simulink model "simulator_prototype"  (R2021b)
(part 7 of 12)

t5255 = t4765.*(-t1901+t3122+t3277);
t5262 = -t3893.*(t4165+t27.*(t1959-t3313+t38.*t1022.*(t855-t878).*2.196325630278387e-1));
t5280 = t3937.*t4834.*7.26735e-3;
t5281 = t4834.*(t1959-t3313+t38.*t1022.*(t855-t878).*2.196325630278387e-1).*(-7.26735e-3);
t5292 = -t5287;
t5300 = -t5297;
t5310 = t4118.*t4814;
t5320 = t4137+t4842;
t5321 = t4142+t4841;
t5356 = t4151.*t4853.*7.26735e-3;
t5357 = t4853.*(t1005+t20.*(t1941-t3315+t39.*t1022.*(t855-t878).*2.196325630278387e-1)).*(-7.26735e-3);
t5415 = (t4360.*t4879)./2.0;
et50 = -t2306-t2317+t3145+t3148+t35.*t941.*t948.*(t850-t874).*3.775747223193135e-1;
et51 = t36.*t941.*t948.*(t850-t874).*2.244797987218524e-1;
t5416 = ((et50+et51).*(-t3538+t3540+t50.*t188.*t202.*(t46-t47).*2.711709361697228e-39))./2.0;
t5487 = t3755.*t3910.*t3934.*t4172.*5.43845e-3;
t5488 = t3755.*t4172.*(t2674-t2676+t3022-t3027).*(t2694-t2701+t3036-t3043).*5.43845e-3;
t5494 = t3712.*t3910.*t3934.*t4215.*5.43845e-3;
t5495 = t3712.*t4215.*(t2674-t2676+t3022-t3027).*(t2694-t2701+t3036-t3043).*5.43845e-3;
t5535 = t3810.*t3910.*t3934.*t4172.*5.43845e-3;
t5536 = t3810.*t4172.*(t2674-t2676+t3022-t3027).*(t2694-t2701+t3036-t3043).*5.43845e-3;
t5538 = t3808.*t3910.*t3934.*t4215.*5.43845e-3;
t5539 = t3808.*t4215.*(t2674-t2676+t3022-t3027).*(t2694-t2701+t3036-t3043).*5.43845e-3;
t5543 = t3756+t4505+t4526;
t5728 = t3910.*t3934.*t3951.*(t1488+t1874+t2519+t2740+t2747+t3096+t3097).*(-3.633675e-3);
t5729 = t3951.*(t2674-t2676+t3022-t3027).*(t2694-t2701+t3036-t3043).*(t1488+t1874+t2519+t2740+t2747+t3096+t3097).*(-3.633675e-3);
t5730 = t3910.*t3934.*t3951.*(t1488+t1874+t2519+t2740+t2747+t3096+t3097).*3.633675e-3;
t5731 = t3951.*(t2674-t2676+t3022-t3027).*(t2694-t2701+t3036-t3043).*(t1488+t1874+t2519+t2740+t2747+t3096+t3097).*3.633675e-3;
t5732 = t3910.*t3925.*t3934.*(t1513+t1879+t2598+t2820+t2834+t3117+t3118).*(-3.633675e-3);
t5733 = t3925.*(t2674-t2676+t3022-t3027).*(t2694-t2701+t3036-t3043).*(t1513+t1879+t2598+t2820+t2834+t3117+t3118).*(-3.633675e-3);
t5734 = t3910.*t3925.*t3934.*(t1513+t1879+t2598+t2820+t2834+t3117+t3118).*3.633675e-3;
t5735 = t3925.*(t2674-t2676+t3022-t3027).*(t2694-t2701+t3036-t3043).*(t1513+t1879+t2598+t2820+t2834+t3117+t3118).*3.633675e-3;
t5738 = t3910.*t3934.*t4018.*(t1488+t1874+t2519+t2740+t2747+t3096+t3097).*(-3.633675e-3);
t5739 = t4018.*(t2674-t2676+t3022-t3027).*(t2694-t2701+t3036-t3043).*(t1488+t1874+t2519+t2740+t2747+t3096+t3097).*(-3.633675e-3);
t5741 = t3910.*t3934.*t3975.*(t1513+t1879+t2598+t2820+t2834+t3117+t3118).*(-3.633675e-3);
t5742 = t3975.*(t2674-t2676+t3022-t3027).*(t2694-t2701+t3036-t3043).*(t1513+t1879+t2598+t2820+t2834+t3117+t3118).*(-3.633675e-3);
t5758 = t3910.*t3934.*t4187.*(t1488+t1874+t2519+t2740+t2747+t3096+t3097).*(-3.633675e-3);
t5759 = t4187.*(t2674-t2676+t3022-t3027).*(t2694-t2701+t3036-t3043).*(t1488+t1874+t2519+t2740+t2747+t3096+t3097).*(-3.633675e-3);
t5780 = -t5779;
t5849 = t3934.*t4215.*t5278.*5.43845e-3;
t5850 = t4215.*t5279.*(t2694-t2701+t3036-t3043).*(-5.43845e-3);
t5916 = t4383+t4384+t4390+t4399;
t5917 = t4392+t4397+t4398+t4400;
t5952 = (t3910.*t4172.*t5540)./2.0;
t5953 = t4172.*t5541.*(t2674-t2676+t3022-t3027).*(-1.0./2.0);
t5955 = (t4172.*t5541.*(t2674-t2676+t3022-t3027))./2.0;
et52 = -t2748-t2749+t2773+t2781-t2788+t3211+t3471+t4032-t4047+t262.*(t46-t47).*2.075672598245148e-23;
et53 = t264.*(t46-t47).*1.875105520197095e-20;
t5989 = t3638.*t3910.*(et52+et53).*(-1.0./2.0);
et54 = t50.*t189.*(-t4504+t4515+t3395.*(t2813-t2835+t12.*(t1456-t2355).*1.02e-6+t17.*(t1456-t2355).*9.0e-8)+t3396.*(-t2804+t2838+t3109+t17.*(t1456-t2355).*9.3e-7));
et55 = -4.771516396025243e-17;
tau_c = ft_9({dq1,dq2,dq3,dq4,dq5,dq6,et54,et55,t10,t1005,t1022,t1089,t11,t1104,t1105,t1108,t1115,t1121,t1158,t1159,t1190,t1193,t1194,t1196,t12,t1205,t1207,t1208,t1210,t1212,t1214,t1217,t1218,t1219,t1220,t1221,t1222,t123,t1230,t1235,t1236,t1237,t1238,t1288,t1289,t13,t1302,t1303,t1319,t1320,t1336,t1348,t1350,t1351,t1360,t1369,t1378,t1396,t14,t140,t1425,t1435,t1456,t1477,t1488,t15,t1513,t1539,t1544,t1545,t1547,t1548,t1549,t1553,t1554,t1559,t1564,t1565,t1576,t1577,t1578,t1579,t1581,t1584,t1585,t1586,t1587,t1591,t1595,t1596,t1598,t1599,t16,t1600,t1601,t1602,t1604,t1605,t1606,t1607,t1608,t1609,t1612,t1613,t1614,t1615,t1616,t1626,t1627,t1628,t1629,t1631,t1637,t1640,t1641,t1648,t1649,t1659,t1660,t1661,t1666,t1667,t1683,t1686,t1690,t1692,t17,t1700,t1701,t1703,t1704,t1705,t1712,t1717,t1738,t1741,t1742,t1750,t1752,t1753,t1754,t1758,t1759,t1775,t1776,t18,t1861,t1874,t1879,t188,t1881,t189,t1896,t19,t1901,t1941,t1953,t1959,t1973,t1993,t1994,t20,t201,t202,t2023,t2053,t2060,t2089,t2090,t2098,t2099,t21,t2117,t2120,t2122,t2123,t2125,t2130,t2137,t2138,t2139,t2140,t2141,t2142,t2145,t2146,t2147,t2149,t2150,t2151,t2152,t2153,t2154,t2155,t2156,t2157,t2159,t2160,t2162,t2164,t2165,t2166,t2167,t2168,t2169,t2174,t2183,t2187,t2193,t2194,t2195,t2199,t22,t2203,t2215,t2219,t2222,t2223,t2239,t2240,t2256,t2257,t2291,t2292,t2293,t2294,t2295,t2296,t2297,t2298,t2299,t2300,t2301,t2302,t2303,t2304,t2306,t2307,t2308,t2309,t2310,t2311,t2313,t2317,t2320,t2322,t2323,t2324,t2325,t2326,t2327,t2328,t2329,t2337,t2338,t2339,t2341,t2342,t2343,t2344,t2352,t2353,t2354,t2355,t2357,t2358,t2359,t236,t2360,t2361,t2362,t2363,t2364,t2365,t2366,t2367,t2368,t2369,t237,t2370,t2371,t2374,t2375,t2378,t2379,t238,t2380,t2384,t2388,t2389,t2391,t2394,t2395,t2397,t2398,t2399,t24,t2400,t2401,t2402,t2403,t2404,t2405,t241,t2413,t2414,t2419,t2421,t2422,t2423,t2433,t2434,t2438,t2447,t2448,t2449,t2450,t2459,t2460,t2461,t2471,t2472,t2492,t2493,t2494,t25,t2502,t2508,t2509,t2510,t2515,t2519,t2520,t2525,t2527,t2529,t2530,t2532,t2534,t2539,t2555,t2556,t2572,t2575,t2583,t2598,t26,t2605,t2606,t2612,t2613,t2615,t2618,t2619,t262,t2638,t264,t2651,t2652,t2664,t2670,t2671,t2673,t2674,t2675,t2676,t2678,t2680,t2681,t2682,t2683,t2684,t2685,t2686,t2687,t2689,t2690,t2692,t2693,t2694,t2695,t2696,t2697,t2698,t27,t2700,t2701,t2704,t2705,t2707,t2708,t2709,t2711,t2712,t2713,t2715,t2716,t2717,t2719,t2720,t2721,t2733,t2735,t2736,t2740,t2742,t2744,t2745,t2747,t2748,t2749,t2750,t2753,t2754,t2759,t2765,t2769,t2773,t2774,t2775,t2777,t2778,t2779,t2781,t2785,t2786,t2787,t2788,t2790,t2792,t2795,t2797,t2798,t2799,t28,t2801,t2802,t2803,t2804,t2805,t2807,t2808,t2813,t2814,t2820,t2823,t2828,t2831,t2834,t2835,t2838,t2850,t2851,t29,t2927,t2937,t2941,t2942,t2945,t2946,t2947,t2948,t2950,t2951,t2953,t2954,t2955,t2956,t2957,t2962,t2963,t2964,t2965,t2966,t2969,t2970,t2971,t2972,t2973,t2975,t2976,t2977,t2978,t2979,t2982,t2984,t2985,t2986,t2987,t2990,t2991,t2993,t2994,t2998,t30,t3003,t3004,t3006,t3008,t3009,t3010,t3015,t3016,t3017,t3018,t3019,t3022,t3027,t3029,t3030,t3031,t3036,t3043,t3044,t3045,t3047,t3049,t3050,t3051,t3054,t3055,t3057,t3058,t3063,t3064,t3065,t3066,t3067,t3068,t3069,t3072,t3073,t3074,t3075,t3076,t3077,t3078,t3079,t3080,t3081,t3082,t3083,t3085,t3086,t3087,t3088,t3096,t3097,t31,t3109,t3117,t3118,t3119,t3121,t3122,t3126,t3129,t313,t3130,t3131,t3132,t3133,t3134,t3135,t3136,t314,t3140,t3141,t3142,t3143,t3145,t3148,t3150,t3151,t3153,t3154,t3155,t3156,t3157,t3158,t3159,t3160,t3161,t3162,t3163,t3164,t3165,t3166,t3167,t3171,t3172,t3173,t3179,t3180,t3181,t3185,t3187,t3188,t3189,t3190,t3192,t3193,t3194,t3195,t3196,t3198,t3199,t32,t3200,t3201,t3202,t3203,t3205,t3206,t3208,t3209,t321,t3211,t3212,t3213,t3216,t3217,t3219,t322,t3221,t3222,t3224,t3225,t3227,t3229,t3230,t3231,t3232,t3233,t3234,t3235,t3236,t3237,t3238,t3239,t3240,t3242,t3245,t3247,t3248,t3249,t3251,t3252,t3253,t3254,t3255,t3256,t3257,t3259,t326,t3260,t3261,t3263,t3265,t3266,t3267,t3268,t3269,t3270,t3271,t3272,t3273,t3276,t3277,t3278,t3279,t328,t3282,t3283,t3284,t3285,t3287,t3288,t3289,t329,t3290,t3291,t3292,t3294,t3295,t3296,t3297,t3298,t33,t330,t3300,t3301,t3303,t3304,t3307,t3308,t3309,t331,t3310,t3311,t3312,t3313,t3315,t3318,t332,t3322,t3324,t3326,t3328,t3329,t333,t3331,t3332,t3333,t3334,t3335,t3336,t3337,t3338,t3339,t3340,t3341,t3342,t3343,t3344,t3345,t3346,t3348,t3349,t335,t3351,t3352,t3353,t3354,t3356,t3357,t3358,t3359,t3360,t3361,t3362,t3363,t3364,t3365,t3366,t3369,t3370,t3377,t3379,t338,t3380,t3383,t3386,t3387,t3389,t339,t3392,t3393,t3394,t3395,t3396,t3397,t3398,t3399,t34,t3402,t3404,t3405,t3406,t3407,t3408,t3409,t341,t3410,t3411,t3416,t3418,t3419,t3420,t3421,t3422,t3423,t3426,t3428,t343,t3430,t3431,t3432,t3433,t3434,t3435,t3438,t3439,t3440,t3441,t3443,t3444,t3445,t3446,t3447,t3448,t3449,t3451,t3452,t3453,t3454,t3455,t3456,t3457,t3458,t346,t3460,t3461,t3462,t3463,t3464,t3465,t3467,t3468,t3469,t3470,t3471,t3472,t3474,t3475,t3478,t3480,t3481,t3483,t3488,t3489,t3490,t3492,t3495,t3496,t3498,t3499,t35,t350,t3500,t3502,t3503,t3504,t3505,t3506,t3507,t3508,t3509,t351,t3514,t3517,t352,t3524,t3530,t3538,t354,t3541,t3542,t3543,t3545,t3546,t3547,t3548,t3550,t3552,t3553,t3554,t3555,t3556,t3557,t356,t3560,t3566,t3571,t3577,t3578,t358,t3580,t3582,t3585,t3588,t359,t3590,t3597,t3598,t3599,t36,t360,t3600,t3602,t3605,t3609,t3611,t3616,t3619,t362,t3628,t363,t3638,t364,t3643,t3644,t3645,t3646,t3648,t3649,t365,t3651,t3655,t366,t3666,t3668,t3676,t3680,t3683,t3686,t369,t3690,t3692,t3693,t3695,t3696,t3697,t3699,t370,t3700,t3701,t3702,t3703,t3704,t3705,t3706,t3707,t3708,t3709,t371,t3710,t3711,t3712,t3713,t372,t3722,t3723,t3726,t3728,t3734,t3748,t3755,t3759,t3760,t3761,t3762,t3763,t3764,t3765,t3766,t3768,t3771,t3772,t3774,t3775,t3777,t3779,t378,t3781,t3782,t3783,t3784,t3785,t3786,t3788,t3789,t3790,t3791,t3792,t3793,t3794,t3795,t3796,t3797,t3798,t38,t380,t3800,t3801,t3802,t3804,t3805,t3808,t3809,t3810,t3811,t3812,t3813,t3814,t3815,t3816,t3817,t3818,t3819,t382,t3820,t3822,t3824,t3825,t3827,t3828,t3829,t3831,t3833,t3834,t3836,t3840,t3841,t3842,t3843,t3844,t3845,t3846,t3847,t3848,t3850,t3851,t3852,t3855,t3856,t3857,t3861,t3862,t3863,t3865,t387,t3871,t3872,t3873,t3874,t3876,t3877,t3878,t3879,t3880,t3881,t3882,t3883,t3884,t3885,t3887,t3888,t3893,t3894,t3895,t3896,t3897,t3898,t3899,t39,t3901,t3902,t3903,t3905,t3909,t3910,t3913,t3915,t3919,t3924,t3925,t3926,t3927,t3928,t3931,t3933,t3934,t3937,t3941,t3943,t3946,t3949,t3950,t3951,t3952,t3953,t3954,t3957,t3958,t3959,t3961,t3962,t3965,t3966,t3968,t3969,t3970,t3971,t3972,t3973,t3974,t3975,t3977,t3979,t3983,t3987,t3988,t3989,t3990,t3992,t3994,t3996,t3998,t3999,t4000,t4004,t4005,t4008,t4009,t4010,t4012,t4018,t4021,t4027,t4028,t4029,t4032,t4034,t4035,t4036,t4037,t4038,t4039,t4040,t4041,t4042,t4043,t4047,t4050,t4057,t4058,t4061,t4066,t4067,t4068,t4071,t4083,t4084,t4086,t4087,t4092,t4096,t4098,t410,t4101,t4118,t4125,t4126,t4144,t4145,t4146,t4147,t4149,t4151,t4153,t4154,t4160,t4163,t4165,t4167,t4169,t4171,t4172,t4176,t4177,t4181,t4182,t4187,t4192,t4195,t4196,t4198,t42,t4200,t4201,t4202,t4203,t4204,t4210,t4211,t4212,t4213,t4214,t4215,t4216,t4217,t4222,t4223,t4225,t4226,t4227,t4228,t4231,t4235,t4236,t4237,t4238,t4245,t4246,t4247,t4248,t4253,t4255,t4256,t4260,t4261,t4263,t4266,t4268,t4273,t4274,t4275,t4276,t4277,t4278,t4279,t4284,t4287,t4288,t429,t4293,t4294,t4295,t4297,t4298,t43,t4301,t4303,t4306,t4307,t4313,t4314,t4316,t4317,t4318,t4322,t4324,t4325,t4326,t4328,t4330,t4331,t4333,t4334,t4335,t4336,t4343,t4346,t4347,t4348,t4350,t4352,t4356,t4358,t4365,t4366,t4371,t4372,t4373,t4374,t4375,t4377,t4378,t4379,t4380,t4386,t4387,t4388,t4389,t4394,t4396,t4401,t4402,t4405,t4406,t4410,t4413,t4414,t4415,t4416,t4417,t4418,t4419,t4420,t4421,t4424,t4452,t4454,t4457,t4459,t4462,t4463,t4467,t4468,t4470,t4471,t4472,t4473,t4474,t4475,t4476,t4480,t4481,t4482,t4485,t4487,t4488,t4489,t4491,t4492,t4493,t4494,t4496,t4498,t4501,t4502,t4503,t4504,t4506,t4507,t4508,t4510,t4511,t4512,t4513,t4515,t4517,t4519,t4520,t4521,t4522,t4527,t4530,t4532,t4533,t4535,t4537,t4539,t4540,t4541,t4544,t4546,t4551,t4559,t4563,t46,t4636,t4637,t4644,t4650,t4652,t4654,t4657,t4663,t4665,t4667,t4670,t4673,t4674,t4677,t4678,t4680,t4683,t47,t4703,t4704,t4705,t4708,t4709,t4710,t4711,t4713,t4714,t4715,t4716,t4722,t4723,t4724,t4725,t4728,t4730,t4739,t4741,t4744,t4745,t4746,t4747,t4748,t4749,t4750,t4751,t4752,t4753,t4754,t4755,t4756,t4757,t4758,t4759,t4760,t4761,t4762,t4763,t4774,t4814,t4820,t4828,t4833,t4835,t4837,t4838,t4843,t4845,t4847,t4848,t4849,t4850,t4853,t4869,t4871,t4872,t4874,t4877,t4878,t4879,t4884,t4885,t4886,t4890,t4891,t4892,t4893,t4894,t4895,t4902,t4915,t4920,t4923,t4924,t4925,t4926,t50,t5014,t5015,t5016,t5017,t5025,t5027,t5028,t5036,t5037,t5045,t5046,t5052,t5053,t5059,t5062,t5063,t5066,t5070,t5072,t5075,t5079,t5084,t5085,t5086,t5087,t5088,t5089,t5090,t5091,t5092,t5093,t5094,t5095,t5096,t5097,t5098,t5099,t5108,t5111,t5194,t5195,t5203,t5209,t5217,t5218,t5219,t5240,t5250,t5252,t5255,t5262,t5274,t5276,t5278,t5279,t5280,t5281,t5283,t5285,t5286,t5287,t5289,t5291,t5292,t5295,t5296,t5297,t5300,t5301,t5302,t5303,t5304,t5308,t5309,t5310,t5312,t5320,t5321,t5356,t5357,t5361,t5363,t5370,t5372,t5381,t5391,t5392,t5393,t5395,t5399,t5400,t5401,t5402,t5403,t5404,t5415,t5416,t5433,t5434,t5436,t5437,t5438,t5439,t5452,t5456,t5457,t5458,t5459,t5460,t5464,t5481,t5487,t5488,t5494,t5495,t5499,t5535,t5536,t5537,t5538,t5539,t5540,t5541,t5542,t5543,t5544,t5545,t5548,t5550,t5561,t5569,t5570,t5586,t56,t5604,t5607,t5678,t5684,t5730,t5731,t5734,t5735,t5738,t5739,t5741,t5742,t5758,t5759,t5760,t5761,t5779,t5782,t5783,t58,t5849,t5896,t59,t5901,t5902,t5916,t5917,t5952,t5955,t5990,t60,t6011,t6013,t6014,t6255,t6256,t6257,t628,t635,t636,t638,t640,t641,t642,t643,t645,t646,t649,t654,t655,t656,t6564,t6565,t657,t659,t660,t6622,t6623,t663,t664,t665,t666,t667,t668,t669,t67,t670,t672,t673,t674,t6745,t675,t6751,t676,t677,t678,t679,t68,t681,t682,t683,t684,t685,t686,t687,t689,t691,t6919,t692,t6920,t693,t694,t6987,t70,t702,t707,t708,t71,t710,t715,t7150,t716,t717,t718,t721,t722,t724,t725,t73,t736,t738,t740,t741,t749,t756,t76,t762,t768,t777,t792,t793,t8,t801,t802,t808,t813,t819,t821,t850,t855,t874,t878,t89,t9,t90,t91,t92,t941,t944,t948,t951,t97});
end
function tau_c = ft_9(ct)
dq1 = ct{1};
dq2 = ct{2};
dq3 = ct{3};
dq4 = ct{4};
dq5 = ct{5};
dq6 = ct{6};
et54 = ct{7};
et55 = ct{8};
t10 = ct{9};
t1005 = ct{10};
t1022 = ct{11};
t1089 = ct{12};
t11 = ct{13};
t1104 = ct{14};
t1105 = ct{15};
t1108 = ct{16};
t1115 = ct{17};
t1121 = ct{18};
t1158 = ct{19};
t1159 = ct{20};
t1190 = ct{21};
t1193 = ct{22};
t1194 = ct{23};
t1196 = ct{24};
t12 = ct{25};
t1205 = ct{26};
t1207 = ct{27};
t1208 = ct{28};
t1210 = ct{29};
t1212 = ct{30};
t1214 = ct{31};
t1217 = ct{32};
t1218 = ct{33};
t1219 = ct{34};
t1220 = ct{35};
t1221 = ct{36};
t1222 = ct{37};
t123 = ct{38};
t1230 = ct{39};
t1235 = ct{40};
t1236 = ct{41};
t1237 = ct{42};
t1238 = ct{43};
t1288 = ct{44};
t1289 = ct{45};
t13 = ct{46};
t1302 = ct{47};
t1303 = ct{48};
t1319 = ct{49};
t1320 = ct{50};
t1336 = ct{51};
t1348 = ct{52};
t1350 = ct{53};
t1351 = ct{54};
t1360 = ct{55};
t1369 = ct{56};
t1378 = ct{57};
t1396 = ct{58};
t14 = ct{59};
t140 = ct{60};
t1425 = ct{61};
t1435 = ct{62};
t1456 = ct{63};
t1477 = ct{64};
t1488 = ct{65};
t15 = ct{66};
t1513 = ct{67};
t1539 = ct{68};
t1544 = ct{69};
t1545 = ct{70};
t1547 = ct{71};
t1548 = ct{72};
t1549 = ct{73};
t1553 = ct{74};
t1554 = ct{75};
t1559 = ct{76};
t1564 = ct{77};
t1565 = ct{78};
t1576 = ct{79};
t1577 = ct{80};
t1578 = ct{81};
t1579 = ct{82};
t1581 = ct{83};
t1584 = ct{84};
t1585 = ct{85};
t1586 = ct{86};
t1587 = ct{87};
t1591 = ct{88};
t1595 = ct{89};
t1596 = ct{90};
t1598 = ct{91};
t1599 = ct{92};
t16 = ct{93};
t1600 = ct{94};
t1601 = ct{95};
t1602 = ct{96};
t1604 = ct{97};
t1605 = ct{98};
t1606 = ct{99};
t1607 = ct{100};
t1608 = ct{101};
t1609 = ct{102};
t1612 = ct{103};
t1613 = ct{104};
t1614 = ct{105};
t1615 = ct{106};
t1616 = ct{107};
t1626 = ct{108};
t1627 = ct{109};
t1628 = ct{110};
t1629 = ct{111};
t1631 = ct{112};
t1637 = ct{113};
t1640 = ct{114};
t1641 = ct{115};
t1648 = ct{116};
t1649 = ct{117};
t1659 = ct{118};
t1660 = ct{119};
t1661 = ct{120};
t1666 = ct{121};
t1667 = ct{122};
t1683 = ct{123};
t1686 = ct{124};
t1690 = ct{125};
t1692 = ct{126};
t17 = ct{127};
t1700 = ct{128};
t1701 = ct{129};
t1703 = ct{130};
t1704 = ct{131};
t1705 = ct{132};
t1712 = ct{133};
t1717 = ct{134};
t1738 = ct{135};
t1741 = ct{136};
t1742 = ct{137};
t1750 = ct{138};
t1752 = ct{139};
t1753 = ct{140};
t1754 = ct{141};
t1758 = ct{142};
t1759 = ct{143};
t1775 = ct{144};
t1776 = ct{145};
t18 = ct{146};
t1861 = ct{147};
t1874 = ct{148};
t1879 = ct{149};
t188 = ct{150};
t1881 = ct{151};
t189 = ct{152};
t1896 = ct{153};
t19 = ct{154};
t1901 = ct{155};
t1941 = ct{156};
t1953 = ct{157};
t1959 = ct{158};
t1973 = ct{159};
t1993 = ct{160};
t1994 = ct{161};
t20 = ct{162};
t201 = ct{163};
t202 = ct{164};
t2023 = ct{165};
t2053 = ct{166};
t2060 = ct{167};
t2089 = ct{168};
t2090 = ct{169};
t2098 = ct{170};
t2099 = ct{171};
t21 = ct{172};
t2117 = ct{173};
t2120 = ct{174};
t2122 = ct{175};
t2123 = ct{176};
t2125 = ct{177};
t2130 = ct{178};
t2137 = ct{179};
t2138 = ct{180};
t2139 = ct{181};
t2140 = ct{182};
t2141 = ct{183};
t2142 = ct{184};
t2145 = ct{185};
t2146 = ct{186};
t2147 = ct{187};
t2149 = ct{188};
t2150 = ct{189};
t2151 = ct{190};
t2152 = ct{191};
t2153 = ct{192};
t2154 = ct{193};
t2155 = ct{194};
t2156 = ct{195};
t2157 = ct{196};
t2159 = ct{197};
t2160 = ct{198};
t2162 = ct{199};
t2164 = ct{200};
t2165 = ct{201};
t2166 = ct{202};
t2167 = ct{203};
t2168 = ct{204};
t2169 = ct{205};
t2174 = ct{206};
t2183 = ct{207};
t2187 = ct{208};
t2193 = ct{209};
t2194 = ct{210};
t2195 = ct{211};
t2199 = ct{212};
t22 = ct{213};
t2203 = ct{214};
t2215 = ct{215};
t2219 = ct{216};
t2222 = ct{217};
t2223 = ct{218};
t2239 = ct{219};
t2240 = ct{220};
t2256 = ct{221};
t2257 = ct{222};
t2291 = ct{223};
t2292 = ct{224};
t2293 = ct{225};
t2294 = ct{226};
t2295 = ct{227};
t2296 = ct{228};
t2297 = ct{229};
t2298 = ct{230};
t2299 = ct{231};
t2300 = ct{232};
t2301 = ct{233};
t2302 = ct{234};
t2303 = ct{235};
t2304 = ct{236};
t2306 = ct{237};
t2307 = ct{238};
t2308 = ct{239};
t2309 = ct{240};
t2310 = ct{241};
t2311 = ct{242};
t2313 = ct{243};
t2317 = ct{244};
t2320 = ct{245};
t2322 = ct{246};
t2323 = ct{247};
t2324 = ct{248};
t2325 = ct{249};
t2326 = ct{250};
t2327 = ct{251};
t2328 = ct{252};
t2329 = ct{253};
t2337 = ct{254};
t2338 = ct{255};
t2339 = ct{256};
t2341 = ct{257};
t2342 = ct{258};
t2343 = ct{259};
t2344 = ct{260};
t2352 = ct{261};
t2353 = ct{262};
t2354 = ct{263};
t2355 = ct{264};
t2357 = ct{265};
t2358 = ct{266};
t2359 = ct{267};
t236 = ct{268};
t2360 = ct{269};
t2361 = ct{270};
t2362 = ct{271};
t2363 = ct{272};
t2364 = ct{273};
t2365 = ct{274};
t2366 = ct{275};
t2367 = ct{276};
t2368 = ct{277};
t2369 = ct{278};
t237 = ct{279};
t2370 = ct{280};
t2371 = ct{281};
t2374 = ct{282};
t2375 = ct{283};
t2378 = ct{284};
t2379 = ct{285};
t238 = ct{286};
t2380 = ct{287};
t2384 = ct{288};
t2388 = ct{289};
t2389 = ct{290};
t2391 = ct{291};
t2394 = ct{292};
t2395 = ct{293};
t2397 = ct{294};
t2398 = ct{295};
t2399 = ct{296};
t24 = ct{297};
t2400 = ct{298};
t2401 = ct{299};
t2402 = ct{300};
t2403 = ct{301};
t2404 = ct{302};
t2405 = ct{303};
t241 = ct{304};
t2413 = ct{305};
t2414 = ct{306};
t2419 = ct{307};
t2421 = ct{308};
t2422 = ct{309};
t2423 = ct{310};
t2433 = ct{311};
t2434 = ct{312};
t2438 = ct{313};
t2447 = ct{314};
t2448 = ct{315};
t2449 = ct{316};
t2450 = ct{317};
t2459 = ct{318};
t2460 = ct{319};
t2461 = ct{320};
t2471 = ct{321};
t2472 = ct{322};
t2492 = ct{323};
t2493 = ct{324};
t2494 = ct{325};
t25 = ct{326};
t2502 = ct{327};
t2508 = ct{328};
t2509 = ct{329};
t2510 = ct{330};
t2515 = ct{331};
t2519 = ct{332};
t2520 = ct{333};
t2525 = ct{334};
t2527 = ct{335};
t2529 = ct{336};
t2530 = ct{337};
t2532 = ct{338};
t2534 = ct{339};
t2539 = ct{340};
t2555 = ct{341};
t2556 = ct{342};
t2572 = ct{343};
t2575 = ct{344};
t2583 = ct{345};
t2598 = ct{346};
t26 = ct{347};
t2605 = ct{348};
t2606 = ct{349};
t2612 = ct{350};
t2613 = ct{351};
t2615 = ct{352};
t2618 = ct{353};
t2619 = ct{354};
t262 = ct{355};
t2638 = ct{356};
t264 = ct{357};
t2651 = ct{358};
t2652 = ct{359};
t2664 = ct{360};
t2670 = ct{361};
t2671 = ct{362};
t2673 = ct{363};
t2674 = ct{364};
t2675 = ct{365};
t2676 = ct{366};
t2678 = ct{367};
t2680 = ct{368};
t2681 = ct{369};
t2682 = ct{370};
t2683 = ct{371};
t2684 = ct{372};
t2685 = ct{373};
t2686 = ct{374};
t2687 = ct{375};
t2689 = ct{376};
t2690 = ct{377};
t2692 = ct{378};
t2693 = ct{379};
t2694 = ct{380};
t2695 = ct{381};
t2696 = ct{382};
t2697 = ct{383};
t2698 = ct{384};
t27 = ct{385};
t2700 = ct{386};
t2701 = ct{387};
t2704 = ct{388};
t2705 = ct{389};
t2707 = ct{390};
t2708 = ct{391};
t2709 = ct{392};
t2711 = ct{393};
t2712 = ct{394};
t2713 = ct{395};
t2715 = ct{396};
t2716 = ct{397};
t2717 = ct{398};
t2719 = ct{399};
t2720 = ct{400};
t2721 = ct{401};
t2733 = ct{402};
t2735 = ct{403};
t2736 = ct{404};
t2740 = ct{405};
t2742 = ct{406};
t2744 = ct{407};
t2745 = ct{408};
t2747 = ct{409};
t2748 = ct{410};
t2749 = ct{411};
t2750 = ct{412};
t2753 = ct{413};
t2754 = ct{414};
t2759 = ct{415};
t2765 = ct{416};
t2769 = ct{417};
t2773 = ct{418};
t2774 = ct{419};
t2775 = ct{420};
t2777 = ct{421};
t2778 = ct{422};
t2779 = ct{423};
t2781 = ct{424};
t2785 = ct{425};
t2786 = ct{426};
t2787 = ct{427};
t2788 = ct{428};
t2790 = ct{429};
t2792 = ct{430};
t2795 = ct{431};
t2797 = ct{432};
t2798 = ct{433};
t2799 = ct{434};
t28 = ct{435};
t2801 = ct{436};
t2802 = ct{437};
t2803 = ct{438};
t2804 = ct{439};
t2805 = ct{440};
t2807 = ct{441};
t2808 = ct{442};
t2813 = ct{443};
t2814 = ct{444};
t2820 = ct{445};
t2823 = ct{446};
t2828 = ct{447};
t2831 = ct{448};
t2834 = ct{449};
t2835 = ct{450};
t2838 = ct{451};
t2850 = ct{452};
t2851 = ct{453};
t29 = ct{454};
t2927 = ct{455};
t2937 = ct{456};
t2941 = ct{457};
t2942 = ct{458};
t2945 = ct{459};
t2946 = ct{460};
t2947 = ct{461};
t2948 = ct{462};
t2950 = ct{463};
t2951 = ct{464};
t2953 = ct{465};
t2954 = ct{466};
t2955 = ct{467};
t2956 = ct{468};
t2957 = ct{469};
t2962 = ct{470};
t2963 = ct{471};
t2964 = ct{472};
t2965 = ct{473};
t2966 = ct{474};
t2969 = ct{475};
t2970 = ct{476};
t2971 = ct{477};
t2972 = ct{478};
t2973 = ct{479};
t2975 = ct{480};
t2976 = ct{481};
t2977 = ct{482};
t2978 = ct{483};
t2979 = ct{484};
t2982 = ct{485};
t2984 = ct{486};
t2985 = ct{487};
t2986 = ct{488};
t2987 = ct{489};
t2990 = ct{490};
t2991 = ct{491};
t2993 = ct{492};
t2994 = ct{493};
t2998 = ct{494};
t30 = ct{495};
t3003 = ct{496};
t3004 = ct{497};
t3006 = ct{498};
t3008 = ct{499};
t3009 = ct{500};
t3010 = ct{501};
t3015 = ct{502};
t3016 = ct{503};
t3017 = ct{504};
t3018 = ct{505};
t3019 = ct{506};
t3022 = ct{507};
t3027 = ct{508};
t3029 = ct{509};
t3030 = ct{510};
t3031 = ct{511};
t3036 = ct{512};
t3043 = ct{513};
t3044 = ct{514};
t3045 = ct{515};
t3047 = ct{516};
t3049 = ct{517};
t3050 = ct{518};
t3051 = ct{519};
t3054 = ct{520};
t3055 = ct{521};
t3057 = ct{522};
t3058 = ct{523};
t3063 = ct{524};
t3064 = ct{525};
t3065 = ct{526};
t3066 = ct{527};
t3067 = ct{528};
t3068 = ct{529};
t3069 = ct{530};
t3072 = ct{531};
t3073 = ct{532};
t3074 = ct{533};
t3075 = ct{534};
t3076 = ct{535};
t3077 = ct{536};
t3078 = ct{537};
t3079 = ct{538};
t3080 = ct{539};
t3081 = ct{540};
t3082 = ct{541};
t3083 = ct{542};
t3085 = ct{543};
t3086 = ct{544};
t3087 = ct{545};
t3088 = ct{546};
t3096 = ct{547};
t3097 = ct{548};
t31 = ct{549};
t3109 = ct{550};
t3117 = ct{551};
t3118 = ct{552};
t3119 = ct{553};
t3121 = ct{554};
t3122 = ct{555};
t3126 = ct{556};
t3129 = ct{557};
t313 = ct{558};
t3130 = ct{559};
t3131 = ct{560};
t3132 = ct{561};
t3133 = ct{562};
t3134 = ct{563};
t3135 = ct{564};
t3136 = ct{565};
t314 = ct{566};
t3140 = ct{567};
t3141 = ct{568};
t3142 = ct{569};
t3143 = ct{570};
t3145 = ct{571};
t3148 = ct{572};
t3150 = ct{573};
t3151 = ct{574};
t3153 = ct{575};
t3154 = ct{576};
t3155 = ct{577};
t3156 = ct{578};
t3157 = ct{579};
t3158 = ct{580};
t3159 = ct{581};
t3160 = ct{582};
t3161 = ct{583};
t3162 = ct{584};
t3163 = ct{585};
t3164 = ct{586};
t3165 = ct{587};
t3166 = ct{588};
t3167 = ct{589};
t3171 = ct{590};
t3172 = ct{591};
t3173 = ct{592};
t3179 = ct{593};
t3180 = ct{594};
t3181 = ct{595};
t3185 = ct{596};
t3187 = ct{597};
t3188 = ct{598};
t3189 = ct{599};
t3190 = ct{600};
t3192 = ct{601};
t3193 = ct{602};
t3194 = ct{603};
t3195 = ct{604};
t3196 = ct{605};
t3198 = ct{606};
t3199 = ct{607};
t32 = ct{608};
t3200 = ct{609};
t3201 = ct{610};
t3202 = ct{611};
t3203 = ct{612};
t3205 = ct{613};
t3206 = ct{614};
t3208 = ct{615};
t3209 = ct{616};
t321 = ct{617};
t3211 = ct{618};
t3212 = ct{619};
t3213 = ct{620};
t3216 = ct{621};
t3217 = ct{622};
t3219 = ct{623};
t322 = ct{624};
t3221 = ct{625};
t3222 = ct{626};
t3224 = ct{627};
t3225 = ct{628};
t3227 = ct{629};
t3229 = ct{630};
t3230 = ct{631};
t3231 = ct{632};
t3232 = ct{633};
t3233 = ct{634};
t3234 = ct{635};
t3235 = ct{636};
t3236 = ct{637};
t3237 = ct{638};
t3238 = ct{639};
t3239 = ct{640};
t3240 = ct{641};
t3242 = ct{642};
t3245 = ct{643};
t3247 = ct{644};
t3248 = ct{645};
t3249 = ct{646};
t3251 = ct{647};
t3252 = ct{648};
t3253 = ct{649};
t3254 = ct{650};
t3255 = ct{651};
t3256 = ct{652};
t3257 = ct{653};
t3259 = ct{654};
t326 = ct{655};
t3260 = ct{656};
t3261 = ct{657};
t3263 = ct{658};
t3265 = ct{659};
t3266 = ct{660};
t3267 = ct{661};
t3268 = ct{662};
t3269 = ct{663};
t3270 = ct{664};
t3271 = ct{665};
t3272 = ct{666};
t3273 = ct{667};
t3276 = ct{668};
t3277 = ct{669};
t3278 = ct{670};
t3279 = ct{671};
t328 = ct{672};
t3282 = ct{673};
t3283 = ct{674};
t3284 = ct{675};
t3285 = ct{676};
t3287 = ct{677};
t3288 = ct{678};
t3289 = ct{679};
t329 = ct{680};
t3290 = ct{681};
t3291 = ct{682};
t3292 = ct{683};
t3294 = ct{684};
t3295 = ct{685};
t3296 = ct{686};
t3297 = ct{687};
t3298 = ct{688};
t33 = ct{689};
t330 = ct{690};
t3300 = ct{691};
t3301 = ct{692};
t3303 = ct{693};
t3304 = ct{694};
t3307 = ct{695};
t3308 = ct{696};
t3309 = ct{697};
t331 = ct{698};
t3310 = ct{699};
t3311 = ct{700};
t3312 = ct{701};
t3313 = ct{702};
t3315 = ct{703};
t3318 = ct{704};
t332 = ct{705};
t3322 = ct{706};
t3324 = ct{707};
t3326 = ct{708};
t3328 = ct{709};
t3329 = ct{710};
t333 = ct{711};
t3331 = ct{712};
t3332 = ct{713};
t3333 = ct{714};
t3334 = ct{715};
t3335 = ct{716};
t3336 = ct{717};
t3337 = ct{718};
t3338 = ct{719};
t3339 = ct{720};
t3340 = ct{721};
t3341 = ct{722};
t3342 = ct{723};
t3343 = ct{724};
t3344 = ct{725};
t3345 = ct{726};
t3346 = ct{727};
t3348 = ct{728};
t3349 = ct{729};
t335 = ct{730};
t3351 = ct{731};
t3352 = ct{732};
t3353 = ct{733};
t3354 = ct{734};
t3356 = ct{735};
t3357 = ct{736};
t3358 = ct{737};
t3359 = ct{738};
t3360 = ct{739};
t3361 = ct{740};
t3362 = ct{741};
t3363 = ct{742};
t3364 = ct{743};
t3365 = ct{744};
t3366 = ct{745};
t3369 = ct{746};
t3370 = ct{747};
t3377 = ct{748};
t3379 = ct{749};
t338 = ct{750};
t3380 = ct{751};
t3383 = ct{752};
t3386 = ct{753};
t3387 = ct{754};
t3389 = ct{755};
t339 = ct{756};
t3392 = ct{757};
t3393 = ct{758};
t3394 = ct{759};
t3395 = ct{760};
t3396 = ct{761};
t3397 = ct{762};
t3398 = ct{763};
t3399 = ct{764};
t34 = ct{765};
t3402 = ct{766};
t3404 = ct{767};
t3405 = ct{768};
t3406 = ct{769};
t3407 = ct{770};
t3408 = ct{771};
t3409 = ct{772};
t341 = ct{773};
t3410 = ct{774};
t3411 = ct{775};
t3416 = ct{776};
t3418 = ct{777};
t3419 = ct{778};
t3420 = ct{779};
t3421 = ct{780};
t3422 = ct{781};
t3423 = ct{782};
t3426 = ct{783};
t3428 = ct{784};
t343 = ct{785};
t3430 = ct{786};
t3431 = ct{787};
t3432 = ct{788};
t3433 = ct{789};
t3434 = ct{790};
t3435 = ct{791};
t3438 = ct{792};
t3439 = ct{793};
t3440 = ct{794};
t3441 = ct{795};
t3443 = ct{796};
t3444 = ct{797};
t3445 = ct{798};
t3446 = ct{799};
t3447 = ct{800};
t3448 = ct{801};
t3449 = ct{802};
t3451 = ct{803};
t3452 = ct{804};
t3453 = ct{805};
t3454 = ct{806};
t3455 = ct{807};
t3456 = ct{808};
t3457 = ct{809};
t3458 = ct{810};
t346 = ct{811};
t3460 = ct{812};
t3461 = ct{813};
t3462 = ct{814};
t3463 = ct{815};
t3464 = ct{816};
t3465 = ct{817};
t3467 = ct{818};
t3468 = ct{819};
t3469 = ct{820};
t3470 = ct{821};
t3471 = ct{822};
t3472 = ct{823};
t3474 = ct{824};
t3475 = ct{825};
t3478 = ct{826};
t3480 = ct{827};
t3481 = ct{828};
t3483 = ct{829};
t3488 = ct{830};
t3489 = ct{831};
t3490 = ct{832};
t3492 = ct{833};
t3495 = ct{834};
t3496 = ct{835};
t3498 = ct{836};
t3499 = ct{837};
t35 = ct{838};
t350 = ct{839};
t3500 = ct{840};
t3502 = ct{841};
t3503 = ct{842};
t3504 = ct{843};
t3505 = ct{844};
t3506 = ct{845};
t3507 = ct{846};
t3508 = ct{847};
t3509 = ct{848};
t351 = ct{849};
t3514 = ct{850};
t3517 = ct{851};
t352 = ct{852};
t3524 = ct{853};
t3530 = ct{854};
t3538 = ct{855};
t354 = ct{856};
t3541 = ct{857};
t3542 = ct{858};
t3543 = ct{859};
t3545 = ct{860};
t3546 = ct{861};
t3547 = ct{862};
t3548 = ct{863};
t3550 = ct{864};
t3552 = ct{865};
t3553 = ct{866};
t3554 = ct{867};
t3555 = ct{868};
t3556 = ct{869};
t3557 = ct{870};
t356 = ct{871};
t3560 = ct{872};
t3566 = ct{873};
t3571 = ct{874};
t3577 = ct{875};
t3578 = ct{876};
t358 = ct{877};
t3580 = ct{878};
t3582 = ct{879};
t3585 = ct{880};
t3588 = ct{881};
t359 = ct{882};
t3590 = ct{883};
t3597 = ct{884};
t3598 = ct{885};
t3599 = ct{886};
t36 = ct{887};
t360 = ct{888};
t3600 = ct{889};
t3602 = ct{890};
t3605 = ct{891};
t3609 = ct{892};
t3611 = ct{893};
t3616 = ct{894};
t3619 = ct{895};
t362 = ct{896};
t3628 = ct{897};
t363 = ct{898};
t3638 = ct{899};
t364 = ct{900};
t3643 = ct{901};
t3644 = ct{902};
t3645 = ct{903};
t3646 = ct{904};
t3648 = ct{905};
t3649 = ct{906};
t365 = ct{907};
t3651 = ct{908};
t3655 = ct{909};
t366 = ct{910};
t3666 = ct{911};
t3668 = ct{912};
t3676 = ct{913};
t3680 = ct{914};
t3683 = ct{915};
t3686 = ct{916};
t369 = ct{917};
t3690 = ct{918};
t3692 = ct{919};
t3693 = ct{920};
t3695 = ct{921};
t3696 = ct{922};
t3697 = ct{923};
t3699 = ct{924};
t370 = ct{925};
t3700 = ct{926};
t3701 = ct{927};
t3702 = ct{928};
t3703 = ct{929};
t3704 = ct{930};
t3705 = ct{931};
t3706 = ct{932};
t3707 = ct{933};
t3708 = ct{934};
t3709 = ct{935};
t371 = ct{936};
t3710 = ct{937};
t3711 = ct{938};
t3712 = ct{939};
t3713 = ct{940};
t372 = ct{941};
t3722 = ct{942};
t3723 = ct{943};
t3726 = ct{944};
t3728 = ct{945};
t3734 = ct{946};
t3748 = ct{947};
t3755 = ct{948};
t3759 = ct{949};
t3760 = ct{950};
t3761 = ct{951};
t3762 = ct{952};
t3763 = ct{953};
t3764 = ct{954};
t3765 = ct{955};
t3766 = ct{956};
t3768 = ct{957};
t3771 = ct{958};
t3772 = ct{959};
t3774 = ct{960};
t3775 = ct{961};
t3777 = ct{962};
t3779 = ct{963};
t378 = ct{964};
t3781 = ct{965};
t3782 = ct{966};
t3783 = ct{967};
t3784 = ct{968};
t3785 = ct{969};
t3786 = ct{970};
t3788 = ct{971};
t3789 = ct{972};
t3790 = ct{973};
t3791 = ct{974};
t3792 = ct{975};
t3793 = ct{976};
t3794 = ct{977};
t3795 = ct{978};
t3796 = ct{979};
t3797 = ct{980};
t3798 = ct{981};
t38 = ct{982};
t380 = ct{983};
t3800 = ct{984};
t3801 = ct{985};
t3802 = ct{986};
t3804 = ct{987};
t3805 = ct{988};
t3808 = ct{989};
t3809 = ct{990};
t3810 = ct{991};
t3811 = ct{992};
t3812 = ct{993};
t3813 = ct{994};
t3814 = ct{995};
t3815 = ct{996};
t3816 = ct{997};
t3817 = ct{998};
t3818 = ct{999};
t3819 = ct{1000};
t382 = ct{1001};
t3820 = ct{1002};
t3822 = ct{1003};
t3824 = ct{1004};
t3825 = ct{1005};
t3827 = ct{1006};
t3828 = ct{1007};
t3829 = ct{1008};
t3831 = ct{1009};
t3833 = ct{1010};
t3834 = ct{1011};
t3836 = ct{1012};
t3840 = ct{1013};
t3841 = ct{1014};
t3842 = ct{1015};
t3843 = ct{1016};
t3844 = ct{1017};
t3845 = ct{1018};
t3846 = ct{1019};
t3847 = ct{1020};
t3848 = ct{1021};
t3850 = ct{1022};
t3851 = ct{1023};
t3852 = ct{1024};
t3855 = ct{1025};
t3856 = ct{1026};
t3857 = ct{1027};
t3861 = ct{1028};
t3862 = ct{1029};
t3863 = ct{1030};
t3865 = ct{1031};
t387 = ct{1032};
t3871 = ct{1033};
t3872 = ct{1034};
t3873 = ct{1035};
t3874 = ct{1036};
t3876 = ct{1037};
t3877 = ct{1038};
t3878 = ct{1039};
t3879 = ct{1040};
t3880 = ct{1041};
t3881 = ct{1042};
t3882 = ct{1043};
t3883 = ct{1044};
t3884 = ct{1045};
t3885 = ct{1046};
t3887 = ct{1047};
t3888 = ct{1048};
t3893 = ct{1049};
t3894 = ct{1050};
t3895 = ct{1051};
t3896 = ct{1052};
t3897 = ct{1053};
t3898 = ct{1054};
t3899 = ct{1055};
t39 = ct{1056};
t3901 = ct{1057};
t3902 = ct{1058};
t3903 = ct{1059};
t3905 = ct{1060};
t3909 = ct{1061};
t3910 = ct{1062};
t3913 = ct{1063};
t3915 = ct{1064};
t3919 = ct{1065};
t3924 = ct{1066};
t3925 = ct{1067};
t3926 = ct{1068};
t3927 = ct{1069};
t3928 = ct{1070};
t3931 = ct{1071};
t3933 = ct{1072};
t3934 = ct{1073};
t3937 = ct{1074};
t3941 = ct{1075};
t3943 = ct{1076};
t3946 = ct{1077};
t3949 = ct{1078};
t3950 = ct{1079};
t3951 = ct{1080};
t3952 = ct{1081};
t3953 = ct{1082};
t3954 = ct{1083};
t3957 = ct{1084};
t3958 = ct{1085};
t3959 = ct{1086};
t3961 = ct{1087};
t3962 = ct{1088};
t3965 = ct{1089};
t3966 = ct{1090};
t3968 = ct{1091};
t3969 = ct{1092};
t3970 = ct{1093};
t3971 = ct{1094};
t3972 = ct{1095};
t3973 = ct{1096};
t3974 = ct{1097};
t3975 = ct{1098};
t3977 = ct{1099};
t3979 = ct{1100};
t3983 = ct{1101};
t3987 = ct{1102};
t3988 = ct{1103};
t3989 = ct{1104};
t3990 = ct{1105};
t3992 = ct{1106};
t3994 = ct{1107};
t3996 = ct{1108};
t3998 = ct{1109};
t3999 = ct{1110};
t4000 = ct{1111};
t4004 = ct{1112};
t4005 = ct{1113};
t4008 = ct{1114};
t4009 = ct{1115};
t4010 = ct{1116};
t4012 = ct{1117};
t4018 = ct{1118};
t4021 = ct{1119};
t4027 = ct{1120};
t4028 = ct{1121};
t4029 = ct{1122};
t4032 = ct{1123};
t4034 = ct{1124};
t4035 = ct{1125};
t4036 = ct{1126};
t4037 = ct{1127};
t4038 = ct{1128};
t4039 = ct{1129};
t4040 = ct{1130};
t4041 = ct{1131};
t4042 = ct{1132};
t4043 = ct{1133};
t4047 = ct{1134};
t4050 = ct{1135};
t4057 = ct{1136};
t4058 = ct{1137};
t4061 = ct{1138};
t4066 = ct{1139};
t4067 = ct{1140};
t4068 = ct{1141};
t4071 = ct{1142};
t4083 = ct{1143};
t4084 = ct{1144};
t4086 = ct{1145};
t4087 = ct{1146};
t4092 = ct{1147};
t4096 = ct{1148};
t4098 = ct{1149};
t410 = ct{1150};
t4101 = ct{1151};
t4118 = ct{1152};
t4125 = ct{1153};
t4126 = ct{1154};
t4144 = ct{1155};
t4145 = ct{1156};
t4146 = ct{1157};
t4147 = ct{1158};
t4149 = ct{1159};
t4151 = ct{1160};
t4153 = ct{1161};
t4154 = ct{1162};
t4160 = ct{1163};
t4163 = ct{1164};
t4165 = ct{1165};
t4167 = ct{1166};
t4169 = ct{1167};
t4171 = ct{1168};
t4172 = ct{1169};
t4176 = ct{1170};
t4177 = ct{1171};
t4181 = ct{1172};
t4182 = ct{1173};
t4187 = ct{1174};
t4192 = ct{1175};
t4195 = ct{1176};
t4196 = ct{1177};
t4198 = ct{1178};
t42 = ct{1179};
t4200 = ct{1180};
t4201 = ct{1181};
t4202 = ct{1182};
t4203 = ct{1183};
t4204 = ct{1184};
t4210 = ct{1185};
t4211 = ct{1186};
t4212 = ct{1187};
t4213 = ct{1188};
t4214 = ct{1189};
t4215 = ct{1190};
t4216 = ct{1191};
t4217 = ct{1192};
t4222 = ct{1193};
t4223 = ct{1194};
t4225 = ct{1195};
t4226 = ct{1196};
t4227 = ct{1197};
t4228 = ct{1198};
t4231 = ct{1199};
t4235 = ct{1200};
t4236 = ct{1201};
t4237 = ct{1202};
t4238 = ct{1203};
t4245 = ct{1204};
t4246 = ct{1205};
t4247 = ct{1206};
t4248 = ct{1207};
t4253 = ct{1208};
t4255 = ct{1209};
t4256 = ct{1210};
t4260 = ct{1211};
t4261 = ct{1212};
t4263 = ct{1213};
t4266 = ct{1214};
t4268 = ct{1215};
t4273 = ct{1216};
t4274 = ct{1217};
t4275 = ct{1218};
t4276 = ct{1219};
t4277 = ct{1220};
t4278 = ct{1221};
t4279 = ct{1222};
t4284 = ct{1223};
t4287 = ct{1224};
t4288 = ct{1225};
t429 = ct{1226};
t4293 = ct{1227};
t4294 = ct{1228};
t4295 = ct{1229};
t4297 = ct{1230};
t4298 = ct{1231};
t43 = ct{1232};
t4301 = ct{1233};
t4303 = ct{1234};
t4306 = ct{1235};
t4307 = ct{1236};
t4313 = ct{1237};
t4314 = ct{1238};
t4316 = ct{1239};
t4317 = ct{1240};
t4318 = ct{1241};
t4322 = ct{1242};
t4324 = ct{1243};
t4325 = ct{1244};
t4326 = ct{1245};
t4328 = ct{1246};
t4330 = ct{1247};
t4331 = ct{1248};
t4333 = ct{1249};
t4334 = ct{1250};
t4335 = ct{1251};
t4336 = ct{1252};
t4343 = ct{1253};
t4346 = ct{1254};
t4347 = ct{1255};
t4348 = ct{1256};
t4350 = ct{1257};
t4352 = ct{1258};
t4356 = ct{1259};
t4358 = ct{1260};
t4365 = ct{1261};
t4366 = ct{1262};
t4371 = ct{1263};
t4372 = ct{1264};
t4373 = ct{1265};
t4374 = ct{1266};
t4375 = ct{1267};
t4377 = ct{1268};
t4378 = ct{1269};
t4379 = ct{1270};
t4380 = ct{1271};
t4386 = ct{1272};
t4387 = ct{1273};
t4388 = ct{1274};
t4389 = ct{1275};
t4394 = ct{1276};
t4396 = ct{1277};
t4401 = ct{1278};
t4402 = ct{1279};
t4405 = ct{1280};
t4406 = ct{1281};
t4410 = ct{1282};
t4413 = ct{1283};
t4414 = ct{1284};
t4415 = ct{1285};
t4416 = ct{1286};
t4417 = ct{1287};
t4418 = ct{1288};
t4419 = ct{1289};
t4420 = ct{1290};
t4421 = ct{1291};
t4424 = ct{1292};
t4452 = ct{1293};
t4454 = ct{1294};
t4457 = ct{1295};
t4459 = ct{1296};
t4462 = ct{1297};
t4463 = ct{1298};
t4467 = ct{1299};
t4468 = ct{1300};
t4470 = ct{1301};
t4471 = ct{1302};
t4472 = ct{1303};
t4473 = ct{1304};
t4474 = ct{1305};
t4475 = ct{1306};
t4476 = ct{1307};
t4480 = ct{1308};
t4481 = ct{1309};
t4482 = ct{1310};
t4485 = ct{1311};
t4487 = ct{1312};
t4488 = ct{1313};
t4489 = ct{1314};
t4491 = ct{1315};
t4492 = ct{1316};
t4493 = ct{1317};
t4494 = ct{1318};
t4496 = ct{1319};
t4498 = ct{1320};
t4501 = ct{1321};
t4502 = ct{1322};
t4503 = ct{1323};
t4504 = ct{1324};
t4506 = ct{1325};
t4507 = ct{1326};
t4508 = ct{1327};
t4510 = ct{1328};
t4511 = ct{1329};
t4512 = ct{1330};
t4513 = ct{1331};
t4515 = ct{1332};
t4517 = ct{1333};
t4519 = ct{1334};
t4520 = ct{1335};
t4521 = ct{1336};
t4522 = ct{1337};
t4527 = ct{1338};
t4530 = ct{1339};
t4532 = ct{1340};
t4533 = ct{1341};
t4535 = ct{1342};
t4537 = ct{1343};
t4539 = ct{1344};
t4540 = ct{1345};
t4541 = ct{1346};
t4544 = ct{1347};
t4546 = ct{1348};
t4551 = ct{1349};
t4559 = ct{1350};
t4563 = ct{1351};
t46 = ct{1352};
t4636 = ct{1353};
t4637 = ct{1354};
t4644 = ct{1355};
t4650 = ct{1356};
t4652 = ct{1357};
t4654 = ct{1358};
t4657 = ct{1359};
t4663 = ct{1360};
t4665 = ct{1361};
t4667 = ct{1362};
t4670 = ct{1363};
t4673 = ct{1364};
t4674 = ct{1365};
t4677 = ct{1366};
t4678 = ct{1367};
t4680 = ct{1368};
t4683 = ct{1369};
t47 = ct{1370};
t4703 = ct{1371};
t4704 = ct{1372};
t4705 = ct{1373};
t4708 = ct{1374};
t4709 = ct{1375};
t4710 = ct{1376};
t4711 = ct{1377};
t4713 = ct{1378};
t4714 = ct{1379};
t4715 = ct{1380};
t4716 = ct{1381};
t4722 = ct{1382};
t4723 = ct{1383};
t4724 = ct{1384};
t4725 = ct{1385};
t4728 = ct{1386};
t4730 = ct{1387};
t4739 = ct{1388};
t4741 = ct{1389};
t4744 = ct{1390};
t4745 = ct{1391};
t4746 = ct{1392};
t4747 = ct{1393};
t4748 = ct{1394};
t4749 = ct{1395};
t4750 = ct{1396};
t4751 = ct{1397};
t4752 = ct{1398};
t4753 = ct{1399};
t4754 = ct{1400};
t4755 = ct{1401};
t4756 = ct{1402};
t4757 = ct{1403};
t4758 = ct{1404};
t4759 = ct{1405};
t4760 = ct{1406};
t4761 = ct{1407};
t4762 = ct{1408};
t4763 = ct{1409};
t4774 = ct{1410};
t4814 = ct{1411};
t4820 = ct{1412};
t4828 = ct{1413};
t4833 = ct{1414};
t4835 = ct{1415};
t4837 = ct{1416};
t4838 = ct{1417};
t4843 = ct{1418};
t4845 = ct{1419};
t4847 = ct{1420};
t4848 = ct{1421};
t4849 = ct{1422};
t4850 = ct{1423};
t4853 = ct{1424};
t4869 = ct{1425};
t4871 = ct{1426};
t4872 = ct{1427};
t4874 = ct{1428};
t4877 = ct{1429};
t4878 = ct{1430};
t4879 = ct{1431};
t4884 = ct{1432};
t4885 = ct{1433};
t4886 = ct{1434};
t4890 = ct{1435};
t4891 = ct{1436};
t4892 = ct{1437};
t4893 = ct{1438};
t4894 = ct{1439};
t4895 = ct{1440};
t4902 = ct{1441};
t4915 = ct{1442};
t4920 = ct{1443};
t4923 = ct{1444};
t4924 = ct{1445};
t4925 = ct{1446};
t4926 = ct{1447};
t50 = ct{1448};
t5014 = ct{1449};
t5015 = ct{1450};
t5016 = ct{1451};
t5017 = ct{1452};
t5025 = ct{1453};
t5027 = ct{1454};
t5028 = ct{1455};
t5036 = ct{1456};
t5037 = ct{1457};
t5045 = ct{1458};
t5046 = ct{1459};
t5052 = ct{1460};
t5053 = ct{1461};
t5059 = ct{1462};
t5062 = ct{1463};
t5063 = ct{1464};
t5066 = ct{1465};
t5070 = ct{1466};
t5072 = ct{1467};
t5075 = ct{1468};
t5079 = ct{1469};
t5084 = ct{1470};
t5085 = ct{1471};
t5086 = ct{1472};
t5087 = ct{1473};
t5088 = ct{1474};
t5089 = ct{1475};
t5090 = ct{1476};
t5091 = ct{1477};
t5092 = ct{1478};
t5093 = ct{1479};
t5094 = ct{1480};
t5095 = ct{1481};
t5096 = ct{1482};
t5097 = ct{1483};
t5098 = ct{1484};
t5099 = ct{1485};
t5108 = ct{1486};
t5111 = ct{1487};
t5194 = ct{1488};
t5195 = ct{1489};
t5203 = ct{1490};
t5209 = ct{1491};
t5217 = ct{1492};
t5218 = ct{1493};
t5219 = ct{1494};
t5240 = ct{1495};
t5250 = ct{1496};
t5252 = ct{1497};
t5255 = ct{1498};
t5262 = ct{1499};
t5274 = ct{1500};
t5276 = ct{1501};
t5278 = ct{1502};
t5279 = ct{1503};
t5280 = ct{1504};
t5281 = ct{1505};
t5283 = ct{1506};
t5285 = ct{1507};
t5286 = ct{1508};
t5287 = ct{1509};
t5289 = ct{1510};
t5291 = ct{1511};
t5292 = ct{1512};
t5295 = ct{1513};
t5296 = ct{1514};
t5297 = ct{1515};
t5300 = ct{1516};
t5301 = ct{1517};
t5302 = ct{1518};
t5303 = ct{1519};
t5304 = ct{1520};
t5308 = ct{1521};
t5309 = ct{1522};
t5310 = ct{1523};
t5312 = ct{1524};
t5320 = ct{1525};
t5321 = ct{1526};
t5356 = ct{1527};
t5357 = ct{1528};
t5361 = ct{1529};
t5363 = ct{1530};
t5370 = ct{1531};
t5372 = ct{1532};
t5381 = ct{1533};
t5391 = ct{1534};
t5392 = ct{1535};
t5393 = ct{1536};
t5395 = ct{1537};
t5399 = ct{1538};
t5400 = ct{1539};
t5401 = ct{1540};
t5402 = ct{1541};
t5403 = ct{1542};
t5404 = ct{1543};
t5415 = ct{1544};
t5416 = ct{1545};
t5433 = ct{1546};
t5434 = ct{1547};
t5436 = ct{1548};
t5437 = ct{1549};
t5438 = ct{1550};
t5439 = ct{1551};
t5452 = ct{1552};
t5456 = ct{1553};
t5457 = ct{1554};
t5458 = ct{1555};
t5459 = ct{1556};
t5460 = ct{1557};
t5464 = ct{1558};
t5481 = ct{1559};
t5487 = ct{1560};
t5488 = ct{1561};
t5494 = ct{1562};
t5495 = ct{1563};
t5499 = ct{1564};
t5535 = ct{1565};
t5536 = ct{1566};
t5537 = ct{1567};
t5538 = ct{1568};
t5539 = ct{1569};
t5540 = ct{1570};
t5541 = ct{1571};
t5542 = ct{1572};
t5543 = ct{1573};
t5544 = ct{1574};
t5545 = ct{1575};
t5548 = ct{1576};
t5550 = ct{1577};
t5561 = ct{1578};
t5569 = ct{1579};
t5570 = ct{1580};
t5586 = ct{1581};
t56 = ct{1582};
t5604 = ct{1583};
t5607 = ct{1584};
t5678 = ct{1585};
t5684 = ct{1586};
t5730 = ct{1587};
t5731 = ct{1588};
t5734 = ct{1589};
t5735 = ct{1590};
t5738 = ct{1591};
t5739 = ct{1592};
t5741 = ct{1593};
t5742 = ct{1594};
t5758 = ct{1595};
t5759 = ct{1596};
t5760 = ct{1597};
t5761 = ct{1598};
t5779 = ct{1599};
t5782 = ct{1600};
t5783 = ct{1601};
t58 = ct{1602};
t5849 = ct{1603};
t5896 = ct{1604};
t59 = ct{1605};
t5901 = ct{1606};
t5902 = ct{1607};
t5916 = ct{1608};
t5917 = ct{1609};
t5952 = ct{1610};
t5955 = ct{1611};
t5990 = ct{1612};
t60 = ct{1613};
t6011 = ct{1614};
t6013 = ct{1615};
t6014 = ct{1616};
t6255 = ct{1617};
t6256 = ct{1618};
t6257 = ct{1619};
t628 = ct{1620};
t635 = ct{1621};
t636 = ct{1622};
t638 = ct{1623};
t640 = ct{1624};
t641 = ct{1625};
t642 = ct{1626};
t643 = ct{1627};
t645 = ct{1628};
t646 = ct{1629};
t649 = ct{1630};
t654 = ct{1631};
t655 = ct{1632};
t656 = ct{1633};
t6564 = ct{1634};
t6565 = ct{1635};
t657 = ct{1636};
t659 = ct{1637};
t660 = ct{1638};
t6622 = ct{1639};
t6623 = ct{1640};
t663 = ct{1641};
t664 = ct{1642};
t665 = ct{1643};
t666 = ct{1644};
t667 = ct{1645};
t668 = ct{1646};
t669 = ct{1647};
t67 = ct{1648};
t670 = ct{1649};
t672 = ct{1650};
t673 = ct{1651};
t674 = ct{1652};
t6745 = ct{1653};
t675 = ct{1654};
t6751 = ct{1655};
t676 = ct{1656};
t677 = ct{1657};
t678 = ct{1658};
t679 = ct{1659};
t68 = ct{1660};
t681 = ct{1661};
t682 = ct{1662};
t683 = ct{1663};
t684 = ct{1664};
t685 = ct{1665};
t686 = ct{1666};
t687 = ct{1667};
t689 = ct{1668};
t691 = ct{1669};
t6919 = ct{1670};
t692 = ct{1671};
t6920 = ct{1672};
t693 = ct{1673};
t694 = ct{1674};
t6987 = ct{1675};
t70 = ct{1676};
t702 = ct{1677};
t707 = ct{1678};
t708 = ct{1679};
t71 = ct{1680};
t710 = ct{1681};
t715 = ct{1682};
t7150 = ct{1683};
t716 = ct{1684};
t717 = ct{1685};
t718 = ct{1686};
t721 = ct{1687};
t722 = ct{1688};
t724 = ct{1689};
t725 = ct{1690};
t73 = ct{1691};
t736 = ct{1692};
t738 = ct{1693};
t740 = ct{1694};
t741 = ct{1695};
t749 = ct{1696};
t756 = ct{1697};
t76 = ct{1698};
t762 = ct{1699};
t768 = ct{1700};
t777 = ct{1701};
t792 = ct{1702};
t793 = ct{1703};
t8 = ct{1704};
t801 = ct{1705};
t802 = ct{1706};
t808 = ct{1707};
t813 = ct{1708};
t819 = ct{1709};
t821 = ct{1710};
t850 = ct{1711};
t855 = ct{1712};
t874 = ct{1713};
t878 = ct{1714};
t89 = ct{1715};
t9 = ct{1716};
t90 = ct{1717};
t91 = ct{1718};
t92 = ct{1719};
t941 = ct{1720};
t944 = ct{1721};
t948 = ct{1722};
t951 = ct{1723};
t97 = ct{1724};
t6050 = et54.*et55;
t6061 = t2297.*(-t4504+t4515+t3395.*(t2813-t2835+t12.*(t1456-t2355).*1.02e-6+t17.*(t1456-t2355).*9.0e-8)+t3396.*(-t2804+t2838+t3109+t17.*(t1456-t2355).*9.3e-7)).*(-1.0./2.0);
t6062 = (t2297.*(-t4504+t4515+t3395.*(t2813-t2835+t12.*(t1456-t2355).*1.02e-6+t17.*(t1456-t2355).*9.0e-8)+t3396.*(-t2804+t2838+t3109+t17.*(t1456-t2355).*9.3e-7)))./2.0;
t6073 = t3047.*(-t4504+t4515+t3395.*(t2813-t2835+t12.*(t1456-t2355).*1.02e-6+t17.*(t1456-t2355).*9.0e-8)+t3396.*(-t2804+t2838+t3109+t17.*(t1456-t2355).*9.3e-7)).*(-1.0./2.0);
t6074 = (t3047.*(-t4504+t4515+t3395.*(t2813-t2835+t12.*(t1456-t2355).*1.02e-6+t17.*(t1456-t2355).*9.0e-8)+t3396.*(-t2804+t2838+t3109+t17.*(t1456-t2355).*9.3e-7)))./2.0;
t6092 = t4212+t4214+t5015+t5017;
t6097 = t201.*(t4213+t5016+t123.*t188.*(t2694-t2701+t3036-t3043).*2.442490654175345e-23+t50.*t189.*t4915.*(t42-t43).*2.711709361697228e-39).*(-1.0./2.0);
t6400 = t3934.*t4215.*(t1554+t2361+t2362+t2367+t2414+t3961+t3968+t4198+t4201+t11.*(-t1901+t3122+t3277).*5.68686e-3).*(-5.43845e-3);
et56 = -t2137+t2777+t2778+t2779-t2787+t4050-t4246+t4248+t21.*(t1959-t3313+t38.*t1022.*(t855-t878).*2.196325630278387e-1).*6.1855407534e-5;
et57 = t27.*(t1959-t3313+t38.*t1022.*(t855-t878).*2.196325630278387e-1).*1.35652563578e-4;
t6442 = (t4172.*(et56+et57).*(t2674-t2676+t3022-t3027))./2.0;
et58 = -t2137+t2777+t2778+t2779-t2787+t4050-t4246+t4248+t21.*(t1959-t3313+t38.*t1022.*(t855-t878).*2.196325630278387e-1).*6.1855407534e-5;
et59 = t27.*(t1959-t3313+t38.*t1022.*(t855-t878).*2.196325630278387e-1).*1.35652563578e-4;
t7004 = t6011.*(et58+et59).*(-1.0./2.0);
et60 = -t2137+t2777+t2778+t2779-t2787+t4050-t4246+t4248+t21.*(t1959-t3313+t38.*t1022.*(t855-t878).*2.196325630278387e-1).*6.1855407534e-5;
et61 = t27.*(t1959-t3313+t38.*t1022.*(t855-t878).*2.196325630278387e-1).*1.35652563578e-4;
t7005 = (t6011.*(et60+et61))./2.0;
t7296 = t4745+t4748+t4749+t4750+t5084+t5089+t5092+t5096;
t7299 = t4752+t4754+t4758+t4759+t5088+t5090+t5098+t5099;
et62 = t50.*t202.*(t4744-t5084+t5087-t5089-t5096+t3913.*(t2694-t2701+t3036-t3043).*5.0e-8+t3934.*(-t1881+t3121+t3276).*5.0e-8+t3934.*(-t1901+t3122+t3277).*1.1e-7);
et63 = -4.771516396025243e-17;
t7304 = et62.*et63;
et64 = t50.*t202.*(t4744-t5084+t5087-t5089-t5096+t3913.*(t2694-t2701+t3036-t3043).*5.0e-8+t3934.*(-t1881+t3121+t3276).*5.0e-8+t3934.*(-t1901+t3122+t3277).*1.1e-7);
et65 = 4.771516396025243e-17;
t7305 = et64.*et65;
et66 = t50.*t202.*(t4757-t5088-t5090+t5097-t5098+t3913.*(t2694-t2701+t3036-t3043).*1.6e-7+t3934.*(-t1881+t3121+t3276).*1.6e-7+t3934.*(-t1901+t3122+t3277).*5.0e-8);
et67 = -2.836813422250052e-17;
t7306 = et66.*et67;
t3293 = -t3282;
t3299 = -t3289;
t3302 = -t3292;
t3305 = -t3301;
t3314 = -t3308;
t3316 = -t3311;
t3317 = -t3312;
t3347 = -t3339;
t3350 = -t3342;
t3355 = -t3349;
t3367 = -t3360;
t3368 = -t3362;
t3414 = -t3404;
t3415 = -t3407;
t3424 = -t3421;
t3425 = -t3423;
t3482 = -t3480;
t3510 = t12.*t3502;
t3511 = -t3504;
t3512 = t17.*t3502;
t3515 = t11.*t3503;
t3516 = t12.*t3503;
t3518 = t16.*t3503;
t3519 = t17.*t3503;
t3525 = t3504.*(3.0./5.0e+2);
t3527 = t3506.*(3.0./5.0e+2);
t3532 = t16.*t3502.*(3.0./5.0e+2);
t3549 = t50.*t202.*t3249.*8.875020496606951e-23;
t3551 = -t3548;
t3558 = -t3553;
t3561 = t50.*t202.*t3249.*8.588729512845436e-24;
t3562 = t22.*t3547;
t3563 = t28.*t3547;
t3564 = t21.*t3550;
t3565 = t22.*t3550;
t3567 = t27.*t3550;
t3568 = t28.*t3550;
t3572 = t3554.*(3.0./5.0e+2);
t3574 = t3556.*(3.0./5.0e+2);
t3583 = t27.*t3547.*(3.0./5.0e+2);
t3591 = t3505.*9.99471e-3;
t3592 = t3507.*1.838876e-2;
t3593 = t3504.*1.247162e-2;
t3594 = t3506.*1.247162e-2;
t3595 = t3504.*5.68686e-3;
t3596 = t3506.*5.68686e-3;
t3612 = t11.*t3502.*1.247162e-2;
t3613 = t3504.*3.131399999999998e-4;
t3614 = t3506.*3.131399999999998e-4;
t3615 = t16.*t3502.*5.68686e-3;
t3634 = t16.*t3502.*3.131399999999998e-4;
t3639 = t3555.*9.99471e-3;
t3640 = t3557.*1.838876e-2;
t3641 = t3554.*1.247162e-2;
t3642 = t3556.*1.247162e-2;
t3657 = t21.*t3547.*1.247162e-2;
t3658 = t3554.*3.131399999999998e-4;
t3659 = t3556.*3.131399999999998e-4;
t3669 = t3582.*(-1.838876e-2);
t3670 = t3554.*4.36041e-5;
t3671 = t3556.*4.36041e-5;
t3673 = t27.*t3547.*3.131399999999998e-4;
t3679 = t27.*t3547.*4.36041e-5;
t3685 = t3680./2.0;
t3689 = -t3686;
t3714 = t3554.*1.35652563578e-4;
t3715 = t3556.*1.35652563578e-4;
t3716 = t3557.*1.33637554986e-4;
t3717 = t3555.*7.26350557185e-5;
t3718 = t3554.*6.1855407534e-5;
t3719 = t3556.*6.1855407534e-5;
t3729 = t2363.*t3249.*9.3e-7;
t3731 = t21.*t3547.*1.35652563578e-4;
t3737 = t27.*t3547.*6.1855407534e-5;
t3747 = t2363.*t3249.*9.0e-8;
t3750 = t3582.*(-1.33637554986e-4);
t3769 = t3768./2.0;
t3821 = -t3818;
t3823 = -t3822;
t3826 = -t3825;
t3830 = t3055.*t3249.*9.3e-7;
t3832 = -t3829;
t3835 = t3055.*t3249.*9.0e-8;
t3853 = -t3841;
t3854 = -t3842;
t3858 = t2973.*t3547;
t3859 = t2971.*t3550;
t3860 = t2972.*t3550;
t3864 = t2973.*t3550;
t3870 = t2976.*t3547;
t3886 = -t3547.*(t1545-t2615);
t3889 = t3547.*(t1545-t2615);
t3890 = t3887./2.0;
t3900 = t3119.*t3547;
t3906 = t3905.*(-1.0./2.0);
t3908 = t21.*t3133.*t3547;
t3930 = t3155.*t3547;
t3932 = t3155.*t3550;
t3960 = t3952./2.0;
t3976 = t3222+t3506;
t3993 = t3213.*t3547;
t4011 = -t4009;
t4013 = (t3237.*t3502)./1.0e+8;
t4015 = (t3237.*t3503)./1.0e+8;
t4017 = t11.*t3237.*t3502.*(-1.0e-8);
t4019 = t3240+t3556;
t4020 = t3248+t3554;
t4030 = t4021./2.0;
t4062 = -t4058;
t4065 = t3237.*t3502.*9.840000000000001e-6;
t4070 = t3237.*t3503.*9.840000000000001e-6;
t4077 = -t4067;
t4079 = -t4068;
t4085 = t3237.*t3502.*6.2e-7;
t4088 = t3237.*t3502.*3.24e-6;
t4089 = t3237.*t3502.*7.83e-6;
t4091 = t3237.*t3503.*6.2e-7;
t4093 = t3237.*t3503.*3.24e-6;
t4095 = t3237.*t3503.*7.83e-6;
t4099 = t16.*t3237.*t3502.*5.7e-7;
t4100 = t11.*t3237.*t3502.*1.02e-6;
t4103 = t11.*t3237.*t3502.*2.4e-7;
t4105 = t11.*t3237.*t3502.*4.0e-8;
t4106 = t16.*t3237.*t3502.*4.0e-8;
t4116 = t28.*(t3242-t3554).*(-9.99471e-3);
t4117 = t22.*(t3242-t3554).*(-1.838876e-2);
t4139 = -t4125;
t4173 = t22.*(t3242-t3554).*(-1.33637554986e-4);
t4174 = t28.*(t3242-t3554).*(-7.26350557185e-5);
t4178 = -t4171;
t4188 = -t4182;
t4189 = t4125.*9.99471e-3;
t4190 = t4126.*1.838876e-2;
t4199 = -t4192;
t4205 = t4192./2.0;
t4207 = t3431.*t3547;
t4218 = -t4216;
t4219 = t4169.*9.99471e-3;
t4221 = t4171.*1.838876e-2;
t4229 = -t4225;
t4230 = -t4227;
t4239 = t3483.*t3547;
t4240 = t3483.*t3550;
t4242 = t4238./2.0;
t4249 = t4169.*7.26350557185e-5;
t4251 = -t4245;
t4254 = t4171.*1.33637554986e-4;
t4262 = t3505+t3514;
t4264 = t3507+t3524;
t4269 = t4266./2.0;
t4271 = -t4268;
t4272 = t4268./2.0;
t4280 = (t3502.*t3547)./1.0e+8;
t4281 = (t3503.*t3547)./1.0e+8;
t4282 = (t3502.*t3550)./1.0e+8;
t4285 = t4284./2.0;
t4289 = t3555+t3571;
t4290 = t3557+t3582;
t4296 = t3502.*t3547.*6.2e-7;
t4299 = t3503.*t3547.*6.2e-7;
t4300 = t3502.*t3550.*6.2e-7;
t4304 = t16.*t3502.*t3547.*5.7e-7;
t4305 = t11.*t3502.*t3547.*1.02e-6;
t4308 = t11.*t3502.*t3547.*2.4e-7;
t4309 = t11.*t3502.*t3547.*4.0e-8;
t4310 = t16.*t3502.*t3547.*4.0e-8;
t4319 = t11.*t2297.*(t3242-t3554).*(-1.02e-6);
t4323 = t2300+t2313+t3292+t3311;
t4332 = t27.*t3547.*t3815;
t4337 = t4335./2.0;
t4340 = -t4336;
t4341 = t4336./2.0;
t4344 = -t3063.*(t3242-t3554);
t4354 = -t3133.*(t3242-t3554);
t4357 = (t1953-t2828).*(t3242-t3554);
t4367 = t2962+t3538+t3542;
t4376 = t2753+t2792+t3408+t3422;
t4453 = t3395.*t3977;
t4456 = t3396.*t3979;
t4464 = t21.*t3547.*t3893;
t4465 = -t4463;
t4477 = -t4473;
t4478 = -t4474;
t4479 = -t4475;
t4486 = t4485.*(-1.0./2.0);
t4495 = (t3502.*t3934)./1.0e+8;
t4497 = (t3502.*t3937)./1.0e+8;
t4499 = (t3503.*t3934)./1.0e+8;
t4509 = t3502.*t3934.*9.840000000000001e-6;
t4516 = t3503.*t3934.*9.840000000000001e-6;
t4518 = t3503.*t3937.*9.840000000000001e-6;
t4523 = t3502.*t3934.*6.2e-7;
t4524 = t3502.*t3934.*3.24e-6;
t4525 = t3502.*t3934.*7.83e-6;
t4528 = t3502.*t3937.*3.24e-6;
t4529 = t3503.*t3934.*6.2e-7;
t4531 = t3502.*t3937.*7.83e-6;
t4534 = t3502.*t3937.*6.2e-7;
t4536 = t3503.*t3934.*3.24e-6;
t4538 = t3503.*t3934.*7.83e-6;
t4542 = t16.*t3502.*t3934.*5.7e-7;
t4543 = t11.*t3502.*t3934.*1.02e-6;
t4545 = -t4539;
t4549 = t11.*t3502.*t3934.*2.4e-7;
t4550 = t11.*t3502.*t3934.*4.0e-8;
t4552 = t16.*t3502.*t3934.*4.0e-8;
t4643 = -t4636;
t4645 = (t3242-t3554).*(t335-t1539-t2831+t2851);
t4646 = t11.*(t1861-t3221).*(t3242-t3554).*1.02e-6;
t4651 = t3502.*t4146;
t4655 = t3547.*(t951+t10.*(-t1881+t3121+t3276)).*(-1.0e-8);
t4656 = (t3547.*(t951+t10.*(-t1881+t3121+t3276)))./1.0e+8;
t4659 = (t3502.*t4151)./1.0e+8;
t4668 = t3547.*(t951+t10.*(-t1881+t3121+t3276)).*(-6.2e-7);
t4669 = t3547.*(t951+t10.*(-t1881+t3121+t3276)).*6.2e-7;
t4671 = t3502.*t4151.*6.2e-7;
t4675 = t3547.*t4187.*7.26735e-3;
t4684 = -t3815.*(t3242-t3554);
t4687 = -t3819.*(t3242-t3554);
t4717 = -t3872.*(t3242-t3554);
t4719 = t3872.*(t3242-t3554);
t4726 = t3216.*t4419;
t4727 = t3217.*t4419;
t4732 = -t3893.*(t3242-t3554);
t4734 = t3893.*(t3242-t3554);
t4737 = t3502.*t4350;
t4742 = t3236.*t4454.*7.26735e-3;
t4743 = t3237.*t4454.*7.26735e-3;
t4826 = t3547.*t4371.*7.26735e-3;
t4839 = t12.*t4835;
t4840 = t17.*t4835;
t4844 = t3502.*t4418;
t4880 = t3946+t4176;
t4916 = t4894.*9.99471e-3;
t4917 = t4893.*1.838876e-2;
t4927 = t3547.*t4452.*7.26735e-3;
t4929 = t22.*(t3242-t3554).*(t2813-t2835+t12.*(t1456-t2355).*1.02e-6+t17.*(t1456-t2355).*9.0e-8);
t4930 = t28.*(t3242-t3554).*(-t2804+t2838+t3109+t17.*(t1456-t2355).*9.3e-7);
t4942 = t4894.*7.26350557185e-5;
t4944 = t4893.*1.33637554986e-4;
t5012 = t3216.*t4710;
t5013 = t3217.*t4710;
t5033 = t3236.*t4715.*7.26735e-3;
t5034 = t3237.*t4715.*7.26735e-3;
t5038 = (t50.*t202.*t5028)./1.801439850948198e+16;
t5047 = -t4714.*(t1861-t3221);
t5048 = t3502.*t4714;
t5050 = t3133.*t4872;
t5060 = (t3236.*t4838)./1.0e+8;
t5064 = t3236.*t4835.*5.7e-7;
t5067 = t3236.*t4838.*1.02e-6;
t5069 = t3236.*t4835.*4.0e-8;
t5073 = t3236.*t4838.*2.4e-7;
t5077 = t3236.*t4838.*4.0e-8;
t5080 = t4723.*(t1896-t3239).*(-7.26735e-3);
t5081 = t4723.*(t1896-t3239).*7.26735e-3;
t5082 = t3547.*t4723.*7.26735e-3;
t5113 = t3502.*t4814;
t5114 = -t5108;
t5119 = t3503.*t4814;
t5140 = t3847+t3861+t3933;
t5142 = t645+t646+t666+t683+t1576+t1579+t1584+t1585+t2291+t2311+t2682+t3029+t3288+t3307;
t5144 = t3547.*(t11.*((t237.*(t42-t43))./9.007199254740992e+15+t15.*(-t1881+t3121+t3276))+t16.*(-t1901+t3122+t3277)).*(-1.0e-8);
t5145 = t4838.*(t1896-t3239).*(-1.0e-8);
t5146 = (t4838.*(t1896-t3239))./1.0e+8;
t5160 = t4835.*(t1896-t3239).*(-5.7e-7);
t5165 = t4835.*(t1896-t3239).*5.7e-7;
t5168 = t3547.*(t11.*((t237.*(t42-t43))./9.007199254740992e+15+t15.*(-t1881+t3121+t3276))+t16.*(-t1901+t3122+t3277)).*(-1.02e-6);
t5170 = t4838.*(t1896-t3239).*(-1.02e-6);
t5171 = t3547.*(t11.*((t237.*(t42-t43))./9.007199254740992e+15+t15.*(-t1881+t3121+t3276))+t16.*(-t1901+t3122+t3277)).*(-2.4e-7);
t5172 = t4835.*(t1896-t3239).*(-4.0e-8);
t5173 = t3547.*t4837.*5.7e-7;
t5174 = t4838.*(t1896-t3239).*1.02e-6;
t5175 = t4838.*(t1896-t3239).*(-2.4e-7);
t5176 = t4835.*(t1896-t3239).*4.0e-8;
t5177 = t3547.*(t11.*((t237.*(t42-t43))./9.007199254740992e+15+t15.*(-t1881+t3121+t3276))+t16.*(-t1901+t3122+t3277)).*(-4.0e-8);
t5178 = t4838.*(t1896-t3239).*2.4e-7;
t5179 = t4838.*(t1896-t3239).*(-4.0e-8);
t5180 = t4838.*(t1896-t3239).*4.0e-8;
t5181 = t3547.*t4837.*4.0e-8;
t5196 = -t5194;
t5197 = t3547.*t4853.*7.26735e-3;
t5198 = t3550.*t4853.*7.26735e-3;
t5202 = (t3502.*t4915)./1.0e+8;
t5210 = t3503.*t4915.*9.840000000000001e-6;
t5213 = t3502.*t4915.*3.24e-6;
t5214 = t3502.*t4915.*7.83e-6;
t5215 = t3502.*t4915.*6.2e-7;
t5246 = t3649.*t4322.*(t2694-t2701+t3036-t3043).*(-1.444822e-2);
t5247 = t3649.*t4322.*(t2694-t2701+t3036-t3043).*1.444822e-2;
t5251 = -t5250;
t5254 = -t5252;
t5256 = t3638.*t4374.*(t2674-t2676+t3022-t3027).*(-1.0./2.0);
t5257 = (t3638.*t4374.*(t2674-t2676+t3022-t3027))./2.0;
t5260 = t3811+t4029+t4316;
t5261 = t3893.*t4872;
t5277 = t4838.*(t2694-t2701+t3036-t3043).*(-1.0e-8);
t5284 = t4835.*(t2694-t2701+t3036-t3043).*(-5.7e-7);
t5288 = t4838.*(t2694-t2701+t3036-t3043).*(-1.02e-6);
t5290 = t4835.*(t2694-t2701+t3036-t3043).*(-4.0e-8);
t5293 = t4838.*(t2694-t2701+t3036-t3043).*1.02e-6;
t5294 = t4838.*(t2694-t2701+t3036-t3043).*(-2.4e-7);
t5298 = t4838.*(t2694-t2701+t3036-t3043).*(-4.0e-8);
t5305 = t1193+t1194+t1222+t1236+t2138+t2141+t2156+t2157+t2733+t2765+t2948+t3069+t3406+t3418;
t5315 = t4838.*(t3242-t3554).*(-1.02e-6);
t5347 = t4167+t4893;
t5350 = t4177+t4894;
t5444 = t3237.*t5320.*9.3e-7;
t5445 = t3237.*t5320.*9.0e-8;
t5446 = t3237.*t5321.*1.02e-6;
t5448 = t3237.*t5321.*9.0e-8;
t5485 = t2520+t2525+t3478+t3481+t4231+t4235;
t5513 = t3547.*t5320.*9.3e-7;
t5516 = t3547.*t5320.*9.0e-8;
t5517 = t3547.*t5321.*1.02e-6;
t5520 = t3547.*t5321.*9.0e-8;
t5549 = t188.*t5543.*4.297799892626299e-1;
t5555 = t4215.*t4711.*(t2694-t2701+t3036-t3043).*(-5.43845e-3);
t5556 = t4215.*t4711.*(t2694-t2701+t3036-t3043).*5.43845e-3;
t5560 = t1548+t1564+t2326+t2343+t2352+t2353+t2354+t3150+t3379+t3958+t3970;
t5565 = (t2307.*t5543)./2.0;
t5566 = (t11.*t2297.*t5543)./2.0;
t5568 = (t2338.*t5543)./2.0;
t5575 = t4172.*t4774.*(t2674-t2676+t3022-t3027).*(-1.0./2.0);
t5576 = (t4172.*t4774.*(t2674-t2676+t3022-t3027))./2.0;
t5590 = (t2994.*t5543)./2.0;
t5605 = t3934.*t5320.*9.3e-7;
t5608 = t3934.*t5320.*9.0e-8;
t5609 = t3934.*t5321.*1.02e-6;
t5611 = t3934.*t5321.*9.0e-8;
t5612 = t5543.*(t1456-t2355).*(-1.0./2.0);
t5660 = -(t4893-t28.*(t1005+t20.*(t1941-t3315+t39.*t1022.*(t855-t878).*2.196325630278387e-1))).*(t2813-t2835+t12.*(t1456-t2355).*1.02e-6+t17.*(t1456-t2355).*9.0e-8);
t5692 = t2130+t2160+t2748+t2749+t2788+t2795+t2805+t3212+t3472+t4037+t4047;
t5803 = t3397+t4021+t4027+t4028+t4317;
t5903 = t3768+t3816+t3905+t3952+t4238+t4284;
t5938 = t201.*t5916.*4.297799892626299e-1;
t5941 = t201.*t5917.*2.555174374272992e-1;
t5954 = -t5952;
t6002 = t1553+t2359+t2365+t2366+t2389+t3954+t3962+t3966+t4200+t4202;
t6033 = t4504+t4506+t4512+t4527;
t6049 = t2137+t2787+t2798+t2799+t2802+t4040+t4043+t4057+t4246+t4253;
t6142 = t3216.*(t3831+t3842-t4328+t4421+t3166.*(t1959-t3313+t38.*t1022.*(t855-t878).*2.196325630278387e-1)+t3119.*(t1896-t3239)).*(-1.0./2.0);
t6143 = (t3216.*(t3831+t3842-t4328+t4421+t3166.*(t1959-t3313+t38.*t1022.*(t855-t878).*2.196325630278387e-1)+t3119.*(t1896-t3239)))./2.0;
t6271 = ((t2674-t2676+t3022-t3027).*(t3831+t3842-t4328+t4421+t3166.*(t1959-t3313+t38.*t1022.*(t855-t878).*2.196325630278387e-1)+t3119.*(t1896-t3239)))./2.0;
t6394 = (t4774.*t6011)./2.0;
t6574 = (t4711.*t6255)./2.0;
t6588 = t2309+t2374+t2509+t2532+t2977+t2982+t3927+t4145+t4196+t4203+t4869+t4871;
t7117 = t1549+t1565+t2309+t2322+t2327+t2328+t2357+t2375+t2509+t2532+t2977+t2982+t3151+t3380+t3927+t3965+t3969+t4145+t4196+t4203+t4869+t4871;
t7141 = t1554+t2309+t2361+t2362+t2367+t2374+t2414+t2509+t2532+t2977+t2982+t3961+t3968+t3972+t4196+t4198+t4203+t4211+t4869+t4871;
t3520 = t16.*t3510;
t3521 = t16.*t3512;
t3522 = -t3512;
t3526 = -t3518;
t3529 = -t3525;
t3531 = -t3527;
t3534 = t3515.*(3.0./5.0e+2);
t3535 = t3518.*(3.0./5.0e+2);
t3569 = -t3563;
t3573 = -t3567;
t3575 = t27.*t3562;
t3576 = t27.*t3563;
t3581 = -t3574;
t3586 = t3564.*(3.0./5.0e+2);
t3587 = t3567.*(3.0./5.0e+2);
t3601 = -t3592;
t3603 = -t3593;
t3606 = t3510.*9.99471e-3;
t3607 = t3512.*9.99471e-3;
t3608 = t3510.*1.838876e-2;
t3610 = t3512.*1.838876e-2;
t3618 = t3516.*9.99471e-3;
t3622 = t3519.*1.838876e-2;
t3623 = -t3612;
t3624 = t3515.*1.247162e-2;
t3625 = t3518.*1.247162e-2;
t3626 = -t3613;
t3627 = t3515.*5.68686e-3;
t3629 = t3518.*5.68686e-3;
t3636 = t3515.*3.131399999999998e-4;
t3637 = t3518.*3.131399999999998e-4;
t3647 = -t3640;
t3650 = -t3642;
t3652 = t3562.*9.99471e-3;
t3653 = t3563.*9.99471e-3;
t3654 = t3562.*1.838876e-2;
t3656 = t3563.*1.838876e-2;
t3661 = t3565.*9.99471e-3;
t3663 = t3568.*1.838876e-2;
t3664 = t3564.*1.247162e-2;
t3665 = t3567.*1.247162e-2;
t3677 = t3564.*3.131399999999998e-4;
t3678 = t3567.*3.131399999999998e-4;
t3681 = t3564.*4.36041e-5;
t3682 = t3567.*4.36041e-5;
t3688 = -t3685;
t3721 = -t3714;
t3724 = -t3716;
t3732 = t3562.*1.33637554986e-4;
t3733 = t3563.*1.33637554986e-4;
t3735 = t3562.*7.26350557185e-5;
t3736 = t3563.*7.26350557185e-5;
t3738 = -t3729;
t3739 = t3564.*1.35652563578e-4;
t3740 = t3567.*1.35652563578e-4;
t3742 = t3568.*1.33637554986e-4;
t3743 = t3565.*7.26350557185e-5;
t3744 = t3564.*6.1855407534e-5;
t3745 = -t3737;
t3746 = t3567.*6.1855407534e-5;
t3752 = -t3747;
t3770 = -t3769;
t3866 = -t3858;
t3867 = -t3860;
t3868 = -t3864;
t3891 = -t3890;
t3939 = -t3932;
t3967 = -t3960;
t3980 = t3224+t3511;
t3984 = t12.*t3976;
t3985 = t17.*t3976;
t3991 = t3229+t3515;
t4002 = -t3993;
t4014 = -t4013;
t4016 = t11.*t4013;
t4024 = t22.*t4019;
t4025 = t28.*t4019;
t4026 = t3247+t3564;
t4069 = -t4065;
t4090 = -t4085;
t4097 = -t4091;
t4102 = -t4100;
t4107 = -t4105;
t4108 = -t4106;
t4193 = -t4189;
t4208 = -t4205;
t4224 = -t4221;
t4241 = -t4239;
t4243 = -t4240;
t4244 = -t4242;
t4258 = -t4254;
t4270 = -t4269;
t4283 = t11.*t4280;
t4286 = -t4285;
t4311 = -t4309;
t4312 = -t4310;
t4339 = -t4337;
t4342 = -t4341;
t4353 = t3133.*t4019;
t4362 = -t4357;
t4403 = -t4019.*(t2801-t2850);
t4404 = (t3236.*t3976)./1.0e+8;
t4422 = t3236.*t3976.*5.7e-7;
t4423 = t3236.*t3976.*1.02e-6;
t4425 = t3236.*t3976.*2.4e-7;
t4426 = t3236.*t3976.*4.0e-8;
t4455 = -t4453;
t4458 = t4453./2.0;
t4460 = t4456./2.0;
t4466 = -t4464;
t4500 = t11.*t4495;
t4548 = -t4542;
t4554 = -t4552;
t4560 = t3976.*(t1896-t3239).*(-1.0e-8);
t4561 = (t3976.*(t1896-t3239))./1.0e+8;
t4570 = t3236.*t4262.*9.3e-7;
t4571 = t3236.*t4262.*9.0e-8;
t4572 = t3236.*t4264.*1.02e-6;
t4575 = t3543.*t3976.*5.7e-7;
t4576 = t3236.*t4264.*9.0e-8;
t4578 = t3976.*(t1896-t3239).*(-5.7e-7);
tau_c = ft_10({dq1,dq2,dq3,dq4,dq5,dq6,t10,t1005,t1022,t1089,t11,t1104,t1105,t1108,t1115,t1121,t1158,t1159,t1190,t1196,t12,t1205,t1207,t1208,t1210,t1212,t1214,t1217,t1218,t1219,t1220,t1221,t123,t1230,t1235,t1237,t1238,t1288,t1289,t13,t1302,t1303,t1319,t1320,t1336,t1348,t1350,t1351,t1360,t1369,t1378,t1396,t14,t140,t1425,t1435,t1456,t1477,t1488,t15,t1513,t1539,t1544,t1547,t1548,t1553,t1554,t1559,t1564,t1576,t1577,t1578,t1579,t1581,t1584,t1585,t1586,t1587,t1591,t1595,t1596,t1598,t1599,t16,t1600,t1601,t1602,t1604,t1605,t1606,t1607,t1608,t1609,t1612,t1613,t1614,t1615,t1616,t1626,t1627,t1628,t1629,t1631,t1637,t1640,t1641,t1648,t1649,t1659,t1660,t1661,t1666,t1667,t1683,t1686,t1690,t1692,t17,t1700,t1701,t1703,t1704,t1705,t1712,t1717,t1738,t1741,t1742,t1750,t1752,t1753,t1754,t1758,t1759,t1775,t1776,t18,t1861,t1874,t1879,t188,t1881,t189,t1896,t19,t1901,t1941,t1953,t1959,t1973,t1993,t1994,t20,t201,t202,t2023,t2053,t2060,t2089,t2090,t2098,t2099,t21,t2117,t2120,t2122,t2123,t2125,t2137,t2139,t2140,t2142,t2145,t2146,t2147,t2149,t2150,t2151,t2152,t2153,t2154,t2155,t2159,t2162,t2164,t2165,t2166,t2167,t2168,t2169,t2174,t2183,t2187,t2193,t2194,t2195,t2199,t22,t2203,t2215,t2219,t2222,t2223,t2239,t2240,t2256,t2257,t2291,t2292,t2293,t2294,t2295,t2296,t2297,t2298,t2299,t2301,t2302,t2303,t2304,t2306,t2307,t2308,t2310,t2311,t2317,t2320,t2323,t2324,t2325,t2326,t2329,t2337,t2338,t2339,t2341,t2342,t2343,t2344,t2352,t2353,t2355,t2358,t2359,t236,t2360,t2361,t2362,t2363,t2364,t2365,t2366,t2367,t2368,t2369,t237,t2370,t2371,t2378,t2379,t238,t2380,t2384,t2388,t2389,t2391,t2394,t2395,t2397,t2398,t2399,t24,t2400,t2401,t2402,t2403,t2404,t2405,t241,t2413,t2414,t2419,t2421,t2422,t2423,t2433,t2434,t2438,t2447,t2448,t2449,t2450,t2459,t2460,t2461,t2471,t2472,t2492,t2493,t2494,t25,t2502,t2508,t2510,t2515,t2519,t2527,t2529,t2530,t2534,t2539,t2555,t2556,t2572,t2575,t2583,t2598,t26,t2605,t2606,t2612,t2613,t2618,t2619,t262,t2638,t264,t2651,t2652,t2664,t2670,t2671,t2673,t2674,t2675,t2676,t2678,t2680,t2681,t2683,t2684,t2685,t2686,t2687,t2689,t2690,t2692,t2693,t2694,t2695,t2696,t2697,t2698,t27,t2700,t2701,t2704,t2705,t2707,t2708,t2709,t2711,t2712,t2713,t2715,t2716,t2717,t2719,t2720,t2721,t2735,t2736,t2740,t2742,t2744,t2745,t2747,t2748,t2749,t2750,t2754,t2759,t2769,t2773,t2774,t2775,t2777,t2778,t2779,t2781,t2785,t2786,t2787,t2788,t2790,t2797,t28,t2801,t2803,t2804,t2807,t2808,t2813,t2814,t2820,t2823,t2828,t2831,t2834,t2835,t2838,t2850,t2851,t29,t2927,t2937,t2941,t2942,t2945,t2946,t2947,t2950,t2951,t2953,t2954,t2955,t2956,t2957,t2963,t2964,t2965,t2966,t2969,t2970,t2975,t2978,t2979,t2984,t2985,t2986,t2987,t2990,t2991,t2993,t2994,t2998,t30,t3003,t3004,t3006,t3008,t3009,t3010,t3015,t3016,t3017,t3018,t3019,t3022,t3027,t3029,t3030,t3031,t3036,t3043,t3044,t3045,t3047,t3049,t3050,t3051,t3054,t3055,t3057,t3058,t3063,t3064,t3065,t3066,t3067,t3068,t3072,t3073,t3074,t3075,t3076,t3077,t3078,t3079,t3080,t3081,t3082,t3083,t3085,t3086,t3087,t3088,t3096,t3097,t31,t3109,t3117,t3118,t3121,t3122,t3126,t3129,t313,t3130,t3131,t3132,t3133,t3134,t3135,t3136,t314,t3140,t3141,t3142,t3143,t3145,t3148,t3150,t3153,t3154,t3156,t3157,t3158,t3159,t3160,t3161,t3162,t3163,t3164,t3165,t3167,t3171,t3172,t3173,t3179,t3180,t3181,t3185,t3187,t3188,t3189,t3190,t3192,t3193,t3194,t3195,t3196,t3198,t3199,t32,t3200,t3201,t3202,t3203,t3205,t3206,t3208,t3209,t321,t3211,t3213,t3216,t3217,t3219,t322,t3221,t3225,t3227,t3230,t3231,t3232,t3233,t3234,t3235,t3236,t3237,t3238,t3239,t3242,t3245,t3251,t3252,t3253,t3254,t3255,t3256,t3257,t3259,t326,t3260,t3261,t3263,t3265,t3266,t3267,t3268,t3269,t3270,t3271,t3272,t3273,t3276,t3277,t3278,t3279,t328,t3282,t3283,t3284,t3285,t3287,t3288,t3289,t329,t3290,t3291,t3293,t3294,t3295,t3296,t3297,t3298,t3299,t33,t330,t3300,t3301,t3302,t3303,t3304,t3305,t3307,t3309,t331,t3310,t3312,t3313,t3314,t3315,t3316,t3317,t3318,t332,t3322,t3324,t3326,t3328,t3329,t333,t3331,t3332,t3333,t3334,t3335,t3336,t3337,t3338,t3340,t3341,t3343,t3344,t3345,t3346,t3347,t3348,t335,t3350,t3351,t3352,t3353,t3354,t3355,t3356,t3357,t3358,t3359,t3361,t3363,t3364,t3365,t3366,t3367,t3368,t3369,t3370,t3377,t3379,t338,t3383,t3386,t3387,t3389,t339,t3392,t3393,t3394,t3395,t3396,t3398,t3399,t34,t3402,t3405,t3407,t3409,t341,t3410,t3411,t3414,t3415,t3416,t3419,t3420,t3421,t3423,t3424,t3425,t3426,t3428,t343,t3430,t3431,t3432,t3433,t3434,t3435,t3438,t3439,t3440,t3441,t3443,t3444,t3445,t3446,t3447,t3448,t3449,t3451,t3452,t3453,t3454,t3455,t3456,t3457,t3458,t346,t3460,t3461,t3462,t3463,t3464,t3465,t3467,t3468,t3469,t3470,t3471,t3474,t3475,t3480,t3482,t3483,t3488,t3489,t3490,t3492,t3495,t3496,t3498,t3499,t35,t350,t3500,t3502,t3503,t3508,t3509,t351,t3510,t3512,t3516,t3517,t3519,t352,t3520,t3521,t3522,t3524,t3526,t3527,t3529,t3530,t3531,t3532,t3534,t3535,t354,t3541,t3543,t3545,t3546,t3547,t3549,t3550,t3551,t3552,t3554,t3558,t356,t3560,t3561,t3562,t3563,t3565,t3566,t3568,t3569,t3572,t3573,t3575,t3576,t3577,t3578,t358,t3580,t3581,t3582,t3583,t3585,t3586,t3587,t3588,t359,t3590,t3591,t3592,t3593,t3594,t3595,t3596,t3597,t3598,t3599,t36,t360,t3600,t3601,t3602,t3603,t3605,t3606,t3607,t3608,t3609,t3610,t3611,t3612,t3614,t3615,t3616,t3618,t3619,t362,t3622,t3623,t3624,t3625,t3626,t3627,t3628,t3629,t363,t3634,t3636,t3637,t3638,t3639,t364,t3640,t3641,t3642,t3643,t3644,t3645,t3646,t3647,t3648,t3649,t365,t3650,t3651,t3652,t3653,t3654,t3655,t3656,t3657,t3658,t3659,t366,t3661,t3663,t3664,t3665,t3666,t3668,t3669,t3670,t3671,t3673,t3676,t3677,t3678,t3679,t3680,t3681,t3682,t3683,t3688,t3689,t369,t3690,t3692,t3693,t3695,t3696,t3697,t3699,t370,t3700,t3701,t3702,t3703,t3704,t3705,t3706,t3707,t3708,t3709,t371,t3710,t3711,t3712,t3713,t3715,t3716,t3717,t3718,t3719,t372,t3721,t3722,t3723,t3724,t3726,t3728,t3729,t3731,t3732,t3733,t3734,t3735,t3736,t3737,t3738,t3739,t3740,t3742,t3743,t3744,t3745,t3746,t3747,t3748,t3750,t3752,t3755,t3759,t3760,t3761,t3762,t3763,t3764,t3765,t3766,t3770,t3771,t3772,t3774,t3775,t3777,t3779,t378,t3781,t3782,t3783,t3784,t3785,t3786,t3788,t3789,t3790,t3791,t3792,t3793,t3794,t3795,t3796,t3797,t3798,t38,t380,t3800,t3801,t3802,t3804,t3805,t3808,t3809,t3810,t3812,t3813,t3814,t3815,t3817,t3818,t3819,t382,t3820,t3821,t3823,t3824,t3826,t3827,t3828,t3830,t3832,t3833,t3834,t3835,t3836,t3840,t3843,t3844,t3845,t3846,t3848,t3850,t3851,t3852,t3853,t3854,t3855,t3856,t3857,t3859,t3862,t3863,t3865,t3866,t3867,t3868,t387,t3870,t3871,t3872,t3873,t3874,t3876,t3877,t3878,t3879,t3880,t3881,t3882,t3883,t3884,t3885,t3887,t3888,t3889,t3890,t3891,t3893,t3894,t3895,t3896,t3897,t3898,t3899,t39,t3900,t3901,t3902,t3903,t3906,t3908,t3909,t3910,t3913,t3915,t3919,t3924,t3925,t3926,t3928,t3930,t3931,t3934,t3937,t3939,t3941,t3943,t3949,t3950,t3951,t3953,t3954,t3957,t3958,t3959,t3961,t3966,t3967,t3968,t3970,t3971,t3973,t3974,t3975,t3976,t3977,t3979,t3980,t3983,t3984,t3985,t3987,t3988,t3989,t3990,t3991,t3992,t3993,t3994,t3996,t3998,t3999,t4000,t4002,t4004,t4005,t4008,t4010,t4011,t4012,t4014,t4015,t4016,t4017,t4018,t4019,t4024,t4025,t4026,t4030,t4032,t4034,t4035,t4036,t4038,t4039,t4041,t4042,t4047,t4050,t4061,t4062,t4065,t4066,t4069,t4070,t4071,t4077,t4079,t4083,t4084,t4086,t4087,t4088,t4089,t4090,t4091,t4092,t4093,t4095,t4096,t4097,t4098,t4099,t410,t4100,t4101,t4102,t4103,t4105,t4107,t4108,t4116,t4117,t4118,t4125,t4126,t4139,t4144,t4146,t4147,t4149,t4151,t4153,t4154,t4160,t4163,t4165,t4169,t4171,t4172,t4173,t4174,t4178,t4181,t4187,t4188,t4189,t4190,t4193,t4195,t4198,t4199,t42,t4200,t4201,t4204,t4205,t4207,t4208,t4210,t4213,t4215,t4217,t4218,t4219,t4222,t4223,t4224,t4226,t4228,t4229,t4230,t4236,t4237,t4240,t4241,t4243,t4244,t4246,t4247,t4248,t4249,t4251,t4255,t4256,t4258,t4260,t4261,t4262,t4263,t4264,t4266,t4270,t4271,t4272,t4273,t4274,t4275,t4276,t4277,t4278,t4279,t4280,t4281,t4282,t4283,t4286,t4287,t4288,t4289,t429,t4290,t4293,t4294,t4295,t4296,t4297,t4298,t4299,t43,t4300,t4301,t4303,t4304,t4305,t4306,t4307,t4308,t4310,t4311,t4312,t4313,t4314,t4318,t4319,t4322,t4323,t4324,t4325,t4326,t4328,t4330,t4331,t4332,t4333,t4334,t4335,t4337,t4339,t4340,t4341,t4342,t4343,t4344,t4346,t4347,t4348,t4352,t4353,t4354,t4356,t4358,t4362,t4365,t4366,t4371,t4372,t4373,t4374,t4375,t4376,t4377,t4378,t4379,t4380,t4386,t4387,t4388,t4389,t4394,t4396,t4401,t4402,t4403,t4404,t4405,t4406,t4410,t4413,t4414,t4415,t4416,t4417,t4420,t4422,t4423,t4424,t4425,t4426,t4455,t4456,t4457,t4458,t4459,t4460,t4462,t4464,t4465,t4466,t4467,t4468,t4470,t4471,t4472,t4476,t4477,t4478,t4479,t4480,t4481,t4482,t4485,t4486,t4487,t4488,t4489,t4491,t4492,t4493,t4494,t4495,t4496,t4497,t4498,t4499,t4500,t4501,t4502,t4503,t4504,t4507,t4508,t4509,t4510,t4511,t4513,t4515,t4516,t4517,t4518,t4519,t4520,t4521,t4522,t4523,t4524,t4525,t4528,t4529,t4530,t4531,t4532,t4533,t4534,t4535,t4536,t4537,t4538,t4540,t4541,t4542,t4543,t4544,t4545,t4546,t4548,t4549,t4550,t4551,t4554,t4559,t4561,t4563,t4570,t4571,t4572,t4575,t4576,t4578,t46,t4637,t4643,t4644,t4645,t4646,t4650,t4651,t4652,t4654,t4656,t4657,t4659,t4663,t4665,t4667,t4669,t4670,t4671,t4673,t4674,t4675,t4677,t4678,t4680,t4683,t4684,t4687,t47,t4703,t4704,t4705,t4708,t4709,t4711,t4713,t4716,t4719,t4722,t4724,t4725,t4726,t4727,t4728,t4730,t4734,t4737,t4739,t4741,t4742,t4743,t4744,t4746,t4747,t4751,t4753,t4755,t4756,t4757,t4760,t4761,t4762,t4763,t4774,t4814,t4820,t4826,t4828,t4833,t4835,t4838,t4839,t4840,t4843,t4844,t4845,t4847,t4848,t4849,t4850,t4853,t4872,t4874,t4877,t4878,t4879,t4880,t4884,t4885,t4886,t4890,t4891,t4892,t4893,t4895,t4902,t4915,t4916,t4917,t4920,t4923,t4924,t4925,t4926,t4927,t4929,t4930,t4942,t4944,t50,t5012,t5013,t5014,t5016,t5025,t5027,t5028,t5033,t5034,t5036,t5037,t5038,t5045,t5046,t5047,t5048,t5050,t5052,t5053,t5059,t5060,t5062,t5063,t5064,t5066,t5067,t5069,t5070,t5072,t5073,t5075,t5077,t5079,t5080,t5081,t5082,t5084,t5085,t5086,t5087,t5088,t5089,t5090,t5091,t5093,t5094,t5095,t5096,t5097,t5098,t5108,t5111,t5113,t5114,t5119,t5140,t5142,t5144,t5146,t5165,t5168,t5171,t5173,t5174,t5176,t5177,t5178,t5180,t5181,t5194,t5195,t5196,t5197,t5198,t5202,t5203,t5209,t5210,t5213,t5214,t5215,t5217,t5218,t5219,t5240,t5246,t5247,t5251,t5254,t5255,t5256,t5257,t5260,t5261,t5262,t5274,t5276,t5277,t5278,t5279,t5280,t5281,t5283,t5284,t5285,t5286,t5287,t5288,t5289,t5290,t5291,t5292,t5293,t5294,t5295,t5296,t5297,t5298,t5300,t5301,t5302,t5303,t5304,t5305,t5308,t5309,t5310,t5312,t5315,t5320,t5321,t5350,t5356,t5357,t5361,t5363,t5370,t5372,t5381,t5391,t5392,t5393,t5395,t5399,t5400,t5401,t5402,t5403,t5404,t5415,t5416,t5433,t5434,t5436,t5437,t5438,t5439,t5444,t5445,t5446,t5448,t5452,t5456,t5457,t5458,t5459,t5460,t5464,t5481,t5485,t5487,t5488,t5494,t5495,t5499,t5513,t5516,t5517,t5520,t5535,t5536,t5537,t5538,t5539,t5540,t5541,t5542,t5543,t5544,t5545,t5548,t5549,t5550,t5555,t5556,t5560,t5561,t5565,t5566,t5568,t5569,t5570,t5575,t5576,t5586,t5590,t56,t5604,t5605,t5607,t5608,t5609,t5611,t5612,t5660,t5678,t5684,t5730,t5731,t5734,t5735,t5738,t5739,t5741,t5742,t5758,t5759,t5760,t5761,t5779,t5782,t5783,t58,t5803,t5849,t5896,t59,t5901,t5902,t5903,t5916,t5917,t5938,t5941,t5954,t5955,t5990,t60,t6002,t6011,t6013,t6014,t6050,t6062,t6074,t6143,t6255,t6256,t6257,t6271,t628,t635,t636,t638,t6394,t640,t641,t642,t643,t6442,t649,t654,t655,t656,t6564,t6565,t657,t6574,t6588,t659,t660,t6622,t6623,t663,t664,t665,t667,t668,t669,t67,t670,t672,t673,t674,t6745,t675,t6751,t676,t677,t678,t679,t68,t681,t682,t684,t685,t686,t687,t689,t691,t6919,t692,t6920,t693,t694,t6987,t70,t7005,t702,t707,t708,t71,t710,t7117,t7141,t715,t7150,t716,t717,t718,t721,t722,t724,t725,t73,t7304,t736,t738,t740,t741,t749,t756,t76,t762,t768,t777,t792,t793,t8,t801,t802,t808,t813,t819,t821,t850,t855,t874,t878,t89,t9,t90,t91,t92,t941,t944,t948,t951,t97});
end
function tau_c = ft_10(ct)
dq1 = ct{1};
dq2 = ct{2};
dq3 = ct{3};
dq4 = ct{4};
dq5 = ct{5};
dq6 = ct{6};
t10 = ct{7};
t1005 = ct{8};
t1022 = ct{9};
t1089 = ct{10};
t11 = ct{11};
t1104 = ct{12};
t1105 = ct{13};
t1108 = ct{14};
t1115 = ct{15};
t1121 = ct{16};
t1158 = ct{17};
t1159 = ct{18};
t1190 = ct{19};
t1196 = ct{20};
t12 = ct{21};
t1205 = ct{22};
t1207 = ct{23};
t1208 = ct{24};
t1210 = ct{25};
t1212 = ct{26};
t1214 = ct{27};
t1217 = ct{28};
t1218 = ct{29};
t1219 = ct{30};
t1220 = ct{31};
t1221 = ct{32};
t123 = ct{33};
t1230 = ct{34};
t1235 = ct{35};
t1237 = ct{36};
t1238 = ct{37};
t1288 = ct{38};
t1289 = ct{39};
t13 = ct{40};
t1302 = ct{41};
t1303 = ct{42};
t1319 = ct{43};
t1320 = ct{44};
t1336 = ct{45};
t1348 = ct{46};
t1350 = ct{47};
t1351 = ct{48};
t1360 = ct{49};
t1369 = ct{50};
t1378 = ct{51};
t1396 = ct{52};
t14 = ct{53};
t140 = ct{54};
t1425 = ct{55};
t1435 = ct{56};
t1456 = ct{57};
t1477 = ct{58};
t1488 = ct{59};
t15 = ct{60};
t1513 = ct{61};
t1539 = ct{62};
t1544 = ct{63};
t1547 = ct{64};
t1548 = ct{65};
t1553 = ct{66};
t1554 = ct{67};
t1559 = ct{68};
t1564 = ct{69};
t1576 = ct{70};
t1577 = ct{71};
t1578 = ct{72};
t1579 = ct{73};
t1581 = ct{74};
t1584 = ct{75};
t1585 = ct{76};
t1586 = ct{77};
t1587 = ct{78};
t1591 = ct{79};
t1595 = ct{80};
t1596 = ct{81};
t1598 = ct{82};
t1599 = ct{83};
t16 = ct{84};
t1600 = ct{85};
t1601 = ct{86};
t1602 = ct{87};
t1604 = ct{88};
t1605 = ct{89};
t1606 = ct{90};
t1607 = ct{91};
t1608 = ct{92};
t1609 = ct{93};
t1612 = ct{94};
t1613 = ct{95};
t1614 = ct{96};
t1615 = ct{97};
t1616 = ct{98};
t1626 = ct{99};
t1627 = ct{100};
t1628 = ct{101};
t1629 = ct{102};
t1631 = ct{103};
t1637 = ct{104};
t1640 = ct{105};
t1641 = ct{106};
t1648 = ct{107};
t1649 = ct{108};
t1659 = ct{109};
t1660 = ct{110};
t1661 = ct{111};
t1666 = ct{112};
t1667 = ct{113};
t1683 = ct{114};
t1686 = ct{115};
t1690 = ct{116};
t1692 = ct{117};
t17 = ct{118};
t1700 = ct{119};
t1701 = ct{120};
t1703 = ct{121};
t1704 = ct{122};
t1705 = ct{123};
t1712 = ct{124};
t1717 = ct{125};
t1738 = ct{126};
t1741 = ct{127};
t1742 = ct{128};
t1750 = ct{129};
t1752 = ct{130};
t1753 = ct{131};
t1754 = ct{132};
t1758 = ct{133};
t1759 = ct{134};
t1775 = ct{135};
t1776 = ct{136};
t18 = ct{137};
t1861 = ct{138};
t1874 = ct{139};
t1879 = ct{140};
t188 = ct{141};
t1881 = ct{142};
t189 = ct{143};
t1896 = ct{144};
t19 = ct{145};
t1901 = ct{146};
t1941 = ct{147};
t1953 = ct{148};
t1959 = ct{149};
t1973 = ct{150};
t1993 = ct{151};
t1994 = ct{152};
t20 = ct{153};
t201 = ct{154};
t202 = ct{155};
t2023 = ct{156};
t2053 = ct{157};
t2060 = ct{158};
t2089 = ct{159};
t2090 = ct{160};
t2098 = ct{161};
t2099 = ct{162};
t21 = ct{163};
t2117 = ct{164};
t2120 = ct{165};
t2122 = ct{166};
t2123 = ct{167};
t2125 = ct{168};
t2137 = ct{169};
t2139 = ct{170};
t2140 = ct{171};
t2142 = ct{172};
t2145 = ct{173};
t2146 = ct{174};
t2147 = ct{175};
t2149 = ct{176};
t2150 = ct{177};
t2151 = ct{178};
t2152 = ct{179};
t2153 = ct{180};
t2154 = ct{181};
t2155 = ct{182};
t2159 = ct{183};
t2162 = ct{184};
t2164 = ct{185};
t2165 = ct{186};
t2166 = ct{187};
t2167 = ct{188};
t2168 = ct{189};
t2169 = ct{190};
t2174 = ct{191};
t2183 = ct{192};
t2187 = ct{193};
t2193 = ct{194};
t2194 = ct{195};
t2195 = ct{196};
t2199 = ct{197};
t22 = ct{198};
t2203 = ct{199};
t2215 = ct{200};
t2219 = ct{201};
t2222 = ct{202};
t2223 = ct{203};
t2239 = ct{204};
t2240 = ct{205};
t2256 = ct{206};
t2257 = ct{207};
t2291 = ct{208};
t2292 = ct{209};
t2293 = ct{210};
t2294 = ct{211};
t2295 = ct{212};
t2296 = ct{213};
t2297 = ct{214};
t2298 = ct{215};
t2299 = ct{216};
t2301 = ct{217};
t2302 = ct{218};
t2303 = ct{219};
t2304 = ct{220};
t2306 = ct{221};
t2307 = ct{222};
t2308 = ct{223};
t2310 = ct{224};
t2311 = ct{225};
t2317 = ct{226};
t2320 = ct{227};
t2323 = ct{228};
t2324 = ct{229};
t2325 = ct{230};
t2326 = ct{231};
t2329 = ct{232};
t2337 = ct{233};
t2338 = ct{234};
t2339 = ct{235};
t2341 = ct{236};
t2342 = ct{237};
t2343 = ct{238};
t2344 = ct{239};
t2352 = ct{240};
t2353 = ct{241};
t2355 = ct{242};
t2358 = ct{243};
t2359 = ct{244};
t236 = ct{245};
t2360 = ct{246};
t2361 = ct{247};
t2362 = ct{248};
t2363 = ct{249};
t2364 = ct{250};
t2365 = ct{251};
t2366 = ct{252};
t2367 = ct{253};
t2368 = ct{254};
t2369 = ct{255};
t237 = ct{256};
t2370 = ct{257};
t2371 = ct{258};
t2378 = ct{259};
t2379 = ct{260};
t238 = ct{261};
t2380 = ct{262};
t2384 = ct{263};
t2388 = ct{264};
t2389 = ct{265};
t2391 = ct{266};
t2394 = ct{267};
t2395 = ct{268};
t2397 = ct{269};
t2398 = ct{270};
t2399 = ct{271};
t24 = ct{272};
t2400 = ct{273};
t2401 = ct{274};
t2402 = ct{275};
t2403 = ct{276};
t2404 = ct{277};
t2405 = ct{278};
t241 = ct{279};
t2413 = ct{280};
t2414 = ct{281};
t2419 = ct{282};
t2421 = ct{283};
t2422 = ct{284};
t2423 = ct{285};
t2433 = ct{286};
t2434 = ct{287};
t2438 = ct{288};
t2447 = ct{289};
t2448 = ct{290};
t2449 = ct{291};
t2450 = ct{292};
t2459 = ct{293};
t2460 = ct{294};
t2461 = ct{295};
t2471 = ct{296};
t2472 = ct{297};
t2492 = ct{298};
t2493 = ct{299};
t2494 = ct{300};
t25 = ct{301};
t2502 = ct{302};
t2508 = ct{303};
t2510 = ct{304};
t2515 = ct{305};
t2519 = ct{306};
t2527 = ct{307};
t2529 = ct{308};
t2530 = ct{309};
t2534 = ct{310};
t2539 = ct{311};
t2555 = ct{312};
t2556 = ct{313};
t2572 = ct{314};
t2575 = ct{315};
t2583 = ct{316};
t2598 = ct{317};
t26 = ct{318};
t2605 = ct{319};
t2606 = ct{320};
t2612 = ct{321};
t2613 = ct{322};
t2618 = ct{323};
t2619 = ct{324};
t262 = ct{325};
t2638 = ct{326};
t264 = ct{327};
t2651 = ct{328};
t2652 = ct{329};
t2664 = ct{330};
t2670 = ct{331};
t2671 = ct{332};
t2673 = ct{333};
t2674 = ct{334};
t2675 = ct{335};
t2676 = ct{336};
t2678 = ct{337};
t2680 = ct{338};
t2681 = ct{339};
t2683 = ct{340};
t2684 = ct{341};
t2685 = ct{342};
t2686 = ct{343};
t2687 = ct{344};
t2689 = ct{345};
t2690 = ct{346};
t2692 = ct{347};
t2693 = ct{348};
t2694 = ct{349};
t2695 = ct{350};
t2696 = ct{351};
t2697 = ct{352};
t2698 = ct{353};
t27 = ct{354};
t2700 = ct{355};
t2701 = ct{356};
t2704 = ct{357};
t2705 = ct{358};
t2707 = ct{359};
t2708 = ct{360};
t2709 = ct{361};
t2711 = ct{362};
t2712 = ct{363};
t2713 = ct{364};
t2715 = ct{365};
t2716 = ct{366};
t2717 = ct{367};
t2719 = ct{368};
t2720 = ct{369};
t2721 = ct{370};
t2735 = ct{371};
t2736 = ct{372};
t2740 = ct{373};
t2742 = ct{374};
t2744 = ct{375};
t2745 = ct{376};
t2747 = ct{377};
t2748 = ct{378};
t2749 = ct{379};
t2750 = ct{380};
t2754 = ct{381};
t2759 = ct{382};
t2769 = ct{383};
t2773 = ct{384};
t2774 = ct{385};
t2775 = ct{386};
t2777 = ct{387};
t2778 = ct{388};
t2779 = ct{389};
t2781 = ct{390};
t2785 = ct{391};
t2786 = ct{392};
t2787 = ct{393};
t2788 = ct{394};
t2790 = ct{395};
t2797 = ct{396};
t28 = ct{397};
t2801 = ct{398};
t2803 = ct{399};
t2804 = ct{400};
t2807 = ct{401};
t2808 = ct{402};
t2813 = ct{403};
t2814 = ct{404};
t2820 = ct{405};
t2823 = ct{406};
t2828 = ct{407};
t2831 = ct{408};
t2834 = ct{409};
t2835 = ct{410};
t2838 = ct{411};
t2850 = ct{412};
t2851 = ct{413};
t29 = ct{414};
t2927 = ct{415};
t2937 = ct{416};
t2941 = ct{417};
t2942 = ct{418};
t2945 = ct{419};
t2946 = ct{420};
t2947 = ct{421};
t2950 = ct{422};
t2951 = ct{423};
t2953 = ct{424};
t2954 = ct{425};
t2955 = ct{426};
t2956 = ct{427};
t2957 = ct{428};
t2963 = ct{429};
t2964 = ct{430};
t2965 = ct{431};
t2966 = ct{432};
t2969 = ct{433};
t2970 = ct{434};
t2975 = ct{435};
t2978 = ct{436};
t2979 = ct{437};
t2984 = ct{438};
t2985 = ct{439};
t2986 = ct{440};
t2987 = ct{441};
t2990 = ct{442};
t2991 = ct{443};
t2993 = ct{444};
t2994 = ct{445};
t2998 = ct{446};
t30 = ct{447};
t3003 = ct{448};
t3004 = ct{449};
t3006 = ct{450};
t3008 = ct{451};
t3009 = ct{452};
t3010 = ct{453};
t3015 = ct{454};
t3016 = ct{455};
t3017 = ct{456};
t3018 = ct{457};
t3019 = ct{458};
t3022 = ct{459};
t3027 = ct{460};
t3029 = ct{461};
t3030 = ct{462};
t3031 = ct{463};
t3036 = ct{464};
t3043 = ct{465};
t3044 = ct{466};
t3045 = ct{467};
t3047 = ct{468};
t3049 = ct{469};
t3050 = ct{470};
t3051 = ct{471};
t3054 = ct{472};
t3055 = ct{473};
t3057 = ct{474};
t3058 = ct{475};
t3063 = ct{476};
t3064 = ct{477};
t3065 = ct{478};
t3066 = ct{479};
t3067 = ct{480};
t3068 = ct{481};
t3072 = ct{482};
t3073 = ct{483};
t3074 = ct{484};
t3075 = ct{485};
t3076 = ct{486};
t3077 = ct{487};
t3078 = ct{488};
t3079 = ct{489};
t3080 = ct{490};
t3081 = ct{491};
t3082 = ct{492};
t3083 = ct{493};
t3085 = ct{494};
t3086 = ct{495};
t3087 = ct{496};
t3088 = ct{497};
t3096 = ct{498};
t3097 = ct{499};
t31 = ct{500};
t3109 = ct{501};
t3117 = ct{502};
t3118 = ct{503};
t3121 = ct{504};
t3122 = ct{505};
t3126 = ct{506};
t3129 = ct{507};
t313 = ct{508};
t3130 = ct{509};
t3131 = ct{510};
t3132 = ct{511};
t3133 = ct{512};
t3134 = ct{513};
t3135 = ct{514};
t3136 = ct{515};
t314 = ct{516};
t3140 = ct{517};
t3141 = ct{518};
t3142 = ct{519};
t3143 = ct{520};
t3145 = ct{521};
t3148 = ct{522};
t3150 = ct{523};
t3153 = ct{524};
t3154 = ct{525};
t3156 = ct{526};
t3157 = ct{527};
t3158 = ct{528};
t3159 = ct{529};
t3160 = ct{530};
t3161 = ct{531};
t3162 = ct{532};
t3163 = ct{533};
t3164 = ct{534};
t3165 = ct{535};
t3167 = ct{536};
t3171 = ct{537};
t3172 = ct{538};
t3173 = ct{539};
t3179 = ct{540};
t3180 = ct{541};
t3181 = ct{542};
t3185 = ct{543};
t3187 = ct{544};
t3188 = ct{545};
t3189 = ct{546};
t3190 = ct{547};
t3192 = ct{548};
t3193 = ct{549};
t3194 = ct{550};
t3195 = ct{551};
t3196 = ct{552};
t3198 = ct{553};
t3199 = ct{554};
t32 = ct{555};
t3200 = ct{556};
t3201 = ct{557};
t3202 = ct{558};
t3203 = ct{559};
t3205 = ct{560};
t3206 = ct{561};
t3208 = ct{562};
t3209 = ct{563};
t321 = ct{564};
t3211 = ct{565};
t3213 = ct{566};
t3216 = ct{567};
t3217 = ct{568};
t3219 = ct{569};
t322 = ct{570};
t3221 = ct{571};
t3225 = ct{572};
t3227 = ct{573};
t3230 = ct{574};
t3231 = ct{575};
t3232 = ct{576};
t3233 = ct{577};
t3234 = ct{578};
t3235 = ct{579};
t3236 = ct{580};
t3237 = ct{581};
t3238 = ct{582};
t3239 = ct{583};
t3242 = ct{584};
t3245 = ct{585};
t3251 = ct{586};
t3252 = ct{587};
t3253 = ct{588};
t3254 = ct{589};
t3255 = ct{590};
t3256 = ct{591};
t3257 = ct{592};
t3259 = ct{593};
t326 = ct{594};
t3260 = ct{595};
t3261 = ct{596};
t3263 = ct{597};
t3265 = ct{598};
t3266 = ct{599};
t3267 = ct{600};
t3268 = ct{601};
t3269 = ct{602};
t3270 = ct{603};
t3271 = ct{604};
t3272 = ct{605};
t3273 = ct{606};
t3276 = ct{607};
t3277 = ct{608};
t3278 = ct{609};
t3279 = ct{610};
t328 = ct{611};
t3282 = ct{612};
t3283 = ct{613};
t3284 = ct{614};
t3285 = ct{615};
t3287 = ct{616};
t3288 = ct{617};
t3289 = ct{618};
t329 = ct{619};
t3290 = ct{620};
t3291 = ct{621};
t3293 = ct{622};
t3294 = ct{623};
t3295 = ct{624};
t3296 = ct{625};
t3297 = ct{626};
t3298 = ct{627};
t3299 = ct{628};
t33 = ct{629};
t330 = ct{630};
t3300 = ct{631};
t3301 = ct{632};
t3302 = ct{633};
t3303 = ct{634};
t3304 = ct{635};
t3305 = ct{636};
t3307 = ct{637};
t3309 = ct{638};
t331 = ct{639};
t3310 = ct{640};
t3312 = ct{641};
t3313 = ct{642};
t3314 = ct{643};
t3315 = ct{644};
t3316 = ct{645};
t3317 = ct{646};
t3318 = ct{647};
t332 = ct{648};
t3322 = ct{649};
t3324 = ct{650};
t3326 = ct{651};
t3328 = ct{652};
t3329 = ct{653};
t333 = ct{654};
t3331 = ct{655};
t3332 = ct{656};
t3333 = ct{657};
t3334 = ct{658};
t3335 = ct{659};
t3336 = ct{660};
t3337 = ct{661};
t3338 = ct{662};
t3340 = ct{663};
t3341 = ct{664};
t3343 = ct{665};
t3344 = ct{666};
t3345 = ct{667};
t3346 = ct{668};
t3347 = ct{669};
t3348 = ct{670};
t335 = ct{671};
t3350 = ct{672};
t3351 = ct{673};
t3352 = ct{674};
t3353 = ct{675};
t3354 = ct{676};
t3355 = ct{677};
t3356 = ct{678};
t3357 = ct{679};
t3358 = ct{680};
t3359 = ct{681};
t3361 = ct{682};
t3363 = ct{683};
t3364 = ct{684};
t3365 = ct{685};
t3366 = ct{686};
t3367 = ct{687};
t3368 = ct{688};
t3369 = ct{689};
t3370 = ct{690};
t3377 = ct{691};
t3379 = ct{692};
t338 = ct{693};
t3383 = ct{694};
t3386 = ct{695};
t3387 = ct{696};
t3389 = ct{697};
t339 = ct{698};
t3392 = ct{699};
t3393 = ct{700};
t3394 = ct{701};
t3395 = ct{702};
t3396 = ct{703};
t3398 = ct{704};
t3399 = ct{705};
t34 = ct{706};
t3402 = ct{707};
t3405 = ct{708};
t3407 = ct{709};
t3409 = ct{710};
t341 = ct{711};
t3410 = ct{712};
t3411 = ct{713};
t3414 = ct{714};
t3415 = ct{715};
t3416 = ct{716};
t3419 = ct{717};
t3420 = ct{718};
t3421 = ct{719};
t3423 = ct{720};
t3424 = ct{721};
t3425 = ct{722};
t3426 = ct{723};
t3428 = ct{724};
t343 = ct{725};
t3430 = ct{726};
t3431 = ct{727};
t3432 = ct{728};
t3433 = ct{729};
t3434 = ct{730};
t3435 = ct{731};
t3438 = ct{732};
t3439 = ct{733};
t3440 = ct{734};
t3441 = ct{735};
t3443 = ct{736};
t3444 = ct{737};
t3445 = ct{738};
t3446 = ct{739};
t3447 = ct{740};
t3448 = ct{741};
t3449 = ct{742};
t3451 = ct{743};
t3452 = ct{744};
t3453 = ct{745};
t3454 = ct{746};
t3455 = ct{747};
t3456 = ct{748};
t3457 = ct{749};
t3458 = ct{750};
t346 = ct{751};
t3460 = ct{752};
t3461 = ct{753};
t3462 = ct{754};
t3463 = ct{755};
t3464 = ct{756};
t3465 = ct{757};
t3467 = ct{758};
t3468 = ct{759};
t3469 = ct{760};
t3470 = ct{761};
t3471 = ct{762};
t3474 = ct{763};
t3475 = ct{764};
t3480 = ct{765};
t3482 = ct{766};
t3483 = ct{767};
t3488 = ct{768};
t3489 = ct{769};
t3490 = ct{770};
t3492 = ct{771};
t3495 = ct{772};
t3496 = ct{773};
t3498 = ct{774};
t3499 = ct{775};
t35 = ct{776};
t350 = ct{777};
t3500 = ct{778};
t3502 = ct{779};
t3503 = ct{780};
t3508 = ct{781};
t3509 = ct{782};
t351 = ct{783};
t3510 = ct{784};
t3512 = ct{785};
t3516 = ct{786};
t3517 = ct{787};
t3519 = ct{788};
t352 = ct{789};
t3520 = ct{790};
t3521 = ct{791};
t3522 = ct{792};
t3524 = ct{793};
t3526 = ct{794};
t3527 = ct{795};
t3529 = ct{796};
t3530 = ct{797};
t3531 = ct{798};
t3532 = ct{799};
t3534 = ct{800};
t3535 = ct{801};
t354 = ct{802};
t3541 = ct{803};
t3543 = ct{804};
t3545 = ct{805};
t3546 = ct{806};
t3547 = ct{807};
t3549 = ct{808};
t3550 = ct{809};
t3551 = ct{810};
t3552 = ct{811};
t3554 = ct{812};
t3558 = ct{813};
t356 = ct{814};
t3560 = ct{815};
t3561 = ct{816};
t3562 = ct{817};
t3563 = ct{818};
t3565 = ct{819};
t3566 = ct{820};
t3568 = ct{821};
t3569 = ct{822};
t3572 = ct{823};
t3573 = ct{824};
t3575 = ct{825};
t3576 = ct{826};
t3577 = ct{827};
t3578 = ct{828};
t358 = ct{829};
t3580 = ct{830};
t3581 = ct{831};
t3582 = ct{832};
t3583 = ct{833};
t3585 = ct{834};
t3586 = ct{835};
t3587 = ct{836};
t3588 = ct{837};
t359 = ct{838};
t3590 = ct{839};
t3591 = ct{840};
t3592 = ct{841};
t3593 = ct{842};
t3594 = ct{843};
t3595 = ct{844};
t3596 = ct{845};
t3597 = ct{846};
t3598 = ct{847};
t3599 = ct{848};
t36 = ct{849};
t360 = ct{850};
t3600 = ct{851};
t3601 = ct{852};
t3602 = ct{853};
t3603 = ct{854};
t3605 = ct{855};
t3606 = ct{856};
t3607 = ct{857};
t3608 = ct{858};
t3609 = ct{859};
t3610 = ct{860};
t3611 = ct{861};
t3612 = ct{862};
t3614 = ct{863};
t3615 = ct{864};
t3616 = ct{865};
t3618 = ct{866};
t3619 = ct{867};
t362 = ct{868};
t3622 = ct{869};
t3623 = ct{870};
t3624 = ct{871};
t3625 = ct{872};
t3626 = ct{873};
t3627 = ct{874};
t3628 = ct{875};
t3629 = ct{876};
t363 = ct{877};
t3634 = ct{878};
t3636 = ct{879};
t3637 = ct{880};
t3638 = ct{881};
t3639 = ct{882};
t364 = ct{883};
t3640 = ct{884};
t3641 = ct{885};
t3642 = ct{886};
t3643 = ct{887};
t3644 = ct{888};
t3645 = ct{889};
t3646 = ct{890};
t3647 = ct{891};
t3648 = ct{892};
t3649 = ct{893};
t365 = ct{894};
t3650 = ct{895};
t3651 = ct{896};
t3652 = ct{897};
t3653 = ct{898};
t3654 = ct{899};
t3655 = ct{900};
t3656 = ct{901};
t3657 = ct{902};
t3658 = ct{903};
t3659 = ct{904};
t366 = ct{905};
t3661 = ct{906};
t3663 = ct{907};
t3664 = ct{908};
t3665 = ct{909};
t3666 = ct{910};
t3668 = ct{911};
t3669 = ct{912};
t3670 = ct{913};
t3671 = ct{914};
t3673 = ct{915};
t3676 = ct{916};
t3677 = ct{917};
t3678 = ct{918};
t3679 = ct{919};
t3680 = ct{920};
t3681 = ct{921};
t3682 = ct{922};
t3683 = ct{923};
t3688 = ct{924};
t3689 = ct{925};
t369 = ct{926};
t3690 = ct{927};
t3692 = ct{928};
t3693 = ct{929};
t3695 = ct{930};
t3696 = ct{931};
t3697 = ct{932};
t3699 = ct{933};
t370 = ct{934};
t3700 = ct{935};
t3701 = ct{936};
t3702 = ct{937};
t3703 = ct{938};
t3704 = ct{939};
t3705 = ct{940};
t3706 = ct{941};
t3707 = ct{942};
t3708 = ct{943};
t3709 = ct{944};
t371 = ct{945};
t3710 = ct{946};
t3711 = ct{947};
t3712 = ct{948};
t3713 = ct{949};
t3715 = ct{950};
t3716 = ct{951};
t3717 = ct{952};
t3718 = ct{953};
t3719 = ct{954};
t372 = ct{955};
t3721 = ct{956};
t3722 = ct{957};
t3723 = ct{958};
t3724 = ct{959};
t3726 = ct{960};
t3728 = ct{961};
t3729 = ct{962};
t3731 = ct{963};
t3732 = ct{964};
t3733 = ct{965};
t3734 = ct{966};
t3735 = ct{967};
t3736 = ct{968};
t3737 = ct{969};
t3738 = ct{970};
t3739 = ct{971};
t3740 = ct{972};
t3742 = ct{973};
t3743 = ct{974};
t3744 = ct{975};
t3745 = ct{976};
t3746 = ct{977};
t3747 = ct{978};
t3748 = ct{979};
t3750 = ct{980};
t3752 = ct{981};
t3755 = ct{982};
t3759 = ct{983};
t3760 = ct{984};
t3761 = ct{985};
t3762 = ct{986};
t3763 = ct{987};
t3764 = ct{988};
t3765 = ct{989};
t3766 = ct{990};
t3770 = ct{991};
t3771 = ct{992};
t3772 = ct{993};
t3774 = ct{994};
t3775 = ct{995};
t3777 = ct{996};
t3779 = ct{997};
t378 = ct{998};
t3781 = ct{999};
t3782 = ct{1000};
t3783 = ct{1001};
t3784 = ct{1002};
t3785 = ct{1003};
t3786 = ct{1004};
t3788 = ct{1005};
t3789 = ct{1006};
t3790 = ct{1007};
t3791 = ct{1008};
t3792 = ct{1009};
t3793 = ct{1010};
t3794 = ct{1011};
t3795 = ct{1012};
t3796 = ct{1013};
t3797 = ct{1014};
t3798 = ct{1015};
t38 = ct{1016};
t380 = ct{1017};
t3800 = ct{1018};
t3801 = ct{1019};
t3802 = ct{1020};
t3804 = ct{1021};
t3805 = ct{1022};
t3808 = ct{1023};
t3809 = ct{1024};
t3810 = ct{1025};
t3812 = ct{1026};
t3813 = ct{1027};
t3814 = ct{1028};
t3815 = ct{1029};
t3817 = ct{1030};
t3818 = ct{1031};
t3819 = ct{1032};
t382 = ct{1033};
t3820 = ct{1034};
t3821 = ct{1035};
t3823 = ct{1036};
t3824 = ct{1037};
t3826 = ct{1038};
t3827 = ct{1039};
t3828 = ct{1040};
t3830 = ct{1041};
t3832 = ct{1042};
t3833 = ct{1043};
t3834 = ct{1044};
t3835 = ct{1045};
t3836 = ct{1046};
t3840 = ct{1047};
t3843 = ct{1048};
t3844 = ct{1049};
t3845 = ct{1050};
t3846 = ct{1051};
t3848 = ct{1052};
t3850 = ct{1053};
t3851 = ct{1054};
t3852 = ct{1055};
t3853 = ct{1056};
t3854 = ct{1057};
t3855 = ct{1058};
t3856 = ct{1059};
t3857 = ct{1060};
t3859 = ct{1061};
t3862 = ct{1062};
t3863 = ct{1063};
t3865 = ct{1064};
t3866 = ct{1065};
t3867 = ct{1066};
t3868 = ct{1067};
t387 = ct{1068};
t3870 = ct{1069};
t3871 = ct{1070};
t3872 = ct{1071};
t3873 = ct{1072};
t3874 = ct{1073};
t3876 = ct{1074};
t3877 = ct{1075};
t3878 = ct{1076};
t3879 = ct{1077};
t3880 = ct{1078};
t3881 = ct{1079};
t3882 = ct{1080};
t3883 = ct{1081};
t3884 = ct{1082};
t3885 = ct{1083};
t3887 = ct{1084};
t3888 = ct{1085};
t3889 = ct{1086};
t3890 = ct{1087};
t3891 = ct{1088};
t3893 = ct{1089};
t3894 = ct{1090};
t3895 = ct{1091};
t3896 = ct{1092};
t3897 = ct{1093};
t3898 = ct{1094};
t3899 = ct{1095};
t39 = ct{1096};
t3900 = ct{1097};
t3901 = ct{1098};
t3902 = ct{1099};
t3903 = ct{1100};
t3906 = ct{1101};
t3908 = ct{1102};
t3909 = ct{1103};
t3910 = ct{1104};
t3913 = ct{1105};
t3915 = ct{1106};
t3919 = ct{1107};
t3924 = ct{1108};
t3925 = ct{1109};
t3926 = ct{1110};
t3928 = ct{1111};
t3930 = ct{1112};
t3931 = ct{1113};
t3934 = ct{1114};
t3937 = ct{1115};
t3939 = ct{1116};
t3941 = ct{1117};
t3943 = ct{1118};
t3949 = ct{1119};
t3950 = ct{1120};
t3951 = ct{1121};
t3953 = ct{1122};
t3954 = ct{1123};
t3957 = ct{1124};
t3958 = ct{1125};
t3959 = ct{1126};
t3961 = ct{1127};
t3966 = ct{1128};
t3967 = ct{1129};
t3968 = ct{1130};
t3970 = ct{1131};
t3971 = ct{1132};
t3973 = ct{1133};
t3974 = ct{1134};
t3975 = ct{1135};
t3976 = ct{1136};
t3977 = ct{1137};
t3979 = ct{1138};
t3980 = ct{1139};
t3983 = ct{1140};
t3984 = ct{1141};
t3985 = ct{1142};
t3987 = ct{1143};
t3988 = ct{1144};
t3989 = ct{1145};
t3990 = ct{1146};
t3991 = ct{1147};
t3992 = ct{1148};
t3993 = ct{1149};
t3994 = ct{1150};
t3996 = ct{1151};
t3998 = ct{1152};
t3999 = ct{1153};
t4000 = ct{1154};
t4002 = ct{1155};
t4004 = ct{1156};
t4005 = ct{1157};
t4008 = ct{1158};
t4010 = ct{1159};
t4011 = ct{1160};
t4012 = ct{1161};
t4014 = ct{1162};
t4015 = ct{1163};
t4016 = ct{1164};
t4017 = ct{1165};
t4018 = ct{1166};
t4019 = ct{1167};
t4024 = ct{1168};
t4025 = ct{1169};
t4026 = ct{1170};
t4030 = ct{1171};
t4032 = ct{1172};
t4034 = ct{1173};
t4035 = ct{1174};
t4036 = ct{1175};
t4038 = ct{1176};
t4039 = ct{1177};
t4041 = ct{1178};
t4042 = ct{1179};
t4047 = ct{1180};
t4050 = ct{1181};
t4061 = ct{1182};
t4062 = ct{1183};
t4065 = ct{1184};
t4066 = ct{1185};
t4069 = ct{1186};
t4070 = ct{1187};
t4071 = ct{1188};
t4077 = ct{1189};
t4079 = ct{1190};
t4083 = ct{1191};
t4084 = ct{1192};
t4086 = ct{1193};
t4087 = ct{1194};
t4088 = ct{1195};
t4089 = ct{1196};
t4090 = ct{1197};
t4091 = ct{1198};
t4092 = ct{1199};
t4093 = ct{1200};
t4095 = ct{1201};
t4096 = ct{1202};
t4097 = ct{1203};
t4098 = ct{1204};
t4099 = ct{1205};
t410 = ct{1206};
t4100 = ct{1207};
t4101 = ct{1208};
t4102 = ct{1209};
t4103 = ct{1210};
t4105 = ct{1211};
t4107 = ct{1212};
t4108 = ct{1213};
t4116 = ct{1214};
t4117 = ct{1215};
t4118 = ct{1216};
t4125 = ct{1217};
t4126 = ct{1218};
t4139 = ct{1219};
t4144 = ct{1220};
t4146 = ct{1221};
t4147 = ct{1222};
t4149 = ct{1223};
t4151 = ct{1224};
t4153 = ct{1225};
t4154 = ct{1226};
t4160 = ct{1227};
t4163 = ct{1228};
t4165 = ct{1229};
t4169 = ct{1230};
t4171 = ct{1231};
t4172 = ct{1232};
t4173 = ct{1233};
t4174 = ct{1234};
t4178 = ct{1235};
t4181 = ct{1236};
t4187 = ct{1237};
t4188 = ct{1238};
t4189 = ct{1239};
t4190 = ct{1240};
t4193 = ct{1241};
t4195 = ct{1242};
t4198 = ct{1243};
t4199 = ct{1244};
t42 = ct{1245};
t4200 = ct{1246};
t4201 = ct{1247};
t4204 = ct{1248};
t4205 = ct{1249};
t4207 = ct{1250};
t4208 = ct{1251};
t4210 = ct{1252};
t4213 = ct{1253};
t4215 = ct{1254};
t4217 = ct{1255};
t4218 = ct{1256};
t4219 = ct{1257};
t4222 = ct{1258};
t4223 = ct{1259};
t4224 = ct{1260};
t4226 = ct{1261};
t4228 = ct{1262};
t4229 = ct{1263};
t4230 = ct{1264};
t4236 = ct{1265};
t4237 = ct{1266};
t4240 = ct{1267};
t4241 = ct{1268};
t4243 = ct{1269};
t4244 = ct{1270};
t4246 = ct{1271};
t4247 = ct{1272};
t4248 = ct{1273};
t4249 = ct{1274};
t4251 = ct{1275};
t4255 = ct{1276};
t4256 = ct{1277};
t4258 = ct{1278};
t4260 = ct{1279};
t4261 = ct{1280};
t4262 = ct{1281};
t4263 = ct{1282};
t4264 = ct{1283};
t4266 = ct{1284};
t4270 = ct{1285};
t4271 = ct{1286};
t4272 = ct{1287};
t4273 = ct{1288};
t4274 = ct{1289};
t4275 = ct{1290};
t4276 = ct{1291};
t4277 = ct{1292};
t4278 = ct{1293};
t4279 = ct{1294};
t4280 = ct{1295};
t4281 = ct{1296};
t4282 = ct{1297};
t4283 = ct{1298};
t4286 = ct{1299};
t4287 = ct{1300};
t4288 = ct{1301};
t4289 = ct{1302};
t429 = ct{1303};
t4290 = ct{1304};
t4293 = ct{1305};
t4294 = ct{1306};
t4295 = ct{1307};
t4296 = ct{1308};
t4297 = ct{1309};
t4298 = ct{1310};
t4299 = ct{1311};
t43 = ct{1312};
t4300 = ct{1313};
t4301 = ct{1314};
t4303 = ct{1315};
t4304 = ct{1316};
t4305 = ct{1317};
t4306 = ct{1318};
t4307 = ct{1319};
t4308 = ct{1320};
t4310 = ct{1321};
t4311 = ct{1322};
t4312 = ct{1323};
t4313 = ct{1324};
t4314 = ct{1325};
t4318 = ct{1326};
t4319 = ct{1327};
t4322 = ct{1328};
t4323 = ct{1329};
t4324 = ct{1330};
t4325 = ct{1331};
t4326 = ct{1332};
t4328 = ct{1333};
t4330 = ct{1334};
t4331 = ct{1335};
t4332 = ct{1336};
t4333 = ct{1337};
t4334 = ct{1338};
t4335 = ct{1339};
t4337 = ct{1340};
t4339 = ct{1341};
t4340 = ct{1342};
t4341 = ct{1343};
t4342 = ct{1344};
t4343 = ct{1345};
t4344 = ct{1346};
t4346 = ct{1347};
t4347 = ct{1348};
t4348 = ct{1349};
t4352 = ct{1350};
t4353 = ct{1351};
t4354 = ct{1352};
t4356 = ct{1353};
t4358 = ct{1354};
t4362 = ct{1355};
t4365 = ct{1356};
t4366 = ct{1357};
t4371 = ct{1358};
t4372 = ct{1359};
t4373 = ct{1360};
t4374 = ct{1361};
t4375 = ct{1362};
t4376 = ct{1363};
t4377 = ct{1364};
t4378 = ct{1365};
t4379 = ct{1366};
t4380 = ct{1367};
t4386 = ct{1368};
t4387 = ct{1369};
t4388 = ct{1370};
t4389 = ct{1371};
t4394 = ct{1372};
t4396 = ct{1373};
t4401 = ct{1374};
t4402 = ct{1375};
t4403 = ct{1376};
t4404 = ct{1377};
t4405 = ct{1378};
t4406 = ct{1379};
t4410 = ct{1380};
t4413 = ct{1381};
t4414 = ct{1382};
t4415 = ct{1383};
t4416 = ct{1384};
t4417 = ct{1385};
t4420 = ct{1386};
t4422 = ct{1387};
t4423 = ct{1388};
t4424 = ct{1389};
t4425 = ct{1390};
t4426 = ct{1391};
t4455 = ct{1392};
t4456 = ct{1393};
t4457 = ct{1394};
t4458 = ct{1395};
t4459 = ct{1396};
t4460 = ct{1397};
t4462 = ct{1398};
t4464 = ct{1399};
t4465 = ct{1400};
t4466 = ct{1401};
t4467 = ct{1402};
t4468 = ct{1403};
t4470 = ct{1404};
t4471 = ct{1405};
t4472 = ct{1406};
t4476 = ct{1407};
t4477 = ct{1408};
t4478 = ct{1409};
t4479 = ct{1410};
t4480 = ct{1411};
t4481 = ct{1412};
t4482 = ct{1413};
t4485 = ct{1414};
t4486 = ct{1415};
t4487 = ct{1416};
t4488 = ct{1417};
t4489 = ct{1418};
t4491 = ct{1419};
t4492 = ct{1420};
t4493 = ct{1421};
t4494 = ct{1422};
t4495 = ct{1423};
t4496 = ct{1424};
t4497 = ct{1425};
t4498 = ct{1426};
t4499 = ct{1427};
t4500 = ct{1428};
t4501 = ct{1429};
t4502 = ct{1430};
t4503 = ct{1431};
t4504 = ct{1432};
t4507 = ct{1433};
t4508 = ct{1434};
t4509 = ct{1435};
t4510 = ct{1436};
t4511 = ct{1437};
t4513 = ct{1438};
t4515 = ct{1439};
t4516 = ct{1440};
t4517 = ct{1441};
t4518 = ct{1442};
t4519 = ct{1443};
t4520 = ct{1444};
t4521 = ct{1445};
t4522 = ct{1446};
t4523 = ct{1447};
t4524 = ct{1448};
t4525 = ct{1449};
t4528 = ct{1450};
t4529 = ct{1451};
t4530 = ct{1452};
t4531 = ct{1453};
t4532 = ct{1454};
t4533 = ct{1455};
t4534 = ct{1456};
t4535 = ct{1457};
t4536 = ct{1458};
t4537 = ct{1459};
t4538 = ct{1460};
t4540 = ct{1461};
t4541 = ct{1462};
t4542 = ct{1463};
t4543 = ct{1464};
t4544 = ct{1465};
t4545 = ct{1466};
t4546 = ct{1467};
t4548 = ct{1468};
t4549 = ct{1469};
t4550 = ct{1470};
t4551 = ct{1471};
t4554 = ct{1472};
t4559 = ct{1473};
t4561 = ct{1474};
t4563 = ct{1475};
t4570 = ct{1476};
t4571 = ct{1477};
t4572 = ct{1478};
t4575 = ct{1479};
t4576 = ct{1480};
t4578 = ct{1481};
t46 = ct{1482};
t4637 = ct{1483};
t4643 = ct{1484};
t4644 = ct{1485};
t4645 = ct{1486};
t4646 = ct{1487};
t4650 = ct{1488};
t4651 = ct{1489};
t4652 = ct{1490};
t4654 = ct{1491};
t4656 = ct{1492};
t4657 = ct{1493};
t4659 = ct{1494};
t4663 = ct{1495};
t4665 = ct{1496};
t4667 = ct{1497};
t4669 = ct{1498};
t4670 = ct{1499};
t4671 = ct{1500};
t4673 = ct{1501};
t4674 = ct{1502};
t4675 = ct{1503};
t4677 = ct{1504};
t4678 = ct{1505};
t4680 = ct{1506};
t4683 = ct{1507};
t4684 = ct{1508};
t4687 = ct{1509};
t47 = ct{1510};
t4703 = ct{1511};
t4704 = ct{1512};
t4705 = ct{1513};
t4708 = ct{1514};
t4709 = ct{1515};
t4711 = ct{1516};
t4713 = ct{1517};
t4716 = ct{1518};
t4719 = ct{1519};
t4722 = ct{1520};
t4724 = ct{1521};
t4725 = ct{1522};
t4726 = ct{1523};
t4727 = ct{1524};
t4728 = ct{1525};
t4730 = ct{1526};
t4734 = ct{1527};
t4737 = ct{1528};
t4739 = ct{1529};
t4741 = ct{1530};
t4742 = ct{1531};
t4743 = ct{1532};
t4744 = ct{1533};
t4746 = ct{1534};
t4747 = ct{1535};
t4751 = ct{1536};
t4753 = ct{1537};
t4755 = ct{1538};
t4756 = ct{1539};
t4757 = ct{1540};
t4760 = ct{1541};
t4761 = ct{1542};
t4762 = ct{1543};
t4763 = ct{1544};
t4774 = ct{1545};
t4814 = ct{1546};
t4820 = ct{1547};
t4826 = ct{1548};
t4828 = ct{1549};
t4833 = ct{1550};
t4835 = ct{1551};
t4838 = ct{1552};
t4839 = ct{1553};
t4840 = ct{1554};
t4843 = ct{1555};
t4844 = ct{1556};
t4845 = ct{1557};
t4847 = ct{1558};
t4848 = ct{1559};
t4849 = ct{1560};
t4850 = ct{1561};
t4853 = ct{1562};
t4872 = ct{1563};
t4874 = ct{1564};
t4877 = ct{1565};
t4878 = ct{1566};
t4879 = ct{1567};
t4880 = ct{1568};
t4884 = ct{1569};
t4885 = ct{1570};
t4886 = ct{1571};
t4890 = ct{1572};
t4891 = ct{1573};
t4892 = ct{1574};
t4893 = ct{1575};
t4895 = ct{1576};
t4902 = ct{1577};
t4915 = ct{1578};
t4916 = ct{1579};
t4917 = ct{1580};
t4920 = ct{1581};
t4923 = ct{1582};
t4924 = ct{1583};
t4925 = ct{1584};
t4926 = ct{1585};
t4927 = ct{1586};
t4929 = ct{1587};
t4930 = ct{1588};
t4942 = ct{1589};
t4944 = ct{1590};
t50 = ct{1591};
t5012 = ct{1592};
t5013 = ct{1593};
t5014 = ct{1594};
t5016 = ct{1595};
t5025 = ct{1596};
t5027 = ct{1597};
t5028 = ct{1598};
t5033 = ct{1599};
t5034 = ct{1600};
t5036 = ct{1601};
t5037 = ct{1602};
t5038 = ct{1603};
t5045 = ct{1604};
t5046 = ct{1605};
t5047 = ct{1606};
t5048 = ct{1607};
t5050 = ct{1608};
t5052 = ct{1609};
t5053 = ct{1610};
t5059 = ct{1611};
t5060 = ct{1612};
t5062 = ct{1613};
t5063 = ct{1614};
t5064 = ct{1615};
t5066 = ct{1616};
t5067 = ct{1617};
t5069 = ct{1618};
t5070 = ct{1619};
t5072 = ct{1620};
t5073 = ct{1621};
t5075 = ct{1622};
t5077 = ct{1623};
t5079 = ct{1624};
t5080 = ct{1625};
t5081 = ct{1626};
t5082 = ct{1627};
t5084 = ct{1628};
t5085 = ct{1629};
t5086 = ct{1630};
t5087 = ct{1631};
t5088 = ct{1632};
t5089 = ct{1633};
t5090 = ct{1634};
t5091 = ct{1635};
t5093 = ct{1636};
t5094 = ct{1637};
t5095 = ct{1638};
t5096 = ct{1639};
t5097 = ct{1640};
t5098 = ct{1641};
t5108 = ct{1642};
t5111 = ct{1643};
t5113 = ct{1644};
t5114 = ct{1645};
t5119 = ct{1646};
t5140 = ct{1647};
t5142 = ct{1648};
t5144 = ct{1649};
t5146 = ct{1650};
t5165 = ct{1651};
t5168 = ct{1652};
t5171 = ct{1653};
t5173 = ct{1654};
t5174 = ct{1655};
t5176 = ct{1656};
t5177 = ct{1657};
t5178 = ct{1658};
t5180 = ct{1659};
t5181 = ct{1660};
t5194 = ct{1661};
t5195 = ct{1662};
t5196 = ct{1663};
t5197 = ct{1664};
t5198 = ct{1665};
t5202 = ct{1666};
t5203 = ct{1667};
t5209 = ct{1668};
t5210 = ct{1669};
t5213 = ct{1670};
t5214 = ct{1671};
t5215 = ct{1672};
t5217 = ct{1673};
t5218 = ct{1674};
t5219 = ct{1675};
t5240 = ct{1676};
t5246 = ct{1677};
t5247 = ct{1678};
t5251 = ct{1679};
t5254 = ct{1680};
t5255 = ct{1681};
t5256 = ct{1682};
t5257 = ct{1683};
t5260 = ct{1684};
t5261 = ct{1685};
t5262 = ct{1686};
t5274 = ct{1687};
t5276 = ct{1688};
t5277 = ct{1689};
t5278 = ct{1690};
t5279 = ct{1691};
t5280 = ct{1692};
t5281 = ct{1693};
t5283 = ct{1694};
t5284 = ct{1695};
t5285 = ct{1696};
t5286 = ct{1697};
t5287 = ct{1698};
t5288 = ct{1699};
t5289 = ct{1700};
t5290 = ct{1701};
t5291 = ct{1702};
t5292 = ct{1703};
t5293 = ct{1704};
t5294 = ct{1705};
t5295 = ct{1706};
t5296 = ct{1707};
t5297 = ct{1708};
t5298 = ct{1709};
t5300 = ct{1710};
t5301 = ct{1711};
t5302 = ct{1712};
t5303 = ct{1713};
t5304 = ct{1714};
t5305 = ct{1715};
t5308 = ct{1716};
t5309 = ct{1717};
t5310 = ct{1718};
t5312 = ct{1719};
t5315 = ct{1720};
t5320 = ct{1721};
t5321 = ct{1722};
t5350 = ct{1723};
t5356 = ct{1724};
t5357 = ct{1725};
t5361 = ct{1726};
t5363 = ct{1727};
t5370 = ct{1728};
t5372 = ct{1729};
t5381 = ct{1730};
t5391 = ct{1731};
t5392 = ct{1732};
t5393 = ct{1733};
t5395 = ct{1734};
t5399 = ct{1735};
t5400 = ct{1736};
t5401 = ct{1737};
t5402 = ct{1738};
t5403 = ct{1739};
t5404 = ct{1740};
t5415 = ct{1741};
t5416 = ct{1742};
t5433 = ct{1743};
t5434 = ct{1744};
t5436 = ct{1745};
t5437 = ct{1746};
t5438 = ct{1747};
t5439 = ct{1748};
t5444 = ct{1749};
t5445 = ct{1750};
t5446 = ct{1751};
t5448 = ct{1752};
t5452 = ct{1753};
t5456 = ct{1754};
t5457 = ct{1755};
t5458 = ct{1756};
t5459 = ct{1757};
t5460 = ct{1758};
t5464 = ct{1759};
t5481 = ct{1760};
t5485 = ct{1761};
t5487 = ct{1762};
t5488 = ct{1763};
t5494 = ct{1764};
t5495 = ct{1765};
t5499 = ct{1766};
t5513 = ct{1767};
t5516 = ct{1768};
t5517 = ct{1769};
t5520 = ct{1770};
t5535 = ct{1771};
t5536 = ct{1772};
t5537 = ct{1773};
t5538 = ct{1774};
t5539 = ct{1775};
t5540 = ct{1776};
t5541 = ct{1777};
t5542 = ct{1778};
t5543 = ct{1779};
t5544 = ct{1780};
t5545 = ct{1781};
t5548 = ct{1782};
t5549 = ct{1783};
t5550 = ct{1784};
t5555 = ct{1785};
t5556 = ct{1786};
t5560 = ct{1787};
t5561 = ct{1788};
t5565 = ct{1789};
t5566 = ct{1790};
t5568 = ct{1791};
t5569 = ct{1792};
t5570 = ct{1793};
t5575 = ct{1794};
t5576 = ct{1795};
t5586 = ct{1796};
t5590 = ct{1797};
t56 = ct{1798};
t5604 = ct{1799};
t5605 = ct{1800};
t5607 = ct{1801};
t5608 = ct{1802};
t5609 = ct{1803};
t5611 = ct{1804};
t5612 = ct{1805};
t5660 = ct{1806};
t5678 = ct{1807};
t5684 = ct{1808};
t5730 = ct{1809};
t5731 = ct{1810};
t5734 = ct{1811};
t5735 = ct{1812};
t5738 = ct{1813};
t5739 = ct{1814};
t5741 = ct{1815};
t5742 = ct{1816};
t5758 = ct{1817};
t5759 = ct{1818};
t5760 = ct{1819};
t5761 = ct{1820};
t5779 = ct{1821};
t5782 = ct{1822};
t5783 = ct{1823};
t58 = ct{1824};
t5803 = ct{1825};
t5849 = ct{1826};
t5896 = ct{1827};
t59 = ct{1828};
t5901 = ct{1829};
t5902 = ct{1830};
t5903 = ct{1831};
t5916 = ct{1832};
t5917 = ct{1833};
t5938 = ct{1834};
t5941 = ct{1835};
t5954 = ct{1836};
t5955 = ct{1837};
t5990 = ct{1838};
t60 = ct{1839};
t6002 = ct{1840};
t6011 = ct{1841};
t6013 = ct{1842};
t6014 = ct{1843};
t6050 = ct{1844};
t6062 = ct{1845};
t6074 = ct{1846};
t6143 = ct{1847};
t6255 = ct{1848};
t6256 = ct{1849};
t6257 = ct{1850};
t6271 = ct{1851};
t628 = ct{1852};
t635 = ct{1853};
t636 = ct{1854};
t638 = ct{1855};
t6394 = ct{1856};
t640 = ct{1857};
t641 = ct{1858};
t642 = ct{1859};
t643 = ct{1860};
t6442 = ct{1861};
t649 = ct{1862};
t654 = ct{1863};
t655 = ct{1864};
t656 = ct{1865};
t6564 = ct{1866};
t6565 = ct{1867};
t657 = ct{1868};
t6574 = ct{1869};
t6588 = ct{1870};
t659 = ct{1871};
t660 = ct{1872};
t6622 = ct{1873};
t6623 = ct{1874};
t663 = ct{1875};
t664 = ct{1876};
t665 = ct{1877};
t667 = ct{1878};
t668 = ct{1879};
t669 = ct{1880};
t67 = ct{1881};
t670 = ct{1882};
t672 = ct{1883};
t673 = ct{1884};
t674 = ct{1885};
t6745 = ct{1886};
t675 = ct{1887};
t6751 = ct{1888};
t676 = ct{1889};
t677 = ct{1890};
t678 = ct{1891};
t679 = ct{1892};
t68 = ct{1893};
t681 = ct{1894};
t682 = ct{1895};
t684 = ct{1896};
t685 = ct{1897};
t686 = ct{1898};
t687 = ct{1899};
t689 = ct{1900};
t691 = ct{1901};
t6919 = ct{1902};
t692 = ct{1903};
t6920 = ct{1904};
t693 = ct{1905};
t694 = ct{1906};
t6987 = ct{1907};
t70 = ct{1908};
t7005 = ct{1909};
t702 = ct{1910};
t707 = ct{1911};
t708 = ct{1912};
t71 = ct{1913};
t710 = ct{1914};
t7117 = ct{1915};
t7141 = ct{1916};
t715 = ct{1917};
t7150 = ct{1918};
t716 = ct{1919};
t717 = ct{1920};
t718 = ct{1921};
t721 = ct{1922};
t722 = ct{1923};
t724 = ct{1924};
t725 = ct{1925};
t73 = ct{1926};
t7304 = ct{1927};
t736 = ct{1928};
t738 = ct{1929};
t740 = ct{1930};
t741 = ct{1931};
t749 = ct{1932};
t756 = ct{1933};
t76 = ct{1934};
t762 = ct{1935};
t768 = ct{1936};
t777 = ct{1937};
t792 = ct{1938};
t793 = ct{1939};
t8 = ct{1940};
t801 = ct{1941};
t802 = ct{1942};
t808 = ct{1943};
t813 = ct{1944};
t819 = ct{1945};
t821 = ct{1946};
t850 = ct{1947};
t855 = ct{1948};
t874 = ct{1949};
t878 = ct{1950};
t89 = ct{1951};
t9 = ct{1952};
t90 = ct{1953};
t91 = ct{1954};
t92 = ct{1955};
t941 = ct{1956};
t944 = ct{1957};
t948 = ct{1958};
t951 = ct{1959};
t97 = ct{1960};
t4581 = t3976.*(t1896-t3239).*(-1.02e-6);
t4583 = t3543.*t3976.*4.0e-8;
t4584 = t3976.*(t1896-t3239).*1.02e-6;
t4587 = t3976.*(t1896-t3239).*(-2.4e-7);
t4588 = t3976.*(t1896-t3239).*(-4.0e-8);
t4593 = t3976.*(t1896-t3239).*2.4e-7;
t4595 = t3976.*(t1896-t3239).*4.0e-8;
t4648 = -t4645;
t4658 = t3711.*t4019;
t4660 = -t4659;
t4672 = -t4671;
t4676 = -t4675;
t4681 = t3814.*t4019;
t4682 = t3815.*t4019;
t4691 = t4262.*(t1896-t3239).*(-9.3e-7);
t4692 = t4262.*(t1896-t3239).*(-9.0e-8);
t4693 = t4264.*(t1896-t3239).*(-1.02e-6);
t4694 = t4264.*(t1896-t3239).*1.02e-6;
t4695 = t4264.*(t1896-t3239).*(-9.0e-8);
t4696 = t4264.*(t1896-t3239).*9.0e-8;
t4731 = t3893.*t4019;
t4764 = t3976.*(t2694-t2701+t3036-t3043).*(-1.0e-8);
t4776 = t3976.*(t2694-t2701+t3036-t3043).*(-5.7e-7);
t4777 = t3976.*(t2694-t2701+t3036-t3043).*(-1.02e-6);
t4778 = t3976.*(t2694-t2701+t3036-t3043).*(-2.4e-7);
t4779 = t3976.*(t2694-t2701+t3036-t3043).*(-4.0e-8);
t4782 = t3976.*(t1959-t3313+t38.*t1022.*(t855-t878).*2.196325630278387e-1).*(-5.7e-7);
t4786 = t3976.*(t1959-t3313+t38.*t1022.*(t855-t878).*2.196325630278387e-1).*5.7e-7;
t4790 = t3976.*(t1959-t3313+t38.*t1022.*(t855-t878).*2.196325630278387e-1).*(-4.0e-8);
t4846 = -t4844;
t4863 = t4839.*1.838876e-2;
t4867 = t4840.*9.99471e-3;
t4875 = t3976.*(t3242-t3554).*(-1.02e-6);
t4896 = t22.*t4880;
t4897 = t28.*t4880;
t4928 = -t4927;
t4933 = t3976.*(t1005+t20.*(t1941-t3315+t39.*t1022.*(t855-t878).*2.196325630278387e-1)).*(-5.7e-7);
t4937 = t3976.*(t1005+t20.*(t1941-t3315+t39.*t1022.*(t855-t878).*2.196325630278387e-1)).*(-4.0e-8);
t4939 = t3278+t3296+t3594+t3595;
t4952 = t4262.*(t2694-t2701+t3036-t3043).*(-9.3e-7);
t4953 = t4262.*(t2694-t2701+t3036-t3043).*(-9.0e-8);
t4954 = t4264.*(t2694-t2701+t3036-t3043).*(-1.02e-6);
t4955 = t4264.*(t2694-t2701+t3036-t3043).*1.02e-6;
t4956 = t4264.*(t2694-t2701+t3036-t3043).*(-9.0e-8);
t4958 = t4264.*(t2694-t2701+t3036-t3043).*9.0e-8;
t5000 = t4262.*(t3242-t3554).*(-9.3e-7);
t5001 = t4262.*(t3242-t3554).*9.3e-7;
t5002 = t4262.*(t3242-t3554).*(-9.0e-8);
t5003 = t4264.*(t3242-t3554).*(-1.02e-6);
t5004 = t4262.*(t3242-t3554).*9.0e-8;
t5005 = t4264.*(t3242-t3554).*(-9.0e-8);
t5018 = -t4289.*(-t2804+t2838+t3109+t17.*(t1456-t2355).*9.3e-7);
t5019 = t4289.*(-t2804+t2838+t3109+t17.*(t1456-t2355).*9.3e-7);
t5020 = -t4290.*(t2813-t2835+t12.*(t1456-t2355).*1.02e-6+t17.*(t1456-t2355).*9.0e-8);
t5024 = t3398+t3411+t3715+t3718;
t5035 = -t5034;
t5039 = -t5038;
t5041 = t3065+t4062+t4070;
t5042 = t3074+t4077+t4093;
t5043 = t3076+t4079+t4095;
t5049 = -t5048;
t5051 = -t5050;
t5061 = -t5060;
t5071 = -t5067;
t5074 = -t5069;
t5076 = -t5073;
t5102 = t2388.*(-t3064+t4065+t3236.*(t1861-t3221).*9.840000000000001e-6).*(-1.0./2.0);
t5126 = -t5119;
t5143 = t641+t663+t664+t678+t1581+t1595+t1596+t1601+t2296+t2324+t2681+t3031+t3289+t3317;
t5199 = -t5198;
t5200 = t58+t59+t5142;
t5201 = t429+t5142;
t5205 = t410+t649+t670+t686+t687+t1577+t1578+t1586+t1600+t2303+t2339+t2689+t3030+t3299+t3312;
t5234 = -t3055.*(-t3080+t4100+t11.*t3236.*(t1861-t3221).*1.02e-6);
t5239 = t3055.*(-t3080+t4100+t11.*t3236.*(t1861-t3221).*1.02e-6).*(-1.0./2.0);
t5241 = t3815.*t4880;
t5248 = t3649.*t3934.*t4323.*1.444822e-2;
t5258 = (t3638.*t3910.*t4376)./2.0;
t5263 = -t3543.*(-t3064+t4065+t3236.*(t1861-t3221).*9.840000000000001e-6);
t5267 = -t3550.*(-t3064+t4065+t3236.*(t1861-t3221).*9.840000000000001e-6);
t5306 = t188.*t5260.*4.297799892626299e-1;
t5307 = t1190+t1214+t1219+t1220+t2145+t2146+t2153+t2169+t2742+t2790+t2947+t3078+t3407+t3425;
t5318 = t4126+t4839;
t5319 = t4139+t4840;
t5328 = t3976.*t4920.*5.7e-7;
t5332 = t3976.*t4920.*4.0e-8;
t5343 = (t2307.*t5260)./2.0;
t5344 = (t2338.*t5260)./2.0;
t5345 = t4507+t4509;
t5346 = t4503+t4516;
t5349 = t3255+t3572+t4116+t4117;
t5352 = t4511+t4536;
t5353 = t4513+t4538;
t5354 = t4535+t4543;
t5358 = t322+t330+t5305;
t5359 = t352+t369+t5305;
t5362 = t341+t370+t1196+t1212+t1237+t1238+t2139+t2140+t2159+t2165+t2754+t2814+t2953+t3072+t3415+t3423;
t5371 = t3366+t3670+t4173+t4174;
t5378 = t50.*t202.*(t3251-t3572+t22.*(t3242-t3554).*1.838876e-2+t28.*(t3242-t3554).*9.99471e-3).*(-6.935255936130809e-19);
t5410 = (t3242-t3554).*(-t3080+t4100+t11.*t3236.*(t1861-t3221).*1.02e-6);
t5442 = t3236.*(t4125-t4840).*(-9.3e-7);
t5443 = t3236.*(t4125-t4840).*(-9.0e-8);
t5449 = (t3915.*t5140)./2.0;
t5504 = (t1896-t3239).*(t4125-t4840).*9.3e-7;
t5510 = (t1896-t3239).*(t4125-t4840).*9.0e-8;
t5567 = -t5566;
t5577 = t3910.*t4172.*(t3421-t3731+t3737+t20.*t50.*t202.*(t46-t47).*8.687615694748404e-39).*(-1.0./2.0);
t5578 = (t3910.*t4172.*(t3421-t3731+t3737+t20.*t50.*t202.*(t46-t47).*8.687615694748404e-39))./2.0;
t5591 = t4376.*(-t56+t60+t649+t670+t686+t687+t1577+t1578+t1586+t1600+t2303+t2339+t2689+t3030+t3299+t3312).*(-1.0./2.0);
t5592 = (t4376.*(-t56+t60+t649+t670+t686+t687+t1577+t1578+t1586+t1600+t2303+t2339+t2689+t3030+t3299+t3312))./2.0;
t5595 = t3761+t3852+t3853+t3871+t3928;
t5599 = (t4125-t4840).*(t2694-t2701+t3036-t3043).*9.3e-7;
t5602 = (t4125-t4840).*(t2694-t2701+t3036-t3043).*9.0e-8;
t5620 = (t3242-t3554).*(t4125-t4840).*9.3e-7;
t5624 = t3369.*t3934.*(-t56+t60+t649+t670+t686+t687+t1577+t1578+t1586+t1600+t2303+t2339+t2689+t3030+t3299+t3312).*(-1.444822e-2);
t5627 = (t3242-t3554).*(t4125-t4840).*9.0e-8;
t5653 = t3649.*t3934.*t5142.*1.444822e-2;
t5658 = t3649.*(t2694-t2701+t3036-t3043).*(t649+t670+t686+t687+t1577+t1578+t1586+t1600+t2303+t2339+t2689+t3030+t3299+t3312).*1.444822e-2;
t5662 = -t5350.*(-t2804+t2838+t3109+t17.*(t1456-t2355).*9.3e-7);
t5677 = t3649.*(t2694-t2701+t3036-t3043).*(-t56+t60+t649+t670+t686+t687+t1577+t1578+t1586+t1600+t2303+t2339+t2689+t3030+t3299+t3312).*1.444822e-2;
t5698 = t2515+t3077+t3881+t3883+t4084+t4089;
t5699 = t2529+t3075+t3882+t3884+t4083+t4088;
t5704 = t50.*t189.*(t3524.*1.838876e-2-t3591+t3592+t4322+t16.*(t1861-t3221).*(3.0./5.0e+2)+t16.*t17.*(t1861-t3221).*9.99471e-3).*(-9.543032792050485e-17);
t5705 = t50.*t189.*(t3524.*1.838876e-2-t3591+t3592+t4322+t16.*(t1861-t3221).*(3.0./5.0e+2)+t16.*t17.*(t1861-t3221).*9.99471e-3).*9.543032792050485e-17;
t5719 = -t2297.*(t2292+t3290+t3524.*1.838876e-2-t3591+t3592+t3611+t16.*(t1861-t3221).*3.131399999999998e-4+t16.*t17.*(t1861-t3221).*9.99471e-3);
t5721 = t4323.*(-t321+t332+t1196+t1212+t1237+t1238+t2139+t2140+t2159+t2165+t2754+t2814+t2953+t3072+t3415+t3423).*(-1.0./2.0);
t5722 = (t4323.*(-t321+t332+t1196+t1212+t1237+t1238+t2139+t2140+t2159+t2165+t2754+t2814+t2953+t3072+t3415+t3423))./2.0;
t5737 = t2363.*(t3328+t3344+t3642-t3658+t22.*(t3242-t3554).*1.838876e-2+t28.*(t3242-t3554).*9.99471e-3).*(-7.26735e-3);
t5743 = t50.*t202.*(t2342-t2423+t3331+t3356+t3582.*1.838876e-2-t3639+t3640+t27.*(t1896-t3239).*(3.0./5.0e+2)+t27.*t28.*(t1896-t3239).*9.99471e-3).*(-6.935255936130809e-19);
t5744 = t50.*t202.*(t2342-t2423+t3331+t3356+t3582.*1.838876e-2-t3639+t3640+t27.*(t1896-t3239).*(3.0./5.0e+2)+t27.*t28.*(t1896-t3239).*9.99471e-3).*6.935255936130809e-19;
et68 = t2363.*(t2368+t3340+t3582.*1.838876e-2-t3639+t3640+t21.*(t1896-t3239).*1.247162e-2+t27.*(t1896-t3239).*3.131399999999998e-4+t27.*t28.*(t1896-t3239).*9.99471e-3);
et69 = -7.26735e-3;
t5757 = et68.*et69;
t5768 = t3322.*t3910.*(-t321+t332+t1196+t1212+t1237+t1238+t2139+t2140+t2159+t2165+t2754+t2814+t2953+t3072+t3415+t3423).*(-1.0./2.0);
t5775 = (t3638.*t3910.*t5305)./2.0;
t5777 = (t3638.*(t2674-t2676+t3022-t3027).*(t1196+t1212+t1237+t1238+t2139+t2140+t2159+t2165+t2754+t2814+t2953+t3072+t3415+t3423))./2.0;
t5781 = (t3910.*t5485)./2.0;
t5784 = (t4879.*t5140)./2.0;
t5788 = (t3638.*(t2674-t2676+t3022-t3027).*(-t321+t332+t1196+t1212+t1237+t1238+t2139+t2140+t2159+t2165+t2754+t2814+t2953+t3072+t3415+t3423))./2.0;
t5813 = t50.*t189.*t5803.*4.771516396025243e-17;
t5818 = t3585+t3812+t3813+t3887+t3894+t4199;
t5825 = (t2297.*t5803)./2.0;
t5852 = (t1477-t2502).*(t3081-t3086+t4086-t4099+t4105+t11.*t3236.*(t1861-t3221).*4.0e-8);
t5891 = (t2694-t2701+t3036-t3043).*(t3524.*1.838876e-2-t3591+t3592+t16.*(t1861-t3221).*(3.0./5.0e+2)+t16.*t17.*(t1861-t3221).*9.99471e-3).*(t1513+t1879+t2598+t2820+t2834+t3117+t3118).*(-3.633675e-3);
t5892 = (t2694-t2701+t3036-t3043).*(t3524.*1.838876e-2-t3591+t3592+t16.*(t1861-t3221).*(3.0./5.0e+2)+t16.*t17.*(t1861-t3221).*9.99471e-3).*(t1513+t1879+t2598+t2820+t2834+t3117+t3118).*3.633675e-3;
t5895 = t3649.*t5560.*(t2694-t2701+t3036-t3043).*(-1.444822e-2);
et70 = t3582.*1.33637554986e-4+t3716-t3717+t27.*(t1896-t3239).*4.36041e-5;
et71 = t27.*t28.*(t1896-t3239).*7.26350557185e-5;
t5908 = (et70+et71).*(t2674-t2676+t3022-t3027).*(t1488+t1874+t2519+t2740+t2747+t3096+t3097).*(-1.0./2.0);
et72 = t3582.*1.33637554986e-4+t3716-t3717+t27.*(t1896-t3239).*4.36041e-5;
et73 = t27.*t28.*(t1896-t3239).*7.26350557185e-5;
t5909 = ((et72+et73).*(t2674-t2676+t3022-t3027).*(t1488+t1874+t2519+t2740+t2747+t3096+t3097))./2.0;
t5921 = t5305.*(-t56+t60+t649+t670+t686+t687+t1577+t1578+t1586+t1600+t2303+t2339+t2689+t3030+t3299+t3312).*(-1.0./2.0);
t5922 = (t5305.*(-t56+t60+t649+t670+t686+t687+t1577+t1578+t1586+t1600+t2303+t2339+t2689+t3030+t3299+t3312))./2.0;
t5924 = (t3359-t3670+t22.*(t3242-t3554).*1.33637554986e-4+t28.*(t3242-t3554).*7.26350557185e-5).*(t2674-t2676+t3022-t3027).*(t1488+t1874+t2519+t2740+t2747+t3096+t3097).*(-1.0./2.0);
t5925 = ((t3359-t3670+t22.*(t3242-t3554).*1.33637554986e-4+t28.*(t3242-t3554).*7.26350557185e-5).*(t2674-t2676+t3022-t3027).*(t1488+t1874+t2519+t2740+t2747+t3096+t3097))./2.0;
t5928 = t50.*t189.*t5903.*4.771516396025243e-17;
t5932 = t5142.*(-t321+t332+t1196+t1212+t1237+t1238+t2139+t2140+t2159+t2165+t2754+t2814+t2953+t3072+t3415+t3423).*(-1.0./2.0);
t5933 = (t5142.*(-t321+t332+t1196+t1212+t1237+t1238+t2139+t2140+t2159+t2165+t2754+t2814+t2953+t3072+t3415+t3423))./2.0;
t5944 = -t5941;
t5966 = (t2297.*t5903)./2.0;
t5971 = -t4019.*(t3081-t3086+t4086-t4099+t4105+t11.*t3236.*(t1861-t3221).*4.0e-8);
t6004 = t4386+t4387+t4521+t4525;
t6005 = t4388+t4389+t4519+t4524;
t6048 = t2162+t2775+t2803+t2807+t2808+t4034+t4036+t4042+t4247+t4251;
t6051 = t3762+t3763+t4266+t4271+t4365+t4366;
t6075 = t3464+t3475+t4335+t4340+t4410+t4414;
t6078 = (t1477-t2502).*(t4533+t4542-t4546-t4550);
t6089 = t3836+t3854+t3899+t4328+t4348+t4424;
t6104 = t3016+t3068+t4471+t4472+t4508+t4518;
et74 = t3015-t3068+t4470-t4518+t3500.*(t1959-t3313+t38.*t1022.*(t855-t878).*2.196325630278387e-1).*9.840000000000001e-6;
et75 = t3237.*((t237.*(t42-t43))./9.007199254740992e+15+t15.*(-t1881+t3121+t3276)).*9.840000000000001e-6;
t6123 = -t2388.*(et74+et75);
et76 = t3015-t3068+t4470-t4518+t3500.*(t1959-t3313+t38.*t1022.*(t855-t878).*2.196325630278387e-1).*9.840000000000001e-6;
et77 = t3237.*((t237.*(t42-t43))./9.007199254740992e+15+t15.*(-t1881+t3121+t3276)).*9.840000000000001e-6;
t6124 = t2388.*(et76+et77).*(-1.0./2.0);
et78 = t3015-t3068+t4470-t4518+t3500.*(t1959-t3313+t38.*t1022.*(t855-t878).*2.196325630278387e-1).*9.840000000000001e-6;
et79 = t3237.*((t237.*(t42-t43))./9.007199254740992e+15+t15.*(-t1881+t3121+t3276)).*9.840000000000001e-6;
t6125 = (t2388.*(et78+et79))./2.0;
et80 = -t2748-t2749+t2773+t2781-t2788+t3211+t3471+t4032-t4047+t262.*(t46-t47).*2.075672598245148e-23;
et81 = t264.*(t46-t47).*1.875105520197095e-20;
t6132 = ((et80+et81).*(-t56+t60+t649+t670+t686+t687+t1577+t1578+t1586+t1600+t2303+t2339+t2689+t3030+t3299+t3312))./2.0;
t6165 = t5561.*(-t321+t332+t1196+t1212+t1237+t1238+t2139+t2140+t2159+t2165+t2754+t2814+t2953+t3072+t3415+t3423).*(-1.0./2.0);
t6166 = (t5561.*(-t321+t332+t1196+t1212+t1237+t1238+t2139+t2140+t2159+t2165+t2754+t2814+t2953+t3072+t3415+t3423))./2.0;
t6211 = -t4019.*(t4533+t4542-t4546-t4550);
et82 = t3015-t3068+t4470-t4518+t3500.*(t1959-t3313+t38.*t1022.*(t855-t878).*2.196325630278387e-1).*9.840000000000001e-6;
et83 = t3237.*((t237.*(t42-t43))./9.007199254740992e+15+t15.*(-t1881+t3121+t3276)).*9.840000000000001e-6;
t6221 = -t3543.*(et82+et83);
et84 = t3015-t3068+t4470-t4518+t3500.*(t1959-t3313+t38.*t1022.*(t855-t878).*2.196325630278387e-1).*9.840000000000001e-6;
et85 = t3237.*((t237.*(t42-t43))./9.007199254740992e+15+t15.*(-t1881+t3121+t3276)).*9.840000000000001e-6;
t6222 = -t3550.*(et84+et85);
et86 = t707+t708-t721-t722-t749+t762+t768-t777-t792-t793-t801-t802-t808+t813-t819+t821-t1629+t1637-t1640-t1641-t1659-t1661+t1666+t1667+t1683+t1692+t1705-t1712+t1758+t1759+t1775+t1776+t1973+t1993+t1994+t2023+t2053+t2060-t2089-t2090+t2098+t2099-t8.*t9.*t15.*t50.*t189.*3.670836568391568e-22;
et87 = t10.*t13.*t14.*t50.*t189.*(-3.279367663374749e-19)-t8.*t9.*t11.*t15.*t50.*t189.*7.075931802640439e-19;
et88 = t8.*t11.*t14.*t15.*t50.*t189.*(-1.190170786299927e-18)-t9.*t11.*t13.*t15.*t50.*t189.*1.190170786299927e-18;
et89 = t13.*t14.*t15.*t16.*t50.*t189.*(-3.226512155691387e-19);
t6396 = ((t3421-t3731+t3737+t20.*t50.*t202.*(t46-t47).*8.687615694748404e-39).*(et86+et87+et88+et89))./2.0;
t6398 = t4215.*t6002.*(t2694-t2701+t3036-t3043).*(-5.43845e-3);
t6399 = t4215.*t6002.*(t2694-t2701+t3036-t3043).*5.43845e-3;
t6448 = t3216.*(-t4236+t4330+t4645+t3213.*(t1896-t3239)+t4019.*(t2801-t2850)+t21.*t3893.*(t1896-t3239)).*(-1.0./2.0);
t6482 = ((t1861-t3221).*(-t4236+t4330+t4645+t3213.*(t1896-t3239)+t4019.*(t2801-t2850)+t21.*t3893.*(t1896-t3239)))./2.0;
t6523 = ((t2674-t2676+t3022-t3027).*(-t4236+t4330+t4645+t3213.*(t1896-t3239)+t4019.*(t2801-t2850)+t21.*t3893.*(t1896-t3239)))./2.0;
t6589 = t4877+t4878+t5209+t5210;
t6651 = t2735+t2823+t2927+t2941+t3006+t3010+t4004+t4228+t4255+t4256+t4942+t4944;
t6966 = t3934.*t6588.*(t1513+t1879+t2598+t2820+t2834+t3117+t3118).*(-3.633675e-3);
t6967 = t3934.*t6588.*(t1513+t1879+t2598+t2820+t2834+t3117+t3118).*3.633675e-3;
t7088 = t2963+t2964+t3019+t3083+t4377+t4379+t4396+t4402+t4478+t4481+t4530+t4531;
t7089 = t2969+t2970+t3018+t3082+t4378+t4380+t4394+t4401+t4477+t4480+t4528+t4540;
t7138 = t50.*t189.*t7117.*9.543032792050485e-17;
t7148 = (t6002.*t6255)./2.0;
t7152 = t1598+t1703+t2358+t2402+t2413+t2422+t2433+t2434+t2539+t2664+t2985+t2986+t3179+t3393+t3950+t3989+t4005+t4181+t4222+t4223+t4916+t4917;
t7160 = t2297.*t7141;
t7172 = t1612+t2358+t2447+t2450+t2459+t2460+t2508+t2539+t2664+t2985+t2986+t3990+t3994+t4000+t4217+t4222+t4223+t4226+t4916+t4917;
t7317 = t4747+t4755+t4885+t4891+t5085+t5094+t5214+t5218;
t7318 = t4753+t4756+t4884+t4890+t5086+t5095+t5213+t5217;
et90 = t4751-t5086+t5093-t5213+t4920.*(t1861-t3221).*3.24e-6+t3934.*(t951+t10.*(-t1881+t3121+t3276)).*3.24e-6+t4118.*(t2694-t2701+t3036-t3043).*3.24e-6;
et91 = t3934.*(-t1901+t3122+t3277).*3.11e-6;
t7319 = t50.*t202.*(et90+et91).*(-4.771516396025243e-17);
et92 = t4751-t5086+t5093-t5213+t4920.*(t1861-t3221).*3.24e-6+t3934.*(t951+t10.*(-t1881+t3121+t3276)).*3.24e-6+t4118.*(t2694-t2701+t3036-t3043).*3.24e-6;
et93 = t3934.*(-t1901+t3122+t3277).*3.11e-6;
t7320 = t50.*t202.*(et92+et93).*4.771516396025243e-17;
et94 = t4746-t5085+t5091-t5214+t4920.*(t1861-t3221).*7.83e-6+t3934.*(t951+t10.*(-t1881+t3121+t3276)).*7.83e-6+t4118.*(t2694-t2701+t3036-t3043).*7.83e-6;
et95 = t3934.*(-t1901+t3122+t3277).*3.24e-6;
t7321 = t2363.*(et94+et95).*(-1.0./2.0);
et96 = t4751-t5086+t5093-t5213+t4920.*(t1861-t3221).*3.24e-6+t3934.*(t951+t10.*(-t1881+t3121+t3276)).*3.24e-6+t4118.*(t2694-t2701+t3036-t3043).*3.24e-6;
et97 = t3934.*(-t1901+t3122+t3277).*3.11e-6;
t7330 = -t3236.*(et96+et97);
et98 = t4751-t5086+t5093-t5213+t4920.*(t1861-t3221).*3.24e-6+t3934.*(t951+t10.*(-t1881+t3121+t3276)).*3.24e-6+t4118.*(t2694-t2701+t3036-t3043).*3.24e-6;
et99 = t3934.*(-t1901+t3122+t3277).*3.11e-6;
t7331 = -t3237.*(et98+et99);
et100 = t4751-t5086+t5093-t5213+t4920.*(t1861-t3221).*3.24e-6+t3934.*(t951+t10.*(-t1881+t3121+t3276)).*3.24e-6+t4118.*(t2694-t2701+t3036-t3043).*3.24e-6;
et101 = t3934.*(-t1901+t3122+t3277).*3.11e-6;
t7332 = t3236.*(et100+et101);
et102 = t4746-t5085+t5091-t5214+t4920.*(t1861-t3221).*7.83e-6+t3934.*(t951+t10.*(-t1881+t3121+t3276)).*7.83e-6+t4118.*(t2694-t2701+t3036-t3043).*7.83e-6;
et103 = t3934.*(-t1901+t3122+t3277).*3.24e-6;
t7333 = (et102+et103).*(t1896-t3239);
et104 = t4746-t5085+t5091-t5214+t4920.*(t1861-t3221).*7.83e-6+t3934.*(t951+t10.*(-t1881+t3121+t3276)).*7.83e-6+t4118.*(t2694-t2701+t3036-t3043).*7.83e-6;
et105 = t3934.*(-t1901+t3122+t3277).*3.24e-6;
t7334 = -t3547.*(et104+et105);
t3528 = -t3520;
t3537 = -t3535;
t3584 = -t3575;
t3589 = -t3587;
t3617 = -t3606;
t3621 = -t3610;
t3630 = t3521.*9.99471e-3;
t3631 = t3520.*1.838876e-2;
t3632 = -t3622;
t3633 = -t3625;
t3635 = -t3629;
t3660 = -t3652;
t3662 = -t3656;
t3667 = -t3663;
t3672 = -t3665;
t3674 = t3576.*9.99471e-3;
t3675 = t3575.*1.838876e-2;
t3684 = -t3682;
t3741 = -t3733;
t3749 = -t3742;
t3751 = -t3746;
t3753 = t3576.*7.26350557185e-5;
t3754 = t3575.*1.33637554986e-4;
t3997 = -t3985;
t4001 = t3227+t3526;
t4031 = t3245+t3573;
t4045 = t3984.*9.99471e-3;
t4046 = t3985.*9.99471e-3;
t4048 = t3984.*1.838876e-2;
t4049 = t3985.*1.838876e-2;
t4059 = t17.*t3980.*9.99471e-3;
t4060 = t12.*t3980.*1.838876e-2;
t4063 = t17.*t3991.*9.99471e-3;
t4064 = t12.*t3991.*1.838876e-2;
t4109 = t4025.*1.838876e-2;
t4110 = t4024.*9.99471e-3;
t4111 = t4025.*9.99471e-3;
t4112 = t4024.*1.838876e-2;
t4121 = t28.*t4026.*9.99471e-3;
t4122 = t22.*t4026.*1.838876e-2;
t4156 = t4024.*1.33637554986e-4;
t4157 = t4025.*1.33637554986e-4;
t4158 = t4024.*7.26350557185e-5;
t4159 = t4025.*7.26350557185e-5;
t4179 = t22.*t4026.*1.33637554986e-4;
t4180 = t28.*t4026.*7.26350557185e-5;
t4265 = t3516+t3521;
t4291 = t3565+t3576;
t4320 = t11.*t2297.*t4026.*1.02e-6;
t4345 = t3063.*t4026;
t4355 = -t4353;
t4359 = t3133.*t4026;
t4361 = -t4026.*(t1953-t2828);
t4407 = (t3236.*t3980)./1.0e+8;
t4409 = (t3237.*t3991)./1.0e+8;
t4427 = t3236.*t3980.*5.7e-7;
t4428 = t3236.*t3980.*1.02e-6;
t4429 = -t4425;
t4430 = -t4426;
t4431 = t3236.*t3980.*2.4e-7;
t4432 = t3236.*t3980.*4.0e-8;
t4434 = t17.*t3236.*t3980.*9.3e-7;
t4435 = t3237.*t3991.*5.7e-7;
t4436 = t3237.*t3991.*1.02e-6;
t4438 = t12.*t3236.*t3980.*9.0e-8;
t4439 = t17.*t3236.*t3980.*9.0e-8;
t4440 = t3237.*t3991.*2.4e-7;
t4441 = t3237.*t3991.*4.0e-8;
t4443 = t17.*t3237.*t3991.*9.3e-7;
t4448 = t12.*t3237.*t3991.*9.0e-8;
t4449 = t17.*t3237.*t3991.*9.0e-8;
t4461 = -t4460;
t4553 = t3509+t3984;
t4562 = (t3543.*t3980)./1.0e+8;
t4564 = t3980.*(t1896-t3239).*(-1.0e-8);
t4565 = (t3547.*t3991)./1.0e+8;
t4567 = (t3550.*t3991)./1.0e+8;
t4573 = t3560+t4024;
t4574 = -t4572;
t4577 = t3566+t4025;
t4579 = -t4575;
t4580 = -t4576;
t4585 = t3543.*t3980.*1.02e-6;
t4589 = t3980.*(t1896-t3239).*(-5.7e-7);
t4591 = t3980.*(t1896-t3239).*(-1.02e-6);
t4594 = t3543.*t3980.*2.4e-7;
t4596 = t3543.*t3980.*4.0e-8;
t4598 = t3980.*(t1896-t3239).*(-2.4e-7);
t4599 = t3980.*(t1896-t3239).*(-4.0e-8);
t4602 = t17.*t3980.*(t1896-t3239).*(-9.3e-7);
t4605 = t3547.*t3991.*5.7e-7;
t4606 = t3547.*t3991.*1.02e-6;
t4608 = t12.*t3980.*(t1896-t3239).*(-9.0e-8);
t4609 = t17.*t3980.*(t1896-t3239).*(-9.0e-8);
t4612 = t3550.*t3991.*1.02e-6;
t4613 = t21.*t3980.*(t1896-t3239).*1.02e-6;
t4614 = t3547.*t3991.*2.4e-7;
t4615 = t3547.*t3991.*4.0e-8;
t4618 = t17.*t3547.*t3991.*9.3e-7;
t4623 = t3550.*t3991.*2.4e-7;
t4625 = t3550.*t3991.*4.0e-8;
t4626 = t12.*t3547.*t3991.*(-1.02e-6);
t4634 = t12.*t3547.*t3991.*9.0e-8;
t4635 = t17.*t3547.*t3991.*9.0e-8;
t4647 = -t4026.*(t335-t1539-t2831+t2851);
t4649 = t11.*t3502.*t4026.*1.02e-6;
t4685 = -t4681;
t4686 = t3815.*t4026;
t4690 = t3819.*t4026;
t4712 = t2310+t3301+t3615+t3623;
t4718 = t3872.*t4026;
t4733 = t3893.*t4026;
t4766 = t3980.*(t2694-t2701+t3036-t3043).*(-1.0e-8);
t4767 = t3980.*(t1959-t3313+t38.*t1022.*(t855-t878).*2.196325630278387e-1).*(-1.0e-8);
t4768 = (t3934.*t3991)./1.0e+8;
t4769 = (t3937.*t3991)./1.0e+8;
t4775 = t2769+t3424+t3731+t3745;
t4780 = t3980.*(t2694-t2701+t3036-t3043).*(-5.7e-7);
t4781 = t3980.*(t2694-t2701+t3036-t3043).*(-1.02e-6);
t4783 = t3980.*(t2694-t2701+t3036-t3043).*5.7e-7;
t4784 = t3980.*(t2694-t2701+t3036-t3043).*1.02e-6;
t4785 = t3980.*(t2694-t2701+t3036-t3043).*(-2.4e-7);
t4787 = t3980.*(t2694-t2701+t3036-t3043).*(-4.0e-8);
t4789 = t17.*t3980.*(t2694-t2701+t3036-t3043).*(-9.3e-7);
t4791 = t3934.*t3991.*5.7e-7;
t4792 = t3934.*t3991.*1.02e-6;
t4793 = t3980.*(t1959-t3313+t38.*t1022.*(t855-t878).*2.196325630278387e-1).*(-1.02e-6);
t4794 = t3937.*t3991.*1.02e-6;
t4795 = t3980.*(t2694-t2701+t3036-t3043).*4.0e-8;
t4796 = t3980.*(t1959-t3313+t38.*t1022.*(t855-t878).*2.196325630278387e-1).*(-2.4e-7);
t4798 = t17.*t3980.*(t2694-t2701+t3036-t3043).*9.3e-7;
t4799 = t3934.*t3991.*2.4e-7;
t4801 = t3934.*t3991.*4.0e-8;
t4802 = t12.*t3980.*(t2694-t2701+t3036-t3043).*(-9.0e-8);
t4803 = t3937.*t3991.*2.4e-7;
t4804 = t17.*t3980.*(t2694-t2701+t3036-t3043).*(-9.0e-8);
t4806 = t17.*t3934.*t3991.*9.3e-7;
t4807 = t3980.*(t1959-t3313+t38.*t1022.*(t855-t878).*2.196325630278387e-1).*(-4.0e-8);
t4812 = t12.*t3980.*(t2694-t2701+t3036-t3043).*9.0e-8;
t4815 = t17.*t3980.*(t2694-t2701+t3036-t3043).*9.0e-8;
t4816 = t3980.*(t1959-t3313+t38.*t1022.*(t855-t878).*2.196325630278387e-1).*4.0e-8;
t4818 = t3937.*t3991.*4.0e-8;
t4824 = t12.*t3934.*t3991.*9.0e-8;
t4825 = t17.*t3934.*t3991.*9.0e-8;
t4855 = t3236.*(t3985+t12.*(t1861-t3221)).*(-9.3e-7);
t4856 = t3236.*(t3985+t12.*(t1861-t3221)).*(-1.02e-6);
t4857 = t3236.*(t3985+t12.*(t1861-t3221)).*9.3e-7;
t4858 = t3236.*(t3985+t12.*(t1861-t3221)).*(-9.0e-8);
t4859 = t3236.*(t3985+t12.*(t1861-t3221)).*9.0e-8;
t4876 = t3980.*t4019.*1.02e-6;
t4883 = t3980.*(t3242-t3554).*(-1.02e-6);
t4887 = t3980.*(t3242-t3554).*1.02e-6;
t4889 = t17.*t3980.*(t3242-t3554).*(-9.3e-7);
t4898 = t17.*t3980.*(t3242-t3554).*(-9.0e-8);
t4899 = t3991.*t4026.*1.02e-6;
t4901 = t12.*t3980.*(t3242-t3554).*(-9.0e-8);
t4904 = t17.*t3991.*t4026.*9.3e-7;
t4907 = t12.*t3991.*t4026.*(-1.02e-6);
t4911 = t17.*t3991.*t4026.*9.0e-8;
t4912 = t12.*t3991.*t4026.*9.0e-8;
t4918 = t4897.*9.99471e-3;
t4919 = t4896.*1.838876e-2;
t4921 = t3980.*(t1005+t20.*(t1941-t3315+t39.*t1022.*(t855-t878).*2.196325630278387e-1)).*(-1.0e-8);
t4922 = (t3991.*t4151)./1.0e+8;
t4931 = -t22.*t4026.*(t2813-t2835+t12.*(t1456-t2355).*1.02e-6+t17.*(t1456-t2355).*9.0e-8);
t4932 = -t28.*t4026.*(-t2804+t2838+t3109+t17.*(t1456-t2355).*9.3e-7);
t4934 = t3980.*(t1005+t20.*(t1941-t3315+t39.*t1022.*(t855-t878).*2.196325630278387e-1)).*(-1.02e-6);
t4935 = t22.*t4026.*(t2813-t2835+t12.*(t1456-t2355).*1.02e-6+t17.*(t1456-t2355).*9.0e-8);
t4936 = t28.*t4026.*(-t2804+t2838+t3109+t17.*(t1456-t2355).*9.3e-7);
t4938 = t3980.*(t1005+t20.*(t1941-t3315+t39.*t1022.*(t855-t878).*2.196325630278387e-1)).*(-2.4e-7);
t4940 = t3980.*(t1005+t20.*(t1941-t3315+t39.*t1022.*(t855-t878).*2.196325630278387e-1)).*(-4.0e-8);
t4941 = t3991.*t4151.*1.02e-6;
t4943 = t3991.*t4151.*2.4e-7;
t4945 = t4897.*7.26350557185e-5;
t4946 = t3991.*t4151.*4.0e-8;
t4947 = t4896.*1.33637554986e-4;
t4950 = t3293+t3295+t3625+t3627;
t4969 = t3543.*(t3985+t12.*(t1861-t3221)).*(-9.3e-7);
t4973 = (t3985+t12.*(t1861-t3221)).*(t1896-t3239).*9.3e-7;
t4974 = (t3985+t12.*(t1861-t3221)).*(t1896-t3239).*1.02e-6;
t4977 = t3543.*(t3985+t12.*(t1861-t3221)).*(-9.0e-8);
t4979 = (t3985+t12.*(t1861-t3221)).*(t1896-t3239).*9.0e-8;
t5026 = t3410+t3414+t3740+t3744;
t5040 = t3064+t4061+t4069;
t5044 = t3080+t4087+t4102;
t5083 = t50.*t202.*t5042.*4.771516396025243e-17;
t5100 = t2388.*t5041;
t5101 = t2399.*t5041;
t5103 = (t2363.*t5041)./2.0;
t5106 = (t2363.*t5043)./2.0;
t5117 = (t3985+t12.*(t1861-t3221)).*(t2694-t2701+t3036-t3043).*9.3e-7;
t5118 = (t3985+t12.*(t1861-t3221)).*(t2694-t2701+t3036-t3043).*1.02e-6;
t5123 = (t3985+t12.*(t1861-t3221)).*(t1959-t3313+t38.*t1022.*(t855-t878).*2.196325630278387e-1).*9.3e-7;
t5124 = (t3985+t12.*(t1861-t3221)).*(t2694-t2701+t3036-t3043).*9.0e-8;
t5127 = (t3985+t12.*(t1861-t3221)).*(t1959-t3313+t38.*t1022.*(t855-t878).*2.196325630278387e-1).*9.0e-8;
t5141 = t3865+t3868+t3930;
t5155 = t4019.*(t3985+t12.*(t1861-t3221)).*(-9.3e-7);
t5158 = t4019.*(t3985+t12.*(t1861-t3221)).*9.3e-7;
t5161 = t4019.*(t3985+t12.*(t1861-t3221)).*(-9.0e-8);
t5163 = (t3985+t12.*(t1861-t3221)).*(t3242-t3554).*9.3e-7;
t5164 = (t3985+t12.*(t1861-t3221)).*(t3242-t3554).*1.02e-6;
t5166 = t4019.*(t3985+t12.*(t1861-t3221)).*9.0e-8;
t5169 = (t3985+t12.*(t1861-t3221)).*(t3242-t3554).*9.0e-8;
t5204 = t56+t73+t5143;
t5208 = (t1005+t20.*(t1941-t3315+t39.*t1022.*(t855-t878).*2.196325630278387e-1)).*(t3985+t12.*(t1861-t3221)).*9.3e-7;
t5212 = (t1005+t20.*(t1941-t3315+t39.*t1022.*(t855-t878).*2.196325630278387e-1)).*(t3985+t12.*(t1861-t3221)).*9.0e-8;
t5243 = t3236.*t5042;
t5244 = t3237.*t5042;
t5249 = -t5248;
t5259 = -t5258;
t5264 = t3543.*t5041;
t5265 = -t5041.*(t1896-t3239);
t5266 = t3547.*t5041;
t5268 = t3550.*t5041;
t5269 = t5041.*(t1896-t3239);
t5271 = -t5043.*(t1896-t3239);
t5272 = t3547.*t5043;
t5273 = t3530+t3591+t3601+t3616+t3619;
t5314 = t4026.*(t11.*((t237.*(t42-t43))./9.007199254740992e+15+t15.*(-t1881+t3121+t3276))+t16.*(-t1901+t3122+t3277)).*(-1.02e-6);
t5316 = t4026.*(t11.*((t237.*(t42-t43))./9.007199254740992e+15+t15.*(-t1881+t3121+t3276))+t16.*(-t1901+t3122+t3277)).*1.02e-6;
t5322 = t3991.*t4872.*1.02e-6;
t5324 = t3980.*(t4165+t27.*(t1959-t3313+t38.*t1022.*(t855-t878).*2.196325630278387e-1)).*(-1.02e-6);
t5325 = (t3991.*t4915)./1.0e+8;
t5327 = (t3980.*t4920)./1.0e+8;
t5329 = t3991.*t4915.*1.02e-6;
t5330 = t3980.*t4920.*1.02e-6;
t5331 = t3991.*t4915.*2.4e-7;
t5336 = t3980.*t4920.*2.4e-7;
t5337 = t3991.*t4915.*4.0e-8;
t5340 = t3980.*t4920.*4.0e-8;
t5348 = t4169+t4897;
t5351 = t4178+t4896;
t5360 = t321+t343+t5307;
t5368 = t3676+t3717+t3724+t3748+t3750;
t5374 = t50.*t202.*t5352.*4.771516396025243e-17;
t5383 = (t2363.*t5346)./2.0;
t5384 = (t2388.*t5345)./2.0;
t5387 = (t2399.*t5346)./2.0;
t5389 = (t2363.*t5353)./2.0;
t5411 = -t4026.*(-t3080+t4100+t11.*t3236.*(t1861-t3221).*1.02e-6);
t5412 = t4026.*(-t3080+t4100+t11.*t3236.*(t1861-t3221).*1.02e-6);
t5419 = t3055.*t5354;
t5424 = t5041.*(t3941-(t262.*(t46-t47))./9.007199254740992e+15);
t5425 = t4149.*t5041;
t5440 = t3236.*t5318.*1.02e-6;
t5441 = t3236.*t5318.*9.0e-8;
t5461 = t3236.*t5352;
t5462 = t3237.*t5352;
t5465 = t635+t636+t679+t689+t1587+t1606+t1608+t1609+t2295+t3279+t3285+t3297+t3596+t3603;
t5472 = (t4165+t27.*(t1959-t3313+t38.*t1022.*(t855-t878).*2.196325630278387e-1)).*(t3985+t12.*(t1861-t3221)).*9.3e-7;
t5474 = (t4165+t27.*(t1959-t3313+t38.*t1022.*(t855-t878).*2.196325630278387e-1)).*(t3985+t12.*(t1861-t3221)).*9.0e-8;
t5500 = t5318.*(t1896-t3239).*(-1.02e-6);
t5501 = t5318.*(t1896-t3239).*1.02e-6;
t5503 = t5318.*(t1896-t3239).*(-9.0e-8);
t5506 = t5318.*(t1896-t3239).*9.0e-8;
t5507 = -t5504;
t5509 = t4920.*(t3985+t12.*(t1861-t3221)).*(-9.3e-7);
t5512 = -t5510;
t5514 = t4920.*(t3985+t12.*(t1861-t3221)).*(-9.0e-8);
t5522 = t3543.*t5345;
t5523 = t3543.*t5346;
t5524 = -t5346.*(t1896-t3239);
